simulink model "LKAS_AutoSave_20210315_1628"  (R2018b)
(part 1 of 18)
settings: Solver=FixedStepDiscrete  StartTime=0.0  StopTime=10.0  FixedStep=0.01  RelTol=1e-3
InitFcn:
  | tmpVer = ver('MATLAB');
  | tmpVer = str2num(tmpVer.Version);
  | % -------------------------------------------------------------------
  | %  MATLAB file generated by Simulink.saveVars on 21-Nov-2019 10:06:14
  | %  MATLAB version: 7.13.0.564 (R2011b)
  | % -------------------------------------------------------------------
  | 
  | 
  | SInt16 = Simulink.AliasType;
  | SInt16.Description = 'Num';
  | if (tmpVer > 7.11)
  | 	SInt16.DataScope = 'Auto';
  | end
  | SInt16.HeaderFile = 'Rte_Type.h';
  | SInt16.BaseType = 'int16';
  | 
  | SInt32 = Simulink.AliasType;
  | SInt32.Description = 'Num';
  | if (tmpVer > 7.11)
  | 	SInt32.DataScope = 'Auto';
  | end
  | SInt32.HeaderFile = 'Rte_Type.h';
  | SInt32.BaseType = 'int32';
  | 
  | SInt8 = Simulink.AliasType;
  | SInt8.Description = 'Num';
  | if (tmpVer > 7.11)
  | 	SInt8.DataScope = 'Auto';
  | end
  | SInt8.HeaderFile = 'Rte_Type.h';
  | SInt8.BaseType = 'int8';
  | 
  | T_A_m2_1024_1_u32 = Simulink.NumericType;
  | T_A_m2_1024_1_u32.Description = 'm2 (square meters  (m2))';
  | if (tmpVer > 7.11)
  | 	T_A_m2_1024_1_u32.DataScope = 'Auto';
  | end
  | T_A_m2_1024_1_u32.HeaderFile = 'Rte_Type.h';
  | T_A_m2_1024_1_u32.DataTypeMode = 'Fixed-point: slope and bias scaling';
  | T_A_m2_1024_1_u32.SignednessBool = false;
  | T_A_m2_1024_1_u32.WordLength = 32;
  | T_A_m2_1024_1_u32.FixedExponent = -10;
  | T_A_m2_1024_1_u32.SlopeAdjustmentFactor = 1;
  | T_A_m2_1024_1_u32.Bias = 0;
  | T_A_m2_1024_1_u32.DataTypeOverride = 'Inherit';
  | T_A_m2_1024_1_u32.IsAlias = true;
  | 
  | T_A_m2_65536_1_u16 = Simulink.NumericType;
  | T_A_m2_65536_1_u16.Description = 'm2 (square meters  (m2))';
  | if (tmpVer > 7.11)
  | 	T_A_m2_65536_1_u16.DataScope = 'Auto';
  | end
  | T_A_m2_65536_1_u16.HeaderFile = 'Rte_Type.h';
  | T_A_m2_65536_1_u16.DataTypeMode = 'Fixed-point: slope and bias scaling';
  | T_A_m2_65536_1_u16.SignednessBool = false;
  | T_A_m2_65536_1_u16.WordLength = 16;
  | T_A_m2_65536_1_u16.FixedExponent = -16;
  | T_A_m2_65536_1_u16.SlopeAdjustmentFactor = 1;
  | T_A_m2_65536_1_u16.Bias = 0;
  | T_A_m2_65536_1_u16.DataTypeOverride = 'Inherit';
  | T_A_m2_65536_1_u16.IsAlias = true;
  | 
  | T_A_m2_Float32 = Simulink.NumericType;
  | T_A_m2_Float32.Description = 'm2 (square meters  (m2))';
  | if (tmpVer > 7.11)
  | 	T_A_m2_Float32.DataScope = 'Auto';
  | end
  | T_A_m2_Float32.HeaderFile = 'Rte_Type.h';
  | T_A_m2_Float32.DataTypeMode = 'Single';
  | T_A_m2_Float32.SignednessBool = true;
  | T_A_m2_Float32.WordLength = 32;
  | T_A_m2_Float32.FixedExponent = 0;
  | T_A_m2_Float32.SlopeAdjustmentFactor = 1;
  | T_A_m2_Float32.Bias = 0;
  | T_A_m2_Float32.DataTypeOverride = 'Inherit';
  | T_A_m2_Float32.IsAlias = true;
  | 
  | T_A_mm2_10_1_u16 = Simulink.NumericType;
  | T_A_mm2_10_1_u16.Description = 'mm2 (square millimeters  (mm2))';
  | if (tmpVer > 7.11)
  | 	T_A_mm2_10_1_u16.DataScope = 'Auto';
  | end
  | T_A_mm2_10_1_u16.HeaderFile = 'Rte_Type.h';
  | T_A_mm2_10_1_u16.DataTypeMode = 'Fixed-point: slope and bias scaling';
  | T_A_mm2_10_1_u16.SignednessBool = false;
  | T_A_mm2_10_1_u16.WordLength = 16;
  | T_A_mm2_10_1_u16.FixedExponent = -4;
  | T_A_mm2_10_1_u16.SlopeAdjustmentFactor = 1.6;
  | T_A_mm2_10_1_u16.Bias = 0;
  | T_A_mm2_10_1_u16.DataTypeOverride = 'Inherit';
  | T_A_mm2_10_1_u16.IsAlias = true;
  | 
  | T_A_mm2_4_1_s16 = Simulink.NumericType;
  | T_A_mm2_4_1_s16.Description = 'mm2 (square millimeters  (mm2))';
  | if (tmpVer > 7.11)
  | 	T_A_mm2_4_1_s16.DataScope = 'Auto';
  | end
  | T_A_mm2_4_1_s16.HeaderFile = 'Rte_Type.h';
  | T_A_mm2_4_1_s16.DataTypeMode = 'Fixed-point: slope and bias scaling';
  | T_A_mm2_4_1_s16.SignednessBool = true;
  | T_A_mm2_4_1_s16.WordLength = 16;
  | T_A_mm2_4_1_s16.FixedExponent = -2;
  | T_A_mm2_4_1_s16.SlopeAdjustmentFactor = 1;
  | T_A_mm2_4_1_s16.Bias = 0;
  | T_A_mm2_4_1_s16.DataTypeOverride = 'Inherit';
  | T_A_mm2_4_1_s16.IsAlias = true;
  | 
  | T_A_mm2_Float32 = Simulink.NumericType;
  | T_A_mm2_Float32.Description = 'mm2 (square millimeters  (mm2))';
  | if (tmpVer > 7.11)
  | 	T_A_mm2_Float32.DataScope = 'Auto';
  | end
  | T_A_mm2_Float32.HeaderFile = 'Rte_Type.h';
  | T_A_mm2_Float32.DataTypeMode = 'Single';
  | T_A_mm2_Float32.SignednessBool = true;
  | T_A_mm2_Float32.WordLength = 32;
  | T_A_mm2_Float32.FixedExponent = 0;
  | T_A_mm2_Float32.SlopeAdjustmentFactor = 1;
  | T_A_mm2_Float32.Bias = 0;
  | T_A_mm2_Float32.DataTypeOverride = 'Inherit';
  | T_A_mm2_Float32.IsAlias = true;
  | 
  | T_BOOLEAN = Simulink.AliasType;
  | T_BOOLEAN.Description = 'Bool';
  | if (tmpVer > 7.11)
  | 	T_BOOLEAN.DataScope = 'Auto';
  | end
  | T_BOOLEAN.HeaderFile = 'Rte_Type.h';
  | T_BOOLEAN.BaseType = 'boolean';
  | 
  | T_Cnt_Num_10_1_u32 = Simulink.NumericType;
  | T_Cnt_Num_10_1_u32.Description = 'Num (counts)';
  | if (tmpVer > 7.11)
  | 	T_Cnt_Num_10_1_u32.DataScope = 'Auto';
  | end
  | T_Cnt_Num_10_1_u32.HeaderFile = 'Rte_Type.h';
  | T_Cnt_Num_10_1_u32.DataTypeMode = 'Fixed-point: slope and bias scaling';
  | T_Cnt_Num_10_1_u32.SignednessBool = false;
  | T_Cnt_Num_10_1_u32.WordLength = 32;
  | T_Cnt_Num_10_1_u32.FixedExponent = -4;
  | T_Cnt_Num_10_1_u32.SlopeAdjustmentFactor = 1.6;
  | T_Cnt_Num_10_1_u32.Bias = 0;
  | T_Cnt_Num_10_1_u32.DataTypeOverride = 'Inherit';
  | T_Cnt_Num_10_1_u32.IsAlias = true;
  | 
  | T_Cnt_Num_1_1_s16 = Simulink.NumericType;
  | T_Cnt_Num_1_1_s16.Description = 'Num (counts)';
  | if (tmpVer > 7.11)
  | 	T_Cnt_Num_1_1_s16.DataScope = 'Auto';
  | end
  | T_Cnt_Num_1_1_s16.HeaderFile = 'Rte_Type.h';
  | T_Cnt_Num_1_1_s16.DataTypeMode = 'Fixed-point: slope and bias scaling';
  | T_Cnt_Num_1_1_s16.SignednessBool = true;
  | T_Cnt_Num_1_1_s16.WordLength = 16;
  | T_Cnt_Num_1_1_s16.FixedExponent = 0;
  | T_Cnt_Num_1_1_s16.SlopeAdjustmentFactor = 1;
  | T_Cnt_Num_1_1_s16.Bias = 0;
  | T_Cnt_Num_1_1_s16.DataTypeOverride = 'Inherit';
  | T_Cnt_Num_1_1_s16.IsAlias = true;
  | 
  | T_Cnt_Num_1_1_s32 = Simulink.NumericType;
  | T_Cnt_Num_1_1_s32.Description = 'Num (counts)';
  | if (tmpVer > 7.11)
  | 	T_Cnt_Num_1_1_s32.DataScope = 'Auto';
  | end
  | T_Cnt_Num_1_1_s32.HeaderFile = 'Rte_Type.h';
  | T_Cnt_Num_1_1_s32.DataTypeMode = 'Fixed-point: slope and bias scaling';
  | T_Cnt_Num_1_1_s32.SignednessBool = true;
  | T_Cnt_Num_1_1_s32.WordLength = 32;
  | T_Cnt_Num_1_1_s32.FixedExponent = 0;
  | T_Cnt_Num_1_1_s32.SlopeAdjustmentFactor = 1;
  | T_Cnt_Num_1_1_s32.Bias = 0;
  | T_Cnt_Num_1_1_s32.DataTypeOverride = 'Inherit';
  | T_Cnt_Num_1_1_s32.IsAlias = true;
  | 
  | T_Cnt_Num_1_1_s8 = Simulink.NumericType;
  | T_Cnt_Num_1_1_s8.Description = 'Num (counts)';
  | if (tmpVer > 7.11)
  | 	T_Cnt_Num_1_1_s8.DataScope = 'Auto';
  | end
  | T_Cnt_Num_1_1_s8.HeaderFile = 'Rte_Type.h';
  | T_Cnt_Num_1_1_s8.DataTypeMode = 'Fixed-point: slope and bias scaling';
  | T_Cnt_Num_1_1_s8.SignednessBool = true;
  | T_Cnt_Num_1_1_s8.WordLength = 8;
  | T_Cnt_Num_1_1_s8.FixedExponent = 0;
  | T_Cnt_Num_1_1_s8.SlopeAdjustmentFactor = 1;
  | T_Cnt_Num_1_1_s8.Bias = 0;
  | T_Cnt_Num_1_1_s8.DataTypeOverride = 'Inherit';
  | T_Cnt_Num_1_1_s8.IsAlias = true;
  | 
  | T_Cnt_Num_1_1_u16 = Simulink.NumericType;
  | T_Cnt_Num_1_1_u16.Description = 'Num (counts)';
  | if (tmpVer > 7.11)
  | 	T_Cnt_Num_1_1_u16.DataScope = 'Auto';
  | end
  | T_Cnt_Num_1_1_u16.HeaderFile = 'Rte_Type.h';
  | T_Cnt_Num_1_1_u16.DataTypeMode = 'Fixed-point: slope and bias scaling';
  | T_Cnt_Num_1_1_u16.SignednessBool = false;
  | T_Cnt_Num_1_1_u16.WordLength = 16;
  | T_Cnt_Num_1_1_u16.FixedExponent = 0;
  | T_Cnt_Num_1_1_u16.SlopeAdjustmentFactor = 1;
  | T_Cnt_Num_1_1_u16.Bias = 0;
  | T_Cnt_Num_1_1_u16.DataTypeOverride = 'Inherit';
  | T_Cnt_Num_1_1_u16.IsAlias = true;
  | 
  | T_Cnt_Num_1_1_u32 = Simulink.NumericType;
  | T_Cnt_Num_1_1_u32.Description = 'Num (counts)';
  | if (tmpVer > 7.11)
  | 	T_Cnt_Num_1_1_u32.DataScope = 'Auto';
  | end
  | T_Cnt_Num_1_1_u32.HeaderFile = 'Rte_Type.h';
  | T_Cnt_Num_1_1_u32.DataTypeMode = 'Fixed-point: slope and bias scaling';
  | T_Cnt_Num_1_1_u32.SignednessBool = false;
  | T_Cnt_Num_1_1_u32.WordLength = 32;
  | T_Cnt_Num_1_1_u32.FixedExponent = 0;
  | T_Cnt_Num_1_1_u32.SlopeAdjustmentFactor = 1;
  | T_Cnt_Num_1_1_u32.Bias = 0;
  | T_Cnt_Num_1_1_u32.DataTypeOverride = 'Inherit';
  | T_Cnt_Num_1_1_u32.IsAlias = true;
  | 
  | T_Cnt_Num_1_1_u8 = Simulink.NumericType;
  | T_Cnt_Num_1_1_u8.Description = 'Num (counts)';
  | if (tmpVer > 7.11)
  | 	T_Cnt_Num_1_1_u8.DataScope = 'Auto';
  | end
  | T_Cnt_Num_1_1_u8.HeaderFile = 'Rte_Type.h';
  | T_Cnt_Num_1_1_u8.DataTypeMode = 'Fixed-point: slope and bias scaling';
  | T_Cnt_Num_1_1_u8.SignednessBool = false;
  | T_Cnt_Num_1_1_u8.WordLength = 8;
  | T_Cnt_Num_1_1_u8.FixedExponent = 0;
  | T_Cnt_Num_1_1_u8.SlopeAdjustmentFactor = 1;
  | T_Cnt_Num_1_1_u8.Bias = 0;
  | T_Cnt_Num_1_1_u8.DataTypeOverride = 'Inherit';
  | T_Cnt_Num_1_1_u8.IsAlias = true;
  | 
  | T_E_J_1_1_s32 = Simulink.NumericType;
  | T_E_J_1_1_s32.Description = 'J (joules  (J))';
  | if (tmpVer > 7.11)
  | 	T_E_J_1_1_s32.DataScope = 'Auto';
  | end
  | T_E_J_1_1_s32.HeaderFile = 'Rte_Type.h';
  | T_E_J_1_1_s32.DataTypeMode = 'Fixed-point: slope and bias scaling';
  | T_E_J_1_1_s32.SignednessBool = true;
  | T_E_J_1_1_s32.WordLength = 32;
  | T_E_J_1_1_s32.FixedExponent = 0;
  | T_E_J_1_1_s32.SlopeAdjustmentFactor = 1;
  | T_E_J_1_1_s32.Bias = 0;
  | T_E_J_1_1_s32.DataTypeOverride = 'Inherit';
  | T_E_J_1_1_s32.IsAlias = true;
  | 
  | T_E_J_Float32 = Simulink.NumericType;
  | T_E_J_Float32.Description = 'J (joules  (J))';
  | if (tmpVer > 7.11)
  | 	T_E_J_Float32.DataScope = 'Auto';
  | end
  | T_E_J_Float32.HeaderFile = 'Rte_Type.h';
  | T_E_J_Float32.DataTypeMode = 'Single';
  | T_E_J_Float32.SignednessBool = true;
  | T_E_J_Float32.WordLength = 32;
  | T_E_J_Float32.FixedExponent = 0;
  | T_E_J_Float32.SlopeAdjustmentFactor = 1;
  | T_E_J_Float32.Bias = 0;
  | T_E_J_Float32.DataTypeOverride = 'Inherit';
  | T_E_J_Float32.IsAlias = true;
  | 
  | T_E_kJ_128_1_s32 = Simulink.NumericType;
  | T_E_kJ_128_1_s32.Description = 'kJ (kilojoules  (kJ))';
  | if (tmpVer > 7.11)
  | 	T_E_kJ_128_1_s32.DataScope = 'Auto';
  | end
  | T_E_kJ_128_1_s32.HeaderFile = 'Rte_Type.h';
  | T_E_kJ_128_1_s32.DataTypeMode = 'Fixed-point: slope and bias scaling';
  | T_E_kJ_128_1_s32.SignednessBool = true;
  | T_E_kJ_128_1_s32.WordLength = 32;
  | T_E_kJ_128_1_s32.FixedExponent = -7;
  | T_E_kJ_128_1_s32.SlopeAdjustmentFactor = 1;
  | T_E_kJ_128_1_s32.Bias = 0;
  | T_E_kJ_128_1_s32.DataTypeOverride = 'Inherit';
  | T_E_kJ_128_1_s32.IsAlias = true;
  | 
  | T_E_kJ_Float32 = Simulink.NumericType;
  | T_E_kJ_Float32.Description = 'kJ (kilojoules  (kJ))';
  | if (tmpVer > 7.11)
  | 	T_E_kJ_Float32.DataScope = 'Auto';
  | end
  | T_E_kJ_Float32.HeaderFile = 'Rte_Type.h';
  | T_E_kJ_Float32.DataTypeMode = 'Single';
  | T_E_kJ_Float32.SignednessBool = true;
  | T_E_kJ_Float32.WordLength = 32;
  | T_E_kJ_Float32.FixedExponent = 0;
  | T_E_kJ_Float32.SlopeAdjustmentFactor = 1;
  | T_E_kJ_Float32.Bias = 0;
  | T_E_kJ_Float32.DataTypeOverride = 'Inherit';
  | T_E_kJ_Float32.IsAlias = true;
  | 
  | T_E_kwh_10_1_u16 = Simulink.NumericType;
  | T_E_kwh_10_1_u16.Description = 'kwh (kilowatt-hours (kwh))';
  | if (tmpVer > 7.11)
  | 	T_E_kwh_10_1_u16.DataScope = 'Auto';
  | end
  | T_E_kwh_10_1_u16.HeaderFile = 'Rte_Type.h';
  | T_E_kwh_10_1_u16.DataTypeMode = 'Fixed-point: slope and bias scaling';
  | T_E_kwh_10_1_u16.SignednessBool = false;
  | T_E_kwh_10_1_u16.WordLength = 16;
  | T_E_kwh_10_1_u16.FixedExponent = -4;
  | T_E_kwh_10_1_u16.SlopeAdjustmentFactor = 1.6;
  | T_E_kwh_10_1_u16.Bias = 0;
  | T_E_kwh_10_1_u16.DataTypeOverride = 'Inherit';
  | T_E_kwh_10_1_u16.IsAlias = true;
  | 
  | T_E_kwh_Float32 = Simulink.NumericType;
  | T_E_kwh_Float32.Description = 'kwh (kilowatt-hours (kwh))';
  | if (tmpVer > 7.11)
  | 	T_E_kwh_Float32.DataScope = 'Auto';
  | end
  | T_E_kwh_Float32.HeaderFile = 'Rte_Type.h';
  | T_E_kwh_Float32.DataTypeMode = 'Single';
  | T_E_kwh_Float32.SignednessBool = true;
  | T_E_kwh_Float32.WordLength = 32;
  | T_E_kwh_Float32.FixedExponent = 0;
  | T_E_kwh_Float32.SlopeAdjustmentFactor = 1;
  | T_E_kwh_Float32.Bias = 0;
  | T_E_kwh_Float32.DataTypeOverride = 'Inherit';
  | T_E_kwh_Float32.IsAlias = true;
  | 
  | T_Epl_kwhpkm_100_1_u16 = Simulink.NumericType;
  | T_Epl_kwhpkm_100_1_u16.Description = 'kwhpkm (kwh / 100km  (kwhpkm))';
  | if (tmpVer > 7.11)
  | 	T_Epl_kwhpkm_100_1_u16.DataScope = 'Auto';
  | end
  | T_Epl_kwhpkm_100_1_u16.HeaderFile = 'Rte_Type.h';
  | T_Epl_kwhpkm_100_1_u16.DataTypeMode = ...
  |   'Fixed-point: slope and bias scaling';
  | T_Epl_kwhpkm_100_1_u16.SignednessBool = false;
  | T_Epl_kwhpkm_100_1_u16.WordLength = 16;
  | T_Epl_kwhpkm_100_1_u16.FixedExponent = -7;
  | T_Epl_kwhpkm_100_1_u16.SlopeAdjustmentFactor = 1.28;
  | T_Epl_kwhpkm_100_1_u16.Bias = 0;
  | T_Epl_kwhpkm_100_1_u16.DataTypeOverride = 'Inherit';
  | T_Epl_kwhpkm_100_1_u16.IsAlias = true;
  | 
  | T_Epl_kwhpkm_Float32 = Simulink.NumericType;
  | T_Epl_kwhpkm_Float32.Description = 'kwhpkm (kwh / 100km  (kwhpkm))';
  | if (tmpVer > 7.11)
  | 	T_Epl_kwhpkm_Float32.DataScope = 'Auto';
  | end
  | T_Epl_kwhpkm_Float32.HeaderFile = 'Rte_Type.h';
  | T_Epl_kwhpkm_Float32.DataTypeMode = 'Single';
  | T_Epl_kwhpkm_Float32.SignednessBool = true;
  | T_Epl_kwhpkm_Float32.WordLength = 32;
  | T_Epl_kwhpkm_Float32.FixedExponent = 0;
  | T_Epl_kwhpkm_Float32.SlopeAdjustmentFactor = 1;
  | T_Epl_kwhpkm_Float32.Bias = 0;
  | T_Epl_kwhpkm_Float32.DataTypeOverride = 'Inherit';
  | T_Epl_kwhpkm_Float32.IsAlias = true;
  | 
  | T_F_N_1_1_s16 = Simulink.NumericType;
  | T_F_N_1_1_s16.Description = 'N (newtons  (N))';
  | if (tmpVer > 7.11)
  | 	T_F_N_1_1_s16.DataScope = 'Auto';
  | end
  | T_F_N_1_1_s16.HeaderFile = 'Rte_Type.h';
  | T_F_N_1_1_s16.DataTypeMode = 'Fixed-point: slope and bias scaling';
  | T_F_N_1_1_s16.SignednessBool = true;
  | T_F_N_1_1_s16.WordLength = 16;
  | T_F_N_1_1_s16.FixedExponent = 0;
  | T_F_N_1_1_s16.SlopeAdjustmentFactor = 1;
  | T_F_N_1_1_s16.Bias = 0;
  | T_F_N_1_1_s16.DataTypeOverride = 'Inherit';
  | T_F_N_1_1_s16.IsAlias = true;
  | 
  | T_F_N_Float32 = Simulink.NumericType;
  | T_F_N_Float32.Description = 'N (newtons  (N))';
  | if (tmpVer > 7.11)
  | 	T_F_N_Float32.DataScope = 'Auto';
  | end
  | T_F_N_Float32.HeaderFile = 'Rte_Type.h';
  | T_F_N_Float32.DataTypeMode = 'Single';
  | T_F_N_Float32.SignednessBool = true;
  | T_F_N_Float32.WordLength = 32;
  | T_F_N_Float32.FixedExponent = 0;
  | T_F_N_Float32.SlopeAdjustmentFactor = 1;
  | T_F_N_Float32.Bias = 0;
  | T_F_N_Float32.DataTypeOverride = 'Inherit';
  | T_F_N_Float32.IsAlias = true;
  | 
  | T_I_A_1000_1_u16 = Simulink.NumericType;
  | T_I_A_1000_1_u16.Description = 'A (amperes  (A))';
  | if (tmpVer > 7.11)
  | 	T_I_A_1000_1_u16.DataScope = 'Auto';
  | end
  | T_I_A_1000_1_u16.HeaderFile = 'Rte_Type.h';
  | T_I_A_1000_1_u16.DataTypeMode = 'Fixed-point: slope and bias scaling';
  | T_I_A_1000_1_u16.SignednessBool = false;
  | T_I_A_1000_1_u16.WordLength = 16;
  | T_I_A_1000_1_u16.FixedExponent = -10;
  | T_I_A_1000_1_u16.SlopeAdjustmentFactor = 1.024;
  | T_I_A_1000_1_u16.Bias = 0;
  | T_I_A_1000_1_u16.DataTypeOverride = 'Inherit';
  | T_I_A_1000_1_u16.IsAlias = true;
  | 
  | T_I_A_1048576_1_s32 = Simulink.NumericType;
  | T_I_A_1048576_1_s32.Description = 'A (amperes  (A))';
  | if (tmpVer > 7.11)
  | 	T_I_A_1048576_1_s32.DataScope = 'Auto';
  | end
  | T_I_A_1048576_1_s32.HeaderFile = 'Rte_Type.h';
  | T_I_A_1048576_1_s32.DataTypeMode = ['Fixed-point: slope and bias scalin' ...
  |                                     'g'];
  | T_I_A_1048576_1_s32.SignednessBool = true;
  | T_I_A_1048576_1_s32.WordLength = 32;
  | T_I_A_1048576_1_s32.FixedExponent = -20;
  | T_I_A_1048576_1_s32.SlopeAdjustmentFactor = 1;
  | T_I_A_1048576_1_s32.Bias = 0;
  | T_I_A_1048576_1_s32.DataTypeOverride = 'Inherit';
  | T_I_A_1048576_1_s32.IsAlias = true;
  | 
  | T_I_A_2048_1_s16 = Simulink.NumericType;
  | T_I_A_2048_1_s16.Description = 'A (amperes  (A))';
  | if (tmpVer > 7.11)
  | 	T_I_A_2048_1_s16.DataScope = 'Auto';
  | end
  | T_I_A_2048_1_s16.HeaderFile = 'Rte_Type.h';
  | T_I_A_2048_1_s16.DataTypeMode = 'Fixed-point: slope and bias scaling';
  | T_I_A_2048_1_s16.SignednessBool = true;
  | T_I_A_2048_1_s16.WordLength = 16;
  | T_I_A_2048_1_s16.FixedExponent = -11;
  | T_I_A_2048_1_s16.SlopeAdjustmentFactor = 1;
  | T_I_A_2048_1_s16.Bias = 0;
  | T_I_A_2048_1_s16.DataTypeOverride = 'Inherit';
  | T_I_A_2048_1_s16.IsAlias = true;
  | 
  | T_I_A_32_1_s16 = Simulink.NumericType;
  | T_I_A_32_1_s16.Description = 'A (amperes  (A))';
  | if (tmpVer > 7.11)
  | 	T_I_A_32_1_s16.DataScope = 'Auto';
  | end
  | T_I_A_32_1_s16.HeaderFile = 'Rte_Type.h';
  | T_I_A_32_1_s16.DataTypeMode = 'Fixed-point: slope and bias scaling';
  | T_I_A_32_1_s16.SignednessBool = true;
  | T_I_A_32_1_s16.WordLength = 16;
  | T_I_A_32_1_s16.FixedExponent = -5;
  | T_I_A_32_1_s16.SlopeAdjustmentFactor = 1;
  | T_I_A_32_1_s16.Bias = 0;
  | T_I_A_32_1_s16.DataTypeOverride = 'Inherit';
  | T_I_A_32_1_s16.IsAlias = true;
  | 
  | T_I_A_Float32 = Simulink.NumericType;
  | T_I_A_Float32.Description = 'A (amperes  (A))';
  | if (tmpVer > 7.11)
  | 	T_I_A_Float32.DataScope = 'Auto';
  | end
  | T_I_A_Float32.HeaderFile = 'Rte_Type.h';
  | T_I_A_Float32.DataTypeMode = 'Single';
  | T_I_A_Float32.SignednessBool = true;
  | T_I_A_Float32.WordLength = 32;
  | T_I_A_Float32.FixedExponent = 0;
  | T_I_A_Float32.SlopeAdjustmentFactor = 1;
  | T_I_A_Float32.Bias = 0;
  | T_I_A_Float32.DataTypeOverride = 'Inherit';
  | T_I_A_Float32.IsAlias = true;
  | 
  | T_I_mA_1_1_s16 = Simulink.NumericType;
  | T_I_mA_1_1_s16.Description = 'mA (milliamperes  (mA))';
  | if (tmpVer > 7.11)
  | 	T_I_mA_1_1_s16.DataScope = 'Auto';
  | end
  | T_I_mA_1_1_s16.HeaderFile = 'Rte_Type.h';
  | T_I_mA_1_1_s16.DataTypeMode = 'Fixed-point: slope and bias scaling';
  | T_I_mA_1_1_s16.SignednessBool = true;
  | T_I_mA_1_1_s16.WordLength = 16;
  | T_I_mA_1_1_s16.FixedExponent = 0;
  | T_I_mA_1_1_s16.SlopeAdjustmentFactor = 1;
  | T_I_mA_1_1_s16.Bias = 0;
  | T_I_mA_1_1_s16.DataTypeOverride = 'Inherit';
  | T_I_mA_1_1_s16.IsAlias = true;
  | 
  | T_I_mA_32768_128_s16 = Simulink.NumericType;
  | T_I_mA_32768_128_s16.Description = 'mA (milliamperes  (mA))';
  | if (tmpVer > 7.11)
  | 	T_I_mA_32768_128_s16.DataScope = 'Auto';
  | end
  | T_I_mA_32768_128_s16.HeaderFile = 'Rte_Type.h';
  | T_I_mA_32768_128_s16.DataTypeMode = ...
  |   'Fixed-point: slope and bias scaling';
  | T_I_mA_32768_128_s16.SignednessBool = true;
  | T_I_mA_32768_128_s16.WordLength = 16;
  | T_I_mA_32768_128_s16.FixedExponent = -8;
  | T_I_mA_32768_128_s16.SlopeAdjustmentFactor = 1;
  | T_I_mA_32768_128_s16.Bias = 0;
  | T_I_mA_32768_128_s16.DataTypeOverride = 'Inherit';
  | T_I_mA_32768_128_s16.IsAlias = true;
  | 
  | T_I_mA_Float32 = Simulink.NumericType;
  | T_I_mA_Float32.Description = 'mA (milliamperes  (mA))';
  | if (tmpVer > 7.11)
  | 	T_I_mA_Float32.DataScope = 'Auto';
  | end
  | T_I_mA_Float32.HeaderFile = 'Rte_Type.h';
  | T_I_mA_Float32.DataTypeMode = 'Single';
  | T_I_mA_Float32.SignednessBool = true;
  | T_I_mA_Float32.WordLength = 32;
  | T_I_mA_Float32.FixedExponent = 0;
  | T_I_mA_Float32.SlopeAdjustmentFactor = 1;
  | T_I_mA_Float32.Bias = 0;
  | T_I_mA_Float32.DataTypeOverride = 'Inherit';
  | T_I_mA_Float32.IsAlias = true;
  | 
  | T_J_kgpm2_128_1_u16 = Simulink.NumericType;
  | T_J_kgpm2_128_1_u16.Description = ['kgpm2 (kilograms-square meters  (kg' ...
  |                                    ' m2))'];
  | if (tmpVer > 7.11)
  | 	T_J_kgpm2_128_1_u16.DataScope = 'Auto';
  | end
  | T_J_kgpm2_128_1_u16.HeaderFile = 'Rte_Type.h';
  | T_J_kgpm2_128_1_u16.DataTypeMode = ['Fixed-point: slope and bias scalin' ...
  |                                     'g'];
  | T_J_kgpm2_128_1_u16.SignednessBool = false;
  | T_J_kgpm2_128_1_u16.WordLength = 16;
  | T_J_kgpm2_128_1_u16.FixedExponent = -7;
  | T_J_kgpm2_128_1_u16.SlopeAdjustmentFactor = 1;
  | T_J_kgpm2_128_1_u16.Bias = 0;
  | T_J_kgpm2_128_1_u16.DataTypeOverride = 'Inherit';
  | T_J_kgpm2_128_1_u16.IsAlias = true;
  | 
  | T_J_kgpm2_Float32 = Simulink.NumericType;
  | T_J_kgpm2_Float32.Description = ['kgpm2 (kilograms-square meters  (kg m' ...
  |                                  '2))'];
  | if (tmpVer > 7.11)
  | 	T_J_kgpm2_Float32.DataScope = 'Auto';
  | end
  | T_J_kgpm2_Float32.HeaderFile = 'Rte_Type.h';
  | T_J_kgpm2_Float32.DataTypeMode = 'Single';
  | T_J_kgpm2_Float32.SignednessBool = true;
  | T_J_kgpm2_Float32.WordLength = 32;
  | T_J_kgpm2_Float32.FixedExponent = 0;
  | T_J_kgpm2_Float32.SlopeAdjustmentFactor = 1;
  | T_J_kgpm2_Float32.Bias = 0;
  | T_J_kgpm2_Float32.DataTypeOverride = 'Inherit';
  | T_J_kgpm2_Float32.IsAlias = true;
  | 
  | T_K_NA_1000_1_s16 = Simulink.NumericType;
  | T_K_NA_1000_1_s16.Description = 'NA (dependent upon the gain)';
  | if (tmpVer > 7.11)
  | 	T_K_NA_1000_1_s16.DataScope = 'Auto';
  | end
  | T_K_NA_1000_1_s16.HeaderFile = 'Rte_Type.h';
  | T_K_NA_1000_1_s16.DataTypeMode = 'Fixed-point: slope and bias scaling';
  | T_K_NA_1000_1_s16.SignednessBool = true;
  | T_K_NA_1000_1_s16.WordLength = 16;
  | T_K_NA_1000_1_s16.FixedExponent = -10;
  | T_K_NA_1000_1_s16.SlopeAdjustmentFactor = 1.024;
  | T_K_NA_1000_1_s16.Bias = 0;
  | T_K_NA_1000_1_s16.DataTypeOverride = 'Inherit';
  | T_K_NA_1000_1_s16.IsAlias = true;
  | 
  | T_K_NA_100_1_s16 = Simulink.NumericType;
  | T_K_NA_100_1_s16.Description = 'NA (dependent upon the gain)';
  | if (tmpVer > 7.11)
  | 	T_K_NA_100_1_s16.DataScope = 'Auto';
  | end
  | T_K_NA_100_1_s16.HeaderFile = 'Rte_Type.h';
  | T_K_NA_100_1_s16.DataTypeMode = 'Fixed-point: slope and bias scaling';
  | T_K_NA_100_1_s16.SignednessBool = true;
  | T_K_NA_100_1_s16.WordLength = 16;
  | T_K_NA_100_1_s16.FixedExponent = -7;
  | T_K_NA_100_1_s16.SlopeAdjustmentFactor = 1.28;
  | T_K_NA_100_1_s16.Bias = 0;
  | T_K_NA_100_1_s16.DataTypeOverride = 'Inherit';
  | T_K_NA_100_1_s16.IsAlias = true;
  | 
  | T_K_NA_100_1_u16 = Simulink.NumericType;
  | T_K_NA_100_1_u16.Description = 'NA (dependent upon the gain)';
  | if (tmpVer > 7.11)
  | 	T_K_NA_100_1_u16.DataScope = 'Auto';
  | end
  | T_K_NA_100_1_u16.HeaderFile = 'Rte_Type.h';
  | T_K_NA_100_1_u16.DataTypeMode = 'Fixed-point: slope and bias scaling';
  | T_K_NA_100_1_u16.SignednessBool = false;
  | T_K_NA_100_1_u16.WordLength = 16;
  | T_K_NA_100_1_u16.FixedExponent = -7;
  | T_K_NA_100_1_u16.SlopeAdjustmentFactor = 1.28;
  | T_K_NA_100_1_u16.Bias = 0;
  | T_K_NA_100_1_u16.DataTypeOverride = 'Inherit';
  | T_K_NA_100_1_u16.IsAlias = true;
  | 
  | T_K_NA_1024_1_s16 = Simulink.NumericType;
  | T_K_NA_1024_1_s16.Description = 'NA (dependent upon the gain)';
  | if (tmpVer > 7.11)
  | 	T_K_NA_1024_1_s16.DataScope = 'Auto';
  | end
  | T_K_NA_1024_1_s16.HeaderFile = 'Rte_Type.h';
  | T_K_NA_1024_1_s16.DataTypeMode = 'Fixed-point: slope and bias scaling';
  | T_K_NA_1024_1_s16.SignednessBool = true;
  | T_K_NA_1024_1_s16.WordLength = 16;
  | T_K_NA_1024_1_s16.FixedExponent = -10;
  | T_K_NA_1024_1_s16.SlopeAdjustmentFactor = 1;
  | T_K_NA_1024_1_s16.Bias = 0;
  | T_K_NA_1024_1_s16.DataTypeOverride = 'Inherit';
  | T_K_NA_1024_1_s16.IsAlias = true;
  | 
  | T_K_NA_1024_1_u16 = Simulink.NumericType;
  | T_K_NA_1024_1_u16.Description = 'NA (dependent upon the gain)';
  | if (tmpVer > 7.11)
  | 	T_K_NA_1024_1_u16.DataScope = 'Auto';
  | end
  | T_K_NA_1024_1_u16.HeaderFile = 'Rte_Type.h';
  | T_K_NA_1024_1_u16.DataTypeMode = 'Fixed-point: slope and bias scaling';
  | T_K_NA_1024_1_u16.SignednessBool = false;
  | T_K_NA_1024_1_u16.WordLength = 16;
  | T_K_NA_1024_1_u16.FixedExponent = -10;
  | T_K_NA_1024_1_u16.SlopeAdjustmentFactor = 1;
  | T_K_NA_1024_1_u16.Bias = 0;
  | T_K_NA_1024_1_u16.DataTypeOverride = 'Inherit';
  | T_K_NA_1024_1_u16.IsAlias = true;
  | 
  | T_K_NA_128_1_s16 = Simulink.NumericType;
  | T_K_NA_128_1_s16.Description = 'NA (dependent upon the gain)';
  | if (tmpVer > 7.11)
  | 	T_K_NA_128_1_s16.DataScope = 'Auto';
  | end
  | T_K_NA_128_1_s16.HeaderFile = 'Rte_Type.h';
  | T_K_NA_128_1_s16.DataTypeMode = 'Fixed-point: slope and bias scaling';
  | T_K_NA_128_1_s16.SignednessBool = true;
  | T_K_NA_128_1_s16.WordLength = 16;
  | T_K_NA_128_1_s16.FixedExponent = -7;
  | T_K_NA_128_1_s16.SlopeAdjustmentFactor = 1;
  | T_K_NA_128_1_s16.Bias = 0;
  | T_K_NA_128_1_s16.DataTypeOverride = 'Inherit';
  | T_K_NA_128_1_s16.IsAlias = true;
  | 
  | T_K_NA_128_1_u16 = Simulink.NumericType;
  | T_K_NA_128_1_u16.Description = 'NA (dependent upon the gain)';
  | if (tmpVer > 7.11)
  | 	T_K_NA_128_1_u16.DataScope = 'Auto';
  | end
  | T_K_NA_128_1_u16.HeaderFile = 'Rte_Type.h';
  | T_K_NA_128_1_u16.DataTypeMode = 'Fixed-point: slope and bias scaling';
  | T_K_NA_128_1_u16.SignednessBool = false;
  | T_K_NA_128_1_u16.WordLength = 16;
  | T_K_NA_128_1_u16.FixedExponent = -7;
  | T_K_NA_128_1_u16.SlopeAdjustmentFactor = 1;
  | T_K_NA_128_1_u16.Bias = 0;
  | T_K_NA_128_1_u16.DataTypeOverride = 'Inherit';
  | T_K_NA_128_1_u16.IsAlias = true;
  | 
  | T_K_NA_128_1_u8 = Simulink.NumericType;
  | T_K_NA_128_1_u8.Description = 'NA (dependent upon the gain)';
  | if (tmpVer > 7.11)
  | 	T_K_NA_128_1_u8.DataScope = 'Auto';
  | end
  | T_K_NA_128_1_u8.HeaderFile = 'Rte_Type.h';
  | T_K_NA_128_1_u8.DataTypeMode = 'Fixed-point: slope and bias scaling';
  | T_K_NA_128_1_u8.SignednessBool = false;
  | T_K_NA_128_1_u8.WordLength = 8;
  | T_K_NA_128_1_u8.FixedExponent = -7;
  | T_K_NA_128_1_u8.SlopeAdjustmentFactor = 1;
  | T_K_NA_128_1_u8.Bias = 0;
  | T_K_NA_128_1_u8.DataTypeOverride = 'Inherit';
  | T_K_NA_128_1_u8.IsAlias = true;
  | 
  | T_K_NA_16777216_1_u32 = Simulink.NumericType;
  | T_K_NA_16777216_1_u32.Description = 'NA (dependent upon the gain)';
  | if (tmpVer > 7.11)
  | 	T_K_NA_16777216_1_u32.DataScope = 'Auto';
  | end
  | T_K_NA_16777216_1_u32.HeaderFile = 'Rte_Type.h';
  | T_K_NA_16777216_1_u32.DataTypeMode = ...
  |   'Fixed-point: slope and bias scaling';
  | T_K_NA_16777216_1_u32.SignednessBool = false;
  | T_K_NA_16777216_1_u32.WordLength = 32;
  | T_K_NA_16777216_1_u32.FixedExponent = -24;
  | T_K_NA_16777216_1_u32.SlopeAdjustmentFactor = 1;
  | T_K_NA_16777216_1_u32.Bias = 0;
  | T_K_NA_16777216_1_u32.DataTypeOverride = 'Inherit';
  | T_K_NA_16777216_1_u32.IsAlias = true;
  | 
  | T_K_NA_16_1_s16 = Simulink.NumericType;
  | T_K_NA_16_1_s16.Description = 'NA (dependent upon the gain)';
  | if (tmpVer > 7.11)
  | 	T_K_NA_16_1_s16.DataScope = 'Auto';
  | end
  | T_K_NA_16_1_s16.HeaderFile = 'Rte_Type.h';
  | T_K_NA_16_1_s16.DataTypeMode = 'Fixed-point: slope and bias scaling';
  | T_K_NA_16_1_s16.SignednessBool = true;
  | T_K_NA_16_1_s16.WordLength = 16;
  | T_K_NA_16_1_s16.FixedExponent = -4;
  | T_K_NA_16_1_s16.SlopeAdjustmentFactor = 1;
  | T_K_NA_16_1_s16.Bias = 0;
  | T_K_NA_16_1_s16.DataTypeOverride = 'Inherit';
  | T_K_NA_16_1_s16.IsAlias = true;
  | 
  | T_K_NA_16_1_u16 = Simulink.NumericType;
  | T_K_NA_16_1_u16.Description = 'NA (dependent upon the gain)';
  | if (tmpVer > 7.11)
  | 	T_K_NA_16_1_u16.DataScope = 'Auto';
  | end
  | T_K_NA_16_1_u16.HeaderFile = 'Rte_Type.h';
  | T_K_NA_16_1_u16.DataTypeMode = 'Fixed-point: slope and bias scaling';
  | T_K_NA_16_1_u16.SignednessBool = false;
  | T_K_NA_16_1_u16.WordLength = 16;
  | T_K_NA_16_1_u16.FixedExponent = -4;
  | T_K_NA_16_1_u16.SlopeAdjustmentFactor = 1;
  | T_K_NA_16_1_u16.Bias = 0;
  | T_K_NA_16_1_u16.DataTypeOverride = 'Inherit';
  | T_K_NA_16_1_u16.IsAlias = true;
  | 
  | T_K_NA_16_1_u8 = Simulink.NumericType;
  | T_K_NA_16_1_u8.Description = 'NA (dependent upon the gain)';
  | if (tmpVer > 7.11)
  | 	T_K_NA_16_1_u8.DataScope = 'Auto';
  | end
  | T_K_NA_16_1_u8.HeaderFile = 'Rte_Type.h';
  | T_K_NA_16_1_u8.DataTypeMode = 'Fixed-point: slope and bias scaling';
  | T_K_NA_16_1_u8.SignednessBool = false;
  | T_K_NA_16_1_u8.WordLength = 8;
  | T_K_NA_16_1_u8.FixedExponent = -4;
  | T_K_NA_16_1_u8.SlopeAdjustmentFactor = 1;
  | T_K_NA_16_1_u8.Bias = 0;
  | T_K_NA_16_1_u8.DataTypeOverride = 'Inherit';
  | T_K_NA_16_1_u8.IsAlias = true;
  | 
  | T_K_NA_1_16_u16 = Simulink.NumericType;
  | T_K_NA_1_16_u16.Description = 'NA (dependent upon the gain)';
  | if (tmpVer > 7.11)
  | 	T_K_NA_1_16_u16.DataScope = 'Auto';
  | end
  | T_K_NA_1_16_u16.HeaderFile = 'Rte_Type.h';
  | T_K_NA_1_16_u16.DataTypeMode = 'Fixed-point: slope and bias scaling';
  | T_K_NA_1_16_u16.SignednessBool = false;
  | T_K_NA_1_16_u16.WordLength = 16;
  | T_K_NA_1_16_u16.FixedExponent = 4;
  | T_K_NA_1_16_u16.SlopeAdjustmentFactor = 1;
  | T_K_NA_1_16_u16.Bias = 0;
  | T_K_NA_1_16_u16.DataTypeOverride = 'Inherit';
  | T_K_NA_1_16_u16.IsAlias = true;
  | 
  | T_K_NA_1_1_s16 = Simulink.NumericType;
  | T_K_NA_1_1_s16.Description = 'NA (dependent upon the gain)';
  | if (tmpVer > 7.11)
  | 	T_K_NA_1_1_s16.DataScope = 'Auto';
  | end
  | T_K_NA_1_1_s16.HeaderFile = 'Rte_Type.h';
  | T_K_NA_1_1_s16.DataTypeMode = 'Fixed-point: slope and bias scaling';
  | T_K_NA_1_1_s16.SignednessBool = true;
  | T_K_NA_1_1_s16.WordLength = 16;
  | T_K_NA_1_1_s16.FixedExponent = 0;
  | T_K_NA_1_1_s16.SlopeAdjustmentFactor = 1;
  | T_K_NA_1_1_s16.Bias = 0;
  | T_K_NA_1_1_s16.DataTypeOverride = 'Inherit';
  | T_K_NA_1_1_s16.IsAlias = true;
  | 
  | T_K_NA_1_1_u16 = Simulink.NumericType;
  | T_K_NA_1_1_u16.Description = 'NA (dependent upon the gain)';
  | if (tmpVer > 7.11)
  | 	T_K_NA_1_1_u16.DataScope = 'Auto';
  | end
  | T_K_NA_1_1_u16.HeaderFile = 'Rte_Type.h';
  | T_K_NA_1_1_u16.DataTypeMode = 'Fixed-point: slope and bias scaling';
  | T_K_NA_1_1_u16.SignednessBool = false;
  | T_K_NA_1_1_u16.WordLength = 16;
  | T_K_NA_1_1_u16.FixedExponent = 0;
  | T_K_NA_1_1_u16.SlopeAdjustmentFactor = 1;
  | T_K_NA_1_1_u16.Bias = 0;
  | T_K_NA_1_1_u16.DataTypeOverride = 'Inherit';
  | T_K_NA_1_1_u16.IsAlias = true;
  | 
  | T_K_NA_1_1_u8 = Simulink.NumericType;
  | T_K_NA_1_1_u8.Description = 'NA (dependent upon the gain)';
  | if (tmpVer > 7.11)
  | 	T_K_NA_1_1_u8.DataScope = 'Auto';
  | end
  | T_K_NA_1_1_u8.HeaderFile = 'Rte_Type.h';
  | T_K_NA_1_1_u8.DataTypeMode = 'Fixed-point: slope and bias scaling';
  | T_K_NA_1_1_u8.SignednessBool = false;
  | T_K_NA_1_1_u8.WordLength = 8;
  | T_K_NA_1_1_u8.FixedExponent = 0;
  | T_K_NA_1_1_u8.SlopeAdjustmentFactor = 1;
  | T_K_NA_1_1_u8.Bias = 0;
  | T_K_NA_1_1_u8.DataTypeOverride = 'Inherit';
  | T_K_NA_1_1_u8.IsAlias = true;
  | 
  | T_K_NA_32768_1_s16 = Simulink.NumericType;
  | T_K_NA_32768_1_s16.Description = 'NA (dependent upon the gain)';
  | if (tmpVer > 7.11)
  | 	T_K_NA_32768_1_s16.DataScope = 'Auto';
  | end
  | T_K_NA_32768_1_s16.HeaderFile = 'Rte_Type.h';
  | T_K_NA_32768_1_s16.DataTypeMode = 'Fixed-point: slope and bias scaling';
  | T_K_NA_32768_1_s16.SignednessBool = true;
  | T_K_NA_32768_1_s16.WordLength = 16;
  | T_K_NA_32768_1_s16.FixedExponent = -15;
  | T_K_NA_32768_1_s16.SlopeAdjustmentFactor = 1;
  | T_K_NA_32768_1_s16.Bias = 0;
  | T_K_NA_32768_1_s16.DataTypeOverride = 'Inherit';
  | T_K_NA_32768_1_s16.IsAlias = true;
  | 
  | T_K_NA_32768_1_u16 = Simulink.NumericType;
  | T_K_NA_32768_1_u16.Description = 'NA (dependent upon the gain)';
  | if (tmpVer > 7.11)
  | 	T_K_NA_32768_1_u16.DataScope = 'Auto';
  | end
  | T_K_NA_32768_1_u16.HeaderFile = 'Rte_Type.h';
  | T_K_NA_32768_1_u16.DataTypeMode = 'Fixed-point: slope and bias scaling';
  | T_K_NA_32768_1_u16.SignednessBool = false;
  | T_K_NA_32768_1_u16.WordLength = 16;
  | T_K_NA_32768_1_u16.FixedExponent = -15;
  | T_K_NA_32768_1_u16.SlopeAdjustmentFactor = 1;
  | T_K_NA_32768_1_u16.Bias = 0;
  | T_K_NA_32768_1_u16.DataTypeOverride = 'Inherit';
  | T_K_NA_32768_1_u16.IsAlias = true;
  | 
  | T_K_NA_32_1_s8 = Simulink.NumericType;
  | T_K_NA_32_1_s8.Description = 'NA (dependent upon the gain)';
  | if (tmpVer > 7.11)
  | 	T_K_NA_32_1_s8.DataScope = 'Auto';
  | end
  | T_K_NA_32_1_s8.HeaderFile = 'Rte_Type.h';
  | T_K_NA_32_1_s8.DataTypeMode = 'Fixed-point: slope and bias scaling';
  | T_K_NA_32_1_s8.SignednessBool = true;
  | T_K_NA_32_1_s8.WordLength = 8;
  | T_K_NA_32_1_s8.FixedExponent = -5;
  | T_K_NA_32_1_s8.SlopeAdjustmentFactor = 1;
  | T_K_NA_32_1_s8.Bias = 0;
  | T_K_NA_32_1_s8.DataTypeOverride = 'Inherit';
  | T_K_NA_32_1_s8.IsAlias = true;
  | 
  | T_K_NA_4096_1_u16 = Simulink.NumericType;
  | T_K_NA_4096_1_u16.Description = 'NA (dependent upon the gain)';
  | if (tmpVer > 7.11)
  | 	T_K_NA_4096_1_u16.DataScope = 'Auto';
  | end
  | T_K_NA_4096_1_u16.HeaderFile = 'Rte_Type.h';
  | T_K_NA_4096_1_u16.DataTypeMode = 'Fixed-point: slope and bias scaling';
  | T_K_NA_4096_1_u16.SignednessBool = false;
  | T_K_NA_4096_1_u16.WordLength = 16;
  | T_K_NA_4096_1_u16.FixedExponent = -12;
  | T_K_NA_4096_1_u16.SlopeAdjustmentFactor = 1;
  | T_K_NA_4096_1_u16.Bias = 0;
  | T_K_NA_4096_1_u16.DataTypeOverride = 'Inherit';
  | T_K_NA_4096_1_u16.IsAlias = true;
  | 
  | T_K_NA_4194304_1_s32 = Simulink.NumericType;
  | T_K_NA_4194304_1_s32.Description = 'NA (dependent upon the gain)';
  | if (tmpVer > 7.11)
  | 	T_K_NA_4194304_1_s32.DataScope = 'Auto';
  | end
  | T_K_NA_4194304_1_s32.HeaderFile = 'Rte_Type.h';
  | T_K_NA_4194304_1_s32.DataTypeMode = ...
  |   'Fixed-point: slope and bias scaling';
  | T_K_NA_4194304_1_s32.SignednessBool = true;
  | T_K_NA_4194304_1_s32.WordLength = 32;
  | T_K_NA_4194304_1_s32.FixedExponent = -22;
  | T_K_NA_4194304_1_s32.SlopeAdjustmentFactor = 1;
  | T_K_NA_4194304_1_s32.Bias = 0;
  | T_K_NA_4194304_1_s32.DataTypeOverride = 'Inherit';
  | T_K_NA_4194304_1_s32.IsAlias = true;
  | 
  | T_K_NA_4194304_1_u16 = Simulink.NumericType;
  | T_K_NA_4194304_1_u16.Description = 'NA (dependent upon the gain)';
  | if (tmpVer > 7.11)
  | 	T_K_NA_4194304_1_u16.DataScope = 'Auto';
  | end
  | T_K_NA_4194304_1_u16.HeaderFile = 'Rte_Type.h';
  | T_K_NA_4194304_1_u16.DataTypeMode = ...
  |   'Fixed-point: slope and bias scaling';
  | T_K_NA_4194304_1_u16.SignednessBool = false;
  | T_K_NA_4194304_1_u16.WordLength = 16;
  | T_K_NA_4194304_1_u16.FixedExponent = -22;
  | T_K_NA_4194304_1_u16.SlopeAdjustmentFactor = 1;
  | T_K_NA_4194304_1_u16.Bias = 0;
  | T_K_NA_4194304_1_u16.DataTypeOverride = 'Inherit';
  | T_K_NA_4194304_1_u16.IsAlias = true;
  | 
  | T_K_NA_65536_1_s32 = Simulink.NumericType;
  | T_K_NA_65536_1_s32.Description = 'NA (dependent upon the gain)';
  | if (tmpVer > 7.11)
  | 	T_K_NA_65536_1_s32.DataScope = 'Auto';
  | end
  | T_K_NA_65536_1_s32.HeaderFile = 'Rte_Type.h';
  | T_K_NA_65536_1_s32.DataTypeMode = 'Fixed-point: slope and bias scaling';
  | T_K_NA_65536_1_s32.SignednessBool = true;
  | T_K_NA_65536_1_s32.WordLength = 32;
  | T_K_NA_65536_1_s32.FixedExponent = -16;
  | T_K_NA_65536_1_s32.SlopeAdjustmentFactor = 1;
  | T_K_NA_65536_1_s32.Bias = 0;
  | T_K_NA_65536_1_s32.DataTypeOverride = 'Inherit';
  | T_K_NA_65536_1_s32.IsAlias = true;
  | 
  | T_K_NA_65536_1_u16 = Simulink.NumericType;
  | T_K_NA_65536_1_u16.Description = 'NA (dependent upon the gain)';
  | if (tmpVer > 7.11)
  | 	T_K_NA_65536_1_u16.DataScope = 'Auto';
  | end
  | T_K_NA_65536_1_u16.HeaderFile = 'Rte_Type.h';
  | T_K_NA_65536_1_u16.DataTypeMode = 'Fixed-point: slope and bias scaling';
  | T_K_NA_65536_1_u16.SignednessBool = false;
  | T_K_NA_65536_1_u16.WordLength = 16;
  | T_K_NA_65536_1_u16.FixedExponent = -16;
  | T_K_NA_65536_1_u16.SlopeAdjustmentFactor = 1;
  | T_K_NA_65536_1_u16.Bias = 0;
  | T_K_NA_65536_1_u16.DataTypeOverride = 'Inherit';
  | T_K_NA_65536_1_u16.IsAlias = true;
  | 
  | T_K_NA_8192_1_s16 = Simulink.NumericType;
  | T_K_NA_8192_1_s16.Description = 'NA (dependent upon the gain)';
  | if (tmpVer > 7.11)
  | 	T_K_NA_8192_1_s16.DataScope = 'Auto';
  | end
  | T_K_NA_8192_1_s16.HeaderFile = 'Rte_Type.h';
  | T_K_NA_8192_1_s16.DataTypeMode = 'Fixed-point: slope and bias scaling';
  | T_K_NA_8192_1_s16.SignednessBool = true;
  | T_K_NA_8192_1_s16.WordLength = 16;
  | T_K_NA_8192_1_s16.FixedExponent = -13;
  | T_K_NA_8192_1_s16.SlopeAdjustmentFactor = 1;
  | T_K_NA_8192_1_s16.Bias = 0;
  | T_K_NA_8192_1_s16.DataTypeOverride = 'Inherit';
  | T_K_NA_8192_1_s16.IsAlias = true;
  | 
  | T_K_NA_8_1_s16 = Simulink.NumericType;
  | T_K_NA_8_1_s16.Description = 'NA (dependent upon the gain)';
  | if (tmpVer > 7.11)
  | 	T_K_NA_8_1_s16.DataScope = 'Auto';
  | end
  | T_K_NA_8_1_s16.HeaderFile = 'Rte_Type.h';
  | T_K_NA_8_1_s16.DataTypeMode = 'Fixed-point: slope and bias scaling';
  | T_K_NA_8_1_s16.SignednessBool = true;
  | T_K_NA_8_1_s16.WordLength = 16;
  | T_K_NA_8_1_s16.FixedExponent = -3;
  | T_K_NA_8_1_s16.SlopeAdjustmentFactor = 1;
  | T_K_NA_8_1_s16.Bias = 0;
  | T_K_NA_8_1_s16.DataTypeOverride = 'Inherit';
  | T_K_NA_8_1_s16.IsAlias = true;
  | 
  | T_K_NA_Float32 = Simulink.NumericType;
  | T_K_NA_Float32.Description = 'NA (dependent upon the gain)';
  | if (tmpVer > 7.11)
  | 	T_K_NA_Float32.DataScope = 'Auto';
  | end
  | T_K_NA_Float32.HeaderFile = 'Rte_Type.h';
  | T_K_NA_Float32.DataTypeMode = 'Single';
  | T_K_NA_Float32.SignednessBool = true;
  | T_K_NA_Float32.WordLength = 32;
  | T_K_NA_Float32.FixedExponent = 0;
  | T_K_NA_Float32.SlopeAdjustmentFactor = 1;
  | T_K_NA_Float32.Bias = 0;
  | T_K_NA_Float32.DataTypeOverride = 'Inherit';
  | T_K_NA_Float32.IsAlias = true;
  | 
  | T_M_Nm_16_1_s16 = Simulink.NumericType;
  | T_M_Nm_16_1_s16.Description = 'Nm (newton-meters  (Nm))';
  | if (tmpVer > 7.11)
  | 	T_M_Nm_16_1_s16.DataScope = 'Auto';
  | end
  | T_M_Nm_16_1_s16.HeaderFile = 'Rte_Type.h';
  | T_M_Nm_16_1_s16.DataTypeMode = 'Fixed-point: slope and bias scaling';
  | T_M_Nm_16_1_s16.SignednessBool = true;
  | T_M_Nm_16_1_s16.WordLength = 16;
  | T_M_Nm_16_1_s16.FixedExponent = -4;
  | T_M_Nm_16_1_s16.SlopeAdjustmentFactor = 1;
  | T_M_Nm_16_1_s16.Bias = 0;
  | T_M_Nm_16_1_s16.DataTypeOverride = 'Inherit';
  | T_M_Nm_16_1_s16.IsAlias = true;
  | 
  | T_M_Nm_1_1_s16 = Simulink.NumericType;
  | T_M_Nm_1_1_s16.Description = 'Nm (newton-meters  (Nm))';
  | if (tmpVer > 7.11)
  | 	T_M_Nm_1_1_s16.DataScope = 'Auto';
  | end
  | T_M_Nm_1_1_s16.HeaderFile = 'Rte_Type.h';
  | T_M_Nm_1_1_s16.DataTypeMode = 'Fixed-point: slope and bias scaling';
  | T_M_Nm_1_1_s16.SignednessBool = true;
  | T_M_Nm_1_1_s16.WordLength = 16;
  | T_M_Nm_1_1_s16.FixedExponent = 0;
  | T_M_Nm_1_1_s16.SlopeAdjustmentFactor = 1;
  | T_M_Nm_1_1_s16.Bias = 0;
  | T_M_Nm_1_1_s16.DataTypeOverride = 'Inherit';
  | T_M_Nm_1_1_s16.IsAlias = true;
  | 
  | T_M_Nm_32768_1_s16 = Simulink.NumericType;
  | T_M_Nm_32768_1_s16.Description = 'Nm (newton-meters  (Nm))';
  | if (tmpVer > 7.11)
  | 	T_M_Nm_32768_1_s16.DataScope = 'Auto';
  | end
  | T_M_Nm_32768_1_s16.HeaderFile = 'Rte_Type.h';
  | T_M_Nm_32768_1_s16.DataTypeMode = 'Fixed-point: slope and bias scaling';
  | T_M_Nm_32768_1_s16.SignednessBool = true;
  | T_M_Nm_32768_1_s16.WordLength = 16;
  | T_M_Nm_32768_1_s16.FixedExponent = -15;
  | T_M_Nm_32768_1_s16.SlopeAdjustmentFactor = 1;
  | T_M_Nm_32768_1_s16.Bias = 0;
  | T_M_Nm_32768_1_s16.DataTypeOverride = 'Inherit';
  | T_M_Nm_32768_1_s16.IsAlias = true;
  | 
  | T_M_Nm_32_1_s16 = Simulink.NumericType;
  | T_M_Nm_32_1_s16.Description = 'Nm (newton-meters  (Nm))';
  | if (tmpVer > 7.11)
  | 	T_M_Nm_32_1_s16.DataScope = 'Auto';
  | end
  | T_M_Nm_32_1_s16.HeaderFile = 'Rte_Type.h';
  | T_M_Nm_32_1_s16.DataTypeMode = 'Fixed-point: slope and bias scaling';
  | T_M_Nm_32_1_s16.SignednessBool = true;
  | T_M_Nm_32_1_s16.WordLength = 16;
  | T_M_Nm_32_1_s16.FixedExponent = -5;
  | T_M_Nm_32_1_s16.SlopeAdjustmentFactor = 1;
  | T_M_Nm_32_1_s16.Bias = 0;
  | T_M_Nm_32_1_s16.DataTypeOverride = 'Inherit';
  | T_M_Nm_32_1_s16.IsAlias = true;
  | 
  | T_M_Nm_4_1_s16 = Simulink.NumericType;
  | T_M_Nm_4_1_s16.Description = 'Nm (newton-meters  (Nm))';
  | if (tmpVer > 7.11)
  | 	T_M_Nm_4_1_s16.DataScope = 'Auto';
  | end
  | T_M_Nm_4_1_s16.HeaderFile = 'Rte_Type.h';
  | T_M_Nm_4_1_s16.DataTypeMode = 'Fixed-point: slope and bias scaling';
  | T_M_Nm_4_1_s16.SignednessBool = true;
  | T_M_Nm_4_1_s16.WordLength = 16;
  | T_M_Nm_4_1_s16.FixedExponent = -2;
  | T_M_Nm_4_1_s16.SlopeAdjustmentFactor = 1;
  | T_M_Nm_4_1_s16.Bias = 0;
  | T_M_Nm_4_1_s16.DataTypeOverride = 'Inherit';
  | T_M_Nm_4_1_s16.IsAlias = true;
  | 
  | T_M_Nm_512_1_s16 = Simulink.NumericType;
  | T_M_Nm_512_1_s16.Description = 'Nm (newton-meters  (Nm))';
  | if (tmpVer > 7.11)
  | 	T_M_Nm_512_1_s16.DataScope = 'Auto';
  | end
  | T_M_Nm_512_1_s16.HeaderFile = 'Rte_Type.h';
  | T_M_Nm_512_1_s16.DataTypeMode = 'Fixed-point: slope and bias scaling';
  | T_M_Nm_512_1_s16.SignednessBool = true;
  | T_M_Nm_512_1_s16.WordLength = 16;
  | T_M_Nm_512_1_s16.FixedExponent = -9;
  | T_M_Nm_512_1_s16.SlopeAdjustmentFactor = 1;
  | T_M_Nm_512_1_s16.Bias = 0;
  | T_M_Nm_512_1_s16.DataTypeOverride = 'Inherit';
  | T_M_Nm_512_1_s16.IsAlias = true;
  | 
  | T_M_Nm_Float32 = Simulink.NumericType;
  | T_M_Nm_Float32.Description = 'Nm (newton-meters  (Nm))';
  | if (tmpVer > 7.11)
  | 	T_M_Nm_Float32.DataScope = 'Auto';
  | end
  | T_M_Nm_Float32.HeaderFile = 'Rte_Type.h';
  | T_M_Nm_Float32.DataTypeMode = 'Single';
  | T_M_Nm_Float32.SignednessBool = true;
  | T_M_Nm_Float32.WordLength = 32;
  | T_M_Nm_Float32.FixedExponent = 0;
  | T_M_Nm_Float32.SlopeAdjustmentFactor = 1;
  | T_M_Nm_Float32.Bias = 0;
  | T_M_Nm_Float32.DataTypeOverride = 'Inherit';
  | T_M_Nm_Float32.IsAlias = true;
  | 
  | T_P_W_1_4_s16 = Simulink.NumericType;
  | T_P_W_1_4_s16.Description = 'W (watts  (W))';
  | if (tmpVer > 7.11)
  | 	T_P_W_1_4_s16.DataScope = 'Auto';
  | end
  | T_P_W_1_4_s16.HeaderFile = 'Rte_Type.h';
  | T_P_W_1_4_s16.DataTypeMode = 'Fixed-point: slope and bias scaling';
  | T_P_W_1_4_s16.SignednessBool = true;
  | T_P_W_1_4_s16.WordLength = 16;
  | T_P_W_1_4_s16.FixedExponent = 2;
  | T_P_W_1_4_s16.SlopeAdjustmentFactor = 1;
  | T_P_W_1_4_s16.Bias = 0;
  | T_P_W_1_4_s16.DataTypeOverride = 'Inherit';
  | T_P_W_1_4_s16.IsAlias = true;
  | 
  | T_P_W_1_8_s16 = Simulink.NumericType;
  | T_P_W_1_8_s16.Description = 'W (watts  (W))';
  | if (tmpVer > 7.11)
  | 	T_P_W_1_8_s16.DataScope = 'Auto';
  | end
  | T_P_W_1_8_s16.HeaderFile = 'Rte_Type.h';
  | T_P_W_1_8_s16.DataTypeMode = 'Fixed-point: slope and bias scaling';
  | T_P_W_1_8_s16.SignednessBool = true;
  | T_P_W_1_8_s16.WordLength = 16;
  | T_P_W_1_8_s16.FixedExponent = 3;
  | T_P_W_1_8_s16.SlopeAdjustmentFactor = 1;
  | T_P_W_1_8_s16.Bias = 0;
  | T_P_W_1_8_s16.DataTypeOverride = 'Inherit';
  | T_P_W_1_8_s16.IsAlias = true;
  | 
  | T_P_W_Float32 = Simulink.NumericType;
  | T_P_W_Float32.Description = 'W (watts  (W))';
  | if (tmpVer > 7.11)
  | 	T_P_W_Float32.DataScope = 'Auto';
  | end
  | T_P_W_Float32.HeaderFile = 'Rte_Type.h';
  | T_P_W_Float32.DataTypeMode = 'Single';
  | T_P_W_Float32.SignednessBool = true;
  | T_P_W_Float32.WordLength = 32;
  | T_P_W_Float32.FixedExponent = 0;
  | T_P_W_Float32.SlopeAdjustmentFactor = 1;
  | T_P_W_Float32.Bias = 0;
  | T_P_W_Float32.DataTypeOverride = 'Inherit';
  | T_P_W_Float32.IsAlias = true;
  | 
  | T_P_kW_128_1_s16 = Simulink.NumericType;
  | T_P_kW_128_1_s16.Description = 'kW (kilowatts  (kW))';
  | if (tmpVer > 7.11)
  | 	T_P_kW_128_1_s16.DataScope = 'Auto';
  | end
  | T_P_kW_128_1_s16.HeaderFile = 'Rte_Type.h';
  | T_P_kW_128_1_s16.DataTypeMode = 'Fixed-point: slope and bias scaling';
  | T_P_kW_128_1_s16.SignednessBool = true;
  | T_P_kW_128_1_s16.WordLength = 16;
  | T_P_kW_128_1_s16.FixedExponent = -7;
  | T_P_kW_128_1_s16.SlopeAdjustmentFactor = 1;
  | T_P_kW_128_1_s16.Bias = 0;
  | T_P_kW_128_1_s16.DataTypeOverride = 'Inherit';
  | T_P_kW_128_1_s16.IsAlias = true;
  | 
  | T_P_kW_1_8_s16 = Simulink.NumericType;
  | T_P_kW_1_8_s16.Description = 'kW (kilowatts  (kW))';
  | if (tmpVer > 7.11)
  | 	T_P_kW_1_8_s16.DataScope = 'Auto';
  | end
  | T_P_kW_1_8_s16.HeaderFile = 'Rte_Type.h';
  | T_P_kW_1_8_s16.DataTypeMode = 'Fixed-point: slope and bias scaling';
  | T_P_kW_1_8_s16.SignednessBool = true;
  | T_P_kW_1_8_s16.WordLength = 16;
  | T_P_kW_1_8_s16.FixedExponent = 3;
  | T_P_kW_1_8_s16.SlopeAdjustmentFactor = 1;
  | T_P_kW_1_8_s16.Bias = 0;
  | T_P_kW_1_8_s16.DataTypeOverride = 'Inherit';
  | T_P_kW_1_8_s16.IsAlias = true;
  | 
  | T_P_kW_8_1_s32 = Simulink.NumericType;
  | T_P_kW_8_1_s32.Description = 'kW (kilowatts  (kW))';
  | if (tmpVer > 7.11)
  | 	T_P_kW_8_1_s32.DataScope = 'Auto';
  | end
  | T_P_kW_8_1_s32.HeaderFile = 'Rte_Type.h';
  | T_P_kW_8_1_s32.DataTypeMode = 'Fixed-point: slope and bias scaling';
  | T_P_kW_8_1_s32.SignednessBool = true;
  | T_P_kW_8_1_s32.WordLength = 32;
  | T_P_kW_8_1_s32.FixedExponent = -3;
  | T_P_kW_8_1_s32.SlopeAdjustmentFactor = 1;
  | T_P_kW_8_1_s32.Bias = 0;
  | T_P_kW_8_1_s32.DataTypeOverride = 'Inherit';
  | T_P_kW_8_1_s32.IsAlias = true;
  | 
  | T_P_kW_Float32 = Simulink.NumericType;
  | T_P_kW_Float32.Description = 'kW (kilowatts  (kW))';
  | if (tmpVer > 7.11)
  | 	T_P_kW_Float32.DataScope = 'Auto';
  | end
  | T_P_kW_Float32.HeaderFile = 'Rte_Type.h';
  | T_P_kW_Float32.DataTypeMode = 'Single';
  | T_P_kW_Float32.SignednessBool = true;
  | T_P_kW_Float32.WordLength = 32;
  | T_P_kW_Float32.FixedExponent = 0;
  | T_P_kW_Float32.SlopeAdjustmentFactor = 1;
  | T_P_kW_Float32.Bias = 0;
  | T_P_kW_Float32.DataTypeOverride = 'Inherit';
  | T_P_kW_Float32.IsAlias = true;
  | 
  | T_Pct_pct_1024_1_s32 = Simulink.NumericType;
  | T_Pct_pct_1024_1_s32.Description = 'pct (percent  (%))';
  | if (tmpVer > 7.11)
  | 	T_Pct_pct_1024_1_s32.DataScope = 'Auto';
  | end
  | T_Pct_pct_1024_1_s32.HeaderFile = 'Rte_Type.h';
  | T_Pct_pct_1024_1_s32.DataTypeMode = ...
  |   'Fixed-point: slope and bias scaling';
  | T_Pct_pct_1024_1_s32.SignednessBool = true;
  | T_Pct_pct_1024_1_s32.WordLength = 32;
  | T_Pct_pct_1024_1_s32.FixedExponent = -10;
  | T_Pct_pct_1024_1_s32.SlopeAdjustmentFactor = 1;
  | T_Pct_pct_1024_1_s32.Bias = 0;
  | T_Pct_pct_1024_1_s32.DataTypeOverride = 'Inherit';
  | T_Pct_pct_1024_1_s32.IsAlias = true;
  | 
  | T_Pct_pct_1024_1_u32 = Simulink.NumericType;
  | T_Pct_pct_1024_1_u32.Description = 'pct (percent  (%))';
  | if (tmpVer > 7.11)
  | 	T_Pct_pct_1024_1_u32.DataScope = 'Auto';
  | end
  | T_Pct_pct_1024_1_u32.HeaderFile = 'Rte_Type.h';
  | T_Pct_pct_1024_1_u32.DataTypeMode = ...
  |   'Fixed-point: slope and bias scaling';
  | T_Pct_pct_1024_1_u32.SignednessBool = false;
  | T_Pct_pct_1024_1_u32.WordLength = 32;
  | T_Pct_pct_1024_1_u32.FixedExponent = -10;
  | T_Pct_pct_1024_1_u32.SlopeAdjustmentFactor = 1;
  | T_Pct_pct_1024_1_u32.Bias = 0;
  | T_Pct_pct_1024_1_u32.DataTypeOverride = 'Inherit';
  | T_Pct_pct_1024_1_u32.IsAlias = true;
  | 
  | T_Pct_pct_10_1_s16 = Simulink.NumericType;
  | T_Pct_pct_10_1_s16.Description = 'pct (percent  (%))';
  | if (tmpVer > 7.11)
  | 	T_Pct_pct_10_1_s16.DataScope = 'Auto';
  | end
  | T_Pct_pct_10_1_s16.HeaderFile = 'Rte_Type.h';
  | T_Pct_pct_10_1_s16.DataTypeMode = 'Fixed-point: slope and bias scaling';
  | T_Pct_pct_10_1_s16.SignednessBool = true;
  | T_Pct_pct_10_1_s16.WordLength = 16;
  | T_Pct_pct_10_1_s16.FixedExponent = -4;
  | T_Pct_pct_10_1_s16.SlopeAdjustmentFactor = 1.6;
  | T_Pct_pct_10_1_s16.Bias = 0;
  | T_Pct_pct_10_1_s16.DataTypeOverride = 'Inherit';
  | T_Pct_pct_10_1_s16.IsAlias = true;
  | 
  | T_Pct_pct_10_1_u32 = Simulink.NumericType;
  | T_Pct_pct_10_1_u32.Description = 'pct (percent  (%))';
  | if (tmpVer > 7.11)
  | 	T_Pct_pct_10_1_u32.DataScope = 'Auto';
  | end
  | T_Pct_pct_10_1_u32.HeaderFile = 'Rte_Type.h';
  | T_Pct_pct_10_1_u32.DataTypeMode = 'Fixed-point: slope and bias scaling';
  | T_Pct_pct_10_1_u32.SignednessBool = false;
  | T_Pct_pct_10_1_u32.WordLength = 32;
  | T_Pct_pct_10_1_u32.FixedExponent = -4;
  | T_Pct_pct_10_1_u32.SlopeAdjustmentFactor = 1.6;
  | T_Pct_pct_10_1_u32.Bias = 0;
  | T_Pct_pct_10_1_u32.DataTypeOverride = 'Inherit';
  | T_Pct_pct_10_1_u32.IsAlias = true;
  | 
  | T_Pct_pct_128_100_s8 = Simulink.NumericType;
  | T_Pct_pct_128_100_s8.Description = 'pct (percent  (%))';
  | if (tmpVer > 7.11)
  | 	T_Pct_pct_128_100_s8.DataScope = 'Auto';
  | end
  | T_Pct_pct_128_100_s8.HeaderFile = 'Rte_Type.h';
  | T_Pct_pct_128_100_s8.DataTypeMode = ...
  |   'Fixed-point: slope and bias scaling';
  | T_Pct_pct_128_100_s8.SignednessBool = true;
  | T_Pct_pct_128_100_s8.WordLength = 8;
  | T_Pct_pct_128_100_s8.FixedExponent = -1;
  | T_Pct_pct_128_100_s8.SlopeAdjustmentFactor = 1.5625;
  | T_Pct_pct_128_100_s8.Bias = 0;
  | T_Pct_pct_128_100_s8.DataTypeOverride = 'Inherit';
  | T_Pct_pct_128_100_s8.IsAlias = true;
  | 
  | T_Pct_pct_1_1_s16 = Simulink.NumericType;
  | T_Pct_pct_1_1_s16.Description = 'pct (percent  (%))';
  | if (tmpVer > 7.11)
  | 	T_Pct_pct_1_1_s16.DataScope = 'Auto';
  | end
  | T_Pct_pct_1_1_s16.HeaderFile = 'Rte_Type.h';
  | T_Pct_pct_1_1_s16.DataTypeMode = 'Fixed-point: slope and bias scaling';
  | T_Pct_pct_1_1_s16.SignednessBool = true;
  | T_Pct_pct_1_1_s16.WordLength = 16;
  | T_Pct_pct_1_1_s16.FixedExponent = 0;
  | T_Pct_pct_1_1_s16.SlopeAdjustmentFactor = 1;
  | T_Pct_pct_1_1_s16.Bias = 0;
  | T_Pct_pct_1_1_s16.DataTypeOverride = 'Inherit';
  | T_Pct_pct_1_1_s16.IsAlias = true;
  | 
  | T_Pct_pct_1_4_u8 = Simulink.NumericType;
  | T_Pct_pct_1_4_u8.Description = 'pct (percent  (%))';
  | if (tmpVer > 7.11)
  | 	T_Pct_pct_1_4_u8.DataScope = 'Auto';
  | end
  | T_Pct_pct_1_4_u8.HeaderFile = 'Rte_Type.h';
  | T_Pct_pct_1_4_u8.DataTypeMode = 'Fixed-point: slope and bias scaling';
  | T_Pct_pct_1_4_u8.SignednessBool = false;
  | T_Pct_pct_1_4_u8.WordLength = 8;
  | T_Pct_pct_1_4_u8.FixedExponent = 2;
  | T_Pct_pct_1_4_u8.SlopeAdjustmentFactor = 1;
  | T_Pct_pct_1_4_u8.Bias = 0;
  | T_Pct_pct_1_4_u8.DataTypeOverride = 'Inherit';
  | T_Pct_pct_1_4_u8.IsAlias = true;
  | 
  | T_Pct_pct_255_100_u16 = Simulink.NumericType;
  | T_Pct_pct_255_100_u16.Description = 'pct (percent  (%))';
  | if (tmpVer > 7.11)
  | 	T_Pct_pct_255_100_u16.DataScope = 'Auto';
  | end
  | T_Pct_pct_255_100_u16.HeaderFile = 'Rte_Type.h';
  | T_Pct_pct_255_100_u16.DataTypeMode = ...
  |   'Fixed-point: slope and bias scaling';
  | T_Pct_pct_255_100_u16.SignednessBool = false;
  | T_Pct_pct_255_100_u16.WordLength = 16;
  | T_Pct_pct_255_100_u16.FixedExponent = -2;
  | T_Pct_pct_255_100_u16.SlopeAdjustmentFactor = 1.5686274509803921;
  | T_Pct_pct_255_100_u16.Bias = 0;
  | T_Pct_pct_255_100_u16.DataTypeOverride = 'Inherit';
  | T_Pct_pct_255_100_u16.IsAlias = true;
  | 
  | T_Pct_pct_255_100_u8 = Simulink.NumericType;
  | T_Pct_pct_255_100_u8.Description = 'pct (percent  (%))';
  | if (tmpVer > 7.11)
  | 	T_Pct_pct_255_100_u8.DataScope = 'Auto';
  | end
  | T_Pct_pct_255_100_u8.HeaderFile = 'Rte_Type.h';
  | T_Pct_pct_255_100_u8.DataTypeMode = ...
  |   'Fixed-point: slope and bias scaling';
  | T_Pct_pct_255_100_u8.SignednessBool = false;
  | T_Pct_pct_255_100_u8.WordLength = 8;
  | T_Pct_pct_255_100_u8.FixedExponent = -2;
  | T_Pct_pct_255_100_u8.SlopeAdjustmentFactor = 1.5686274509803921;
  | T_Pct_pct_255_100_u8.Bias = 0;
  | T_Pct_pct_255_100_u8.DataTypeOverride = 'Inherit';
  | T_Pct_pct_255_100_u8.IsAlias = true;
  | 
  | T_Pct_pct_256_1_s16 = Simulink.NumericType;
  | T_Pct_pct_256_1_s16.Description = 'pct (percent  (%))';
  | if (tmpVer > 7.11)
  | 	T_Pct_pct_256_1_s16.DataScope = 'Auto';
  | end
  | T_Pct_pct_256_1_s16.HeaderFile = 'Rte_Type.h';
  | T_Pct_pct_256_1_s16.DataTypeMode = ['Fixed-point: slope and bias scalin' ...
  |                                     'g'];
  | T_Pct_pct_256_1_s16.SignednessBool = true;
  | T_Pct_pct_256_1_s16.WordLength = 16;
  | T_Pct_pct_256_1_s16.FixedExponent = -8;
  | T_Pct_pct_256_1_s16.SlopeAdjustmentFactor = 1;
  | T_Pct_pct_256_1_s16.Bias = 0;
  | T_Pct_pct_256_1_s16.DataTypeOverride = 'Inherit';
  | T_Pct_pct_256_1_s16.IsAlias = true;
  | 
  | T_Pct_pct_256_1_u16 = Simulink.NumericType;
  | T_Pct_pct_256_1_u16.Description = 'pct (percent  (%))';
  | if (tmpVer > 7.11)
  | 	T_Pct_pct_256_1_u16.DataScope = 'Auto';
  | end
  | T_Pct_pct_256_1_u16.HeaderFile = 'Rte_Type.h';
  | T_Pct_pct_256_1_u16.DataTypeMode = ['Fixed-point: slope and bias scalin' ...
  |                                     'g'];
  | T_Pct_pct_256_1_u16.SignednessBool = false;
  | T_Pct_pct_256_1_u16.WordLength = 16;
  | T_Pct_pct_256_1_u16.FixedExponent = -8;
  | T_Pct_pct_256_1_u16.SlopeAdjustmentFactor = 1;
  | T_Pct_pct_256_1_u16.Bias = 0;
  | T_Pct_pct_256_1_u16.DataTypeOverride = 'Inherit';
  | T_Pct_pct_256_1_u16.IsAlias = true;
  | 
  | T_Pct_pct_65535_100_u16 = Simulink.NumericType;
  | T_Pct_pct_65535_100_u16.Description = 'pct (percent  (%))';
  | if (tmpVer > 7.11)
  | 	T_Pct_pct_65535_100_u16.DataScope = 'Auto';
  | end
  | T_Pct_pct_65535_100_u16.HeaderFile = 'Rte_Type.h';
  | T_Pct_pct_65535_100_u16.DataTypeMode = ...
  |   'Fixed-point: slope and bias scaling';
  | T_Pct_pct_65535_100_u16.SignednessBool = false;
  | T_Pct_pct_65535_100_u16.WordLength = 16;
  | T_Pct_pct_65535_100_u16.FixedExponent = -10;
  | T_Pct_pct_65535_100_u16.SlopeAdjustmentFactor = 1.5625238422217136;
  | T_Pct_pct_65535_100_u16.Bias = 0;
  | T_Pct_pct_65535_100_u16.DataTypeOverride = 'Inherit';
  | T_Pct_pct_65535_100_u16.IsAlias = true;
  | 
  | T_Pct_pct_Float32 = Simulink.NumericType;
  | T_Pct_pct_Float32.Description = 'pct (percent  (%))';
  | if (tmpVer > 7.11)
  | 	T_Pct_pct_Float32.DataScope = 'Auto';
  | end
  | T_Pct_pct_Float32.HeaderFile = 'Rte_Type.h';
  | T_Pct_pct_Float32.DataTypeMode = 'Single';
  | T_Pct_pct_Float32.SignednessBool = true;
  | T_Pct_pct_Float32.WordLength = 32;
  | T_Pct_pct_Float32.FixedExponent = 0;
  | T_Pct_pct_Float32.SlopeAdjustmentFactor = 1;
  | T_Pct_pct_Float32.Bias = 0;
  | T_Pct_pct_Float32.DataTypeOverride = 'Inherit';
  | T_Pct_pct_Float32.IsAlias = true;
  | 
  | T_R_ohm_1024_1_s16 = Simulink.NumericType;
  | T_R_ohm_1024_1_s16.Description = 'ohm (ohms  (ohm))';
  | if (tmpVer > 7.11)
  | 	T_R_ohm_1024_1_s16.DataScope = 'Auto';
  | end
  | T_R_ohm_1024_1_s16.HeaderFile = 'Rte_Type.h';
  | T_R_ohm_1024_1_s16.DataTypeMode = 'Fixed-point: slope and bias scaling';
  | T_R_ohm_1024_1_s16.SignednessBool = true;
  | T_R_ohm_1024_1_s16.WordLength = 16;
  | T_R_ohm_1024_1_s16.FixedExponent = -10;
  | T_R_ohm_1024_1_s16.SlopeAdjustmentFactor = 1;
  | T_R_ohm_1024_1_s16.Bias = 0;
  | T_R_ohm_1024_1_s16.DataTypeOverride = 'Inherit';
  | T_R_ohm_1024_1_s16.IsAlias = true;
  | 
  | T_R_ohm_32_1_s16 = Simulink.NumericType;
  | T_R_ohm_32_1_s16.Description = 'ohm (ohms  (ohm))';
  | if (tmpVer > 7.11)
  | 	T_R_ohm_32_1_s16.DataScope = 'Auto';
  | end
  | T_R_ohm_32_1_s16.HeaderFile = 'Rte_Type.h';
  | T_R_ohm_32_1_s16.DataTypeMode = 'Fixed-point: slope and bias scaling';
  | T_R_ohm_32_1_s16.SignednessBool = true;
  | T_R_ohm_32_1_s16.WordLength = 16;
  | T_R_ohm_32_1_s16.FixedExponent = -5;
  | T_R_ohm_32_1_s16.SlopeAdjustmentFactor = 1;
  | T_R_ohm_32_1_s16.Bias = 0;
  | T_R_ohm_32_1_s16.DataTypeOverride = 'Inherit';
  | T_R_ohm_32_1_s16.IsAlias = true;
  | 
  | T_R_ohm_Float32 = Simulink.NumericType;
  | T_R_ohm_Float32.Description = 'ohm (ohms  (ohm))';
  | if (tmpVer > 7.11)
  | 	T_R_ohm_Float32.DataScope = 'Auto';
  | end
  | T_R_ohm_Float32.HeaderFile = 'Rte_Type.h';
  | T_R_ohm_Float32.DataTypeMode = 'Single';
  | T_R_ohm_Float32.SignednessBool = true;
  | T_R_ohm_Float32.WordLength = 32;
  | T_R_ohm_Float32.FixedExponent = 0;
  | T_R_ohm_Float32.SlopeAdjustmentFactor = 1;
  | T_R_ohm_Float32.Bias = 0;
  | T_R_ohm_Float32.DataTypeOverride = 'Inherit';
  | T_R_ohm_Float32.IsAlias = true;
  | 
  | T_TK_K_16_1_s16 = Simulink.NumericType;
  | T_TK_K_16_1_s16.Description = 'K (Kelvin  (K))';
  | if (tmpVer > 7.11)
  | 	T_TK_K_16_1_s16.DataScope = 'Auto';
  | end
  | T_TK_K_16_1_s16.HeaderFile = 'Rte_Type.h';
  | T_TK_K_16_1_s16.DataTypeMode = 'Fixed-point: slope and bias scaling';
  | T_TK_K_16_1_s16.SignednessBool = true;
  | T_TK_K_16_1_s16.WordLength = 16;
  | T_TK_K_16_1_s16.FixedExponent = -4;
  | T_TK_K_16_1_s16.SlopeAdjustmentFactor = 1;
  | T_TK_K_16_1_s16.Bias = 0;
  | T_TK_K_16_1_s16.DataTypeOverride = 'Inherit';
  | T_TK_K_16_1_s16.IsAlias = true;
  | 
  | T_TK_K_Float32 = Simulink.NumericType;
  | T_TK_K_Float32.Description = 'K (Kelvin  (K))';
  | if (tmpVer > 7.11)
  | 	T_TK_K_Float32.DataScope = 'Auto';
  | end
  | T_TK_K_Float32.HeaderFile = 'Rte_Type.h';
  | T_TK_K_Float32.DataTypeMode = 'Single';
  | T_TK_K_Float32.SignednessBool = true;
  | T_TK_K_Float32.WordLength = 32;
  | T_TK_K_Float32.FixedExponent = 0;
  | T_TK_K_Float32.SlopeAdjustmentFactor = 1;
  | T_TK_K_Float32.Bias = 0;
  | T_TK_K_Float32.DataTypeOverride = 'Inherit';
  | T_TK_K_Float32.IsAlias = true;
  | 
  | T_T_degC_10_400_1_u16 = Simulink.NumericType;
  | T_T_degC_10_400_1_u16.Description = 'degC (degrees Celsius  (deg C))';
  | if (tmpVer > 7.11)
  | 	T_T_degC_10_400_1_u16.DataScope = 'Auto';
  | end
  | T_T_degC_10_400_1_u16.HeaderFile = 'Rte_Type.h';
  | T_T_degC_10_400_1_u16.DataTypeMode = ...
  |   'Fixed-point: slope and bias scaling';
  | T_T_degC_10_400_1_u16.SignednessBool = false;
  | T_T_degC_10_400_1_u16.WordLength = 16;
  | T_T_degC_10_400_1_u16.FixedExponent = -4;
  | T_T_degC_10_400_1_u16.SlopeAdjustmentFactor = 1.6;
  | T_T_degC_10_400_1_u16.Bias = -40;
  | T_T_degC_10_400_1_u16.DataTypeOverride = 'Inherit';
  | T_T_degC_10_400_1_u16.IsAlias = true;
  | 
  | T_T_degC_16_1_s16 = Simulink.NumericType;
  | T_T_degC_16_1_s16.Description = 'degC (degrees Celsius  (deg C))';
  | if (tmpVer > 7.11)
  | 	T_T_degC_16_1_s16.DataScope = 'Auto';
  | end
  | T_T_degC_16_1_s16.HeaderFile = 'Rte_Type.h';
  | T_T_degC_16_1_s16.DataTypeMode = 'Fixed-point: slope and bias scaling';
  | T_T_degC_16_1_s16.SignednessBool = true;
  | T_T_degC_16_1_s16.WordLength = 16;
  | T_T_degC_16_1_s16.FixedExponent = -4;
  | T_T_degC_16_1_s16.SlopeAdjustmentFactor = 1;
  | T_T_degC_16_1_s16.Bias = 0;
  | T_T_degC_16_1_s16.DataTypeOverride = 'Inherit';
  | T_T_degC_16_1_s16.IsAlias = true;
  | 
  | T_T_degC_1_40_1_u8 = Simulink.NumericType;
  | T_T_degC_1_40_1_u8.Description = 'degC (degrees Celsius  (deg C))';
  | if (tmpVer > 7.11)
  | 	T_T_degC_1_40_1_u8.DataScope = 'Auto';
  | end
  | T_T_degC_1_40_1_u8.HeaderFile = 'Rte_Type.h';
  | T_T_degC_1_40_1_u8.DataTypeMode = 'Fixed-point: slope and bias scaling';
  | T_T_degC_1_40_1_u8.SignednessBool = false;
  | T_T_degC_1_40_1_u8.WordLength = 8;
  | T_T_degC_1_40_1_u8.FixedExponent = 0;
  | T_T_degC_1_40_1_u8.SlopeAdjustmentFactor = 1;
  | T_T_degC_1_40_1_u8.Bias = -40;
  | T_T_degC_1_40_1_u8.DataTypeOverride = 'Inherit';
  | T_T_degC_1_40_1_u8.IsAlias = true;
  | 
  | T_T_degC_2_80_1_u8 = Simulink.NumericType;
  | T_T_degC_2_80_1_u8.Description = 'degC (degrees Celsius  (deg C))';
  | if (tmpVer > 7.11)
  | 	T_T_degC_2_80_1_u8.DataScope = 'Auto';
  | end
  | T_T_degC_2_80_1_u8.HeaderFile = 'Rte_Type.h';
  | T_T_degC_2_80_1_u8.DataTypeMode = 'Fixed-point: slope and bias scaling';
  | T_T_degC_2_80_1_u8.SignednessBool = false;
  | T_T_degC_2_80_1_u8.WordLength = 8;
  | T_T_degC_2_80_1_u8.FixedExponent = -1;
  | T_T_degC_2_80_1_u8.SlopeAdjustmentFactor = 1;
  | T_T_degC_2_80_1_u8.Bias = -40;
  | T_T_degC_2_80_1_u8.DataTypeOverride = 'Inherit';
  | T_T_degC_2_80_1_u8.IsAlias = true;
  | 
  | T_T_degC_Float32 = Simulink.NumericType;
  | T_T_degC_Float32.Description = 'degC (degrees Celsius  (deg C))';
  | if (tmpVer > 7.11)
  | 	T_T_degC_Float32.DataScope = 'Auto';
  | end
  | T_T_degC_Float32.HeaderFile = 'Rte_Type.h';
  | T_T_degC_Float32.DataTypeMode = 'Single';
  | T_T_degC_Float32.SignednessBool = true;
  | T_T_degC_Float32.WordLength = 32;
  | T_T_degC_Float32.FixedExponent = 0;
  | T_T_degC_Float32.SlopeAdjustmentFactor = 1;
  | T_T_degC_Float32.Bias = 0;
  | T_T_degC_Float32.DataTypeOverride = 'Inherit';
  | T_T_degC_Float32.IsAlias = true;
  | 
  | T_U_V_1000_1_u16 = Simulink.NumericType;
  | T_U_V_1000_1_u16.Description = 'V (volts  (V))';
  | if (tmpVer > 7.11)
  | 	T_U_V_1000_1_u16.DataScope = 'Auto';
  | end
  | T_U_V_1000_1_u16.HeaderFile = 'Rte_Type.h';
  | T_U_V_1000_1_u16.DataTypeMode = 'Fixed-point: slope and bias scaling';
  | T_U_V_1000_1_u16.SignednessBool = false;
  | T_U_V_1000_1_u16.WordLength = 16;
  | T_U_V_1000_1_u16.FixedExponent = -10;
  | T_U_V_1000_1_u16.SlopeAdjustmentFactor = 1.024;
  | T_U_V_1000_1_u16.Bias = 0;
  | T_U_V_1000_1_u16.DataTypeOverride = 'Inherit';
  | T_U_V_1000_1_u16.IsAlias = true;
  | 
  | T_U_V_10_1_u8 = Simulink.NumericType;
  | T_U_V_10_1_u8.Description = 'V (volts  (V))';
  | if (tmpVer > 7.11)
  | 	T_U_V_10_1_u8.DataScope = 'Auto';
  | end
  | T_U_V_10_1_u8.HeaderFile = 'Rte_Type.h';
  | T_U_V_10_1_u8.DataTypeMode = 'Fixed-point: slope and bias scaling';
  | T_U_V_10_1_u8.SignednessBool = false;
  | T_U_V_10_1_u8.WordLength = 8;
  | T_U_V_10_1_u8.FixedExponent = -4;
  | T_U_V_10_1_u8.SlopeAdjustmentFactor = 1.6;
  | T_U_V_10_1_u8.Bias = 0;
  | T_U_V_10_1_u8.DataTypeOverride = 'Inherit';
  | T_U_V_10_1_u8.IsAlias = true;
  | 
  | T_U_V_200_1_u8 = Simulink.NumericType;
  | T_U_V_200_1_u8.Description = 'V (volts  (V))';
  | if (tmpVer > 7.11)
  | 	T_U_V_200_1_u8.DataScope = 'Auto';
  | end
  | T_U_V_200_1_u8.HeaderFile = 'Rte_Type.h';
  | T_U_V_200_1_u8.DataTypeMode = 'Fixed-point: slope and bias scaling';
  | T_U_V_200_1_u8.SignednessBool = false;
  | T_U_V_200_1_u8.WordLength = 8;
  | T_U_V_200_1_u8.FixedExponent = -8;
  | T_U_V_200_1_u8.SlopeAdjustmentFactor = 1.28;
  | T_U_V_200_1_u8.Bias = 0;
  | T_U_V_200_1_u8.DataTypeOverride = 'Inherit';
  | T_U_V_200_1_u8.IsAlias = true;
  | 
  | T_U_V_32_1_s16 = Simulink.NumericType;
  | T_U_V_32_1_s16.Description = 'V (volts  (V))';
  | if (tmpVer > 7.11)
  | 	T_U_V_32_1_s16.DataScope = 'Auto';
  | end
  | T_U_V_32_1_s16.HeaderFile = 'Rte_Type.h';
  | T_U_V_32_1_s16.DataTypeMode = 'Fixed-point: slope and bias scaling';
  | T_U_V_32_1_s16.SignednessBool = true;
  | T_U_V_32_1_s16.WordLength = 16;
  | T_U_V_32_1_s16.FixedExponent = -5;
  | T_U_V_32_1_s16.SlopeAdjustmentFactor = 1;
  | T_U_V_32_1_s16.Bias = 0;
  | T_U_V_32_1_s16.DataTypeOverride = 'Inherit';
  | T_U_V_32_1_s16.IsAlias = true;
  | 
  | T_U_V_4096_1_s16 = Simulink.NumericType;
  | T_U_V_4096_1_s16.Description = 'V (volts  (V))';
  | if (tmpVer > 7.11)
  | 	T_U_V_4096_1_s16.DataScope = 'Auto';
  | end
  | T_U_V_4096_1_s16.HeaderFile = 'Rte_Type.h';
  | T_U_V_4096_1_s16.DataTypeMode = 'Fixed-point: slope and bias scaling';
  | T_U_V_4096_1_s16.SignednessBool = true;
  | T_U_V_4096_1_s16.WordLength = 16;
  | T_U_V_4096_1_s16.FixedExponent = -12;
  | T_U_V_4096_1_s16.SlopeAdjustmentFactor = 1;
  | T_U_V_4096_1_s16.Bias = 0;
  | T_U_V_4096_1_s16.DataTypeOverride = 'Inherit';
  | T_U_V_4096_1_s16.IsAlias = true;
  | 
  | T_U_V_512_1_s16 = Simulink.NumericType;
  | T_U_V_512_1_s16.Description = 'V (volts  (V))';
  | if (tmpVer > 7.11)
  | 	T_U_V_512_1_s16.DataScope = 'Auto';
  | end
  | T_U_V_512_1_s16.HeaderFile = 'Rte_Type.h';
  | T_U_V_512_1_s16.DataTypeMode = 'Fixed-point: slope and bias scaling';
  | T_U_V_512_1_s16.SignednessBool = true;
  | T_U_V_512_1_s16.WordLength = 16;
  | T_U_V_512_1_s16.FixedExponent = -9;
  | T_U_V_512_1_s16.SlopeAdjustmentFactor = 1;
  | T_U_V_512_1_s16.Bias = 0;
  | T_U_V_512_1_s16.DataTypeOverride = 'Inherit';
  | T_U_V_512_1_s16.IsAlias = true;
  | 
  | T_U_V_65535_8_u16 = Simulink.NumericType;
  | T_U_V_65535_8_u16.Description = 'V (volts  (V))';
  | if (tmpVer > 7.11)
  | 	T_U_V_65535_8_u16.DataScope = 'Auto';
  | end
  | T_U_V_65535_8_u16.HeaderFile = 'Rte_Type.h';
  | T_U_V_65535_8_u16.DataTypeMode = 'Fixed-point: slope and bias scaling';
  | T_U_V_65535_8_u16.SignednessBool = false;
  | T_U_V_65535_8_u16.WordLength = 16;
  | T_U_V_65535_8_u16.FixedExponent = -13;
  | T_U_V_65535_8_u16.SlopeAdjustmentFactor = 1.0000152590218967;
  | T_U_V_65535_8_u16.Bias = 0;
  | T_U_V_65535_8_u16.DataTypeOverride = 'Inherit';
  | T_U_V_65535_8_u16.IsAlias = true;
  | 
  | T_U_V_8192_1_u16 = Simulink.NumericType;
  | T_U_V_8192_1_u16.Description = 'V (volts  (V))';
  | if (tmpVer > 7.11)
  | 	T_U_V_8192_1_u16.DataScope = 'Auto';
  | end
  | T_U_V_8192_1_u16.HeaderFile = 'Rte_Type.h';
  | T_U_V_8192_1_u16.DataTypeMode = 'Fixed-point: slope and bias scaling';
  | T_U_V_8192_1_u16.SignednessBool = false;
  | T_U_V_8192_1_u16.WordLength = 16;
  | T_U_V_8192_1_u16.FixedExponent = -13;
  | T_U_V_8192_1_u16.SlopeAdjustmentFactor = 1;
  | T_U_V_8192_1_u16.Bias = 0;
  | T_U_V_8192_1_u16.DataTypeOverride = 'Inherit';
  | T_U_V_8192_1_u16.IsAlias = true;
  | 
  | T_U_V_Float32 = Simulink.NumericType;
  | T_U_V_Float32.Description = 'V (volts  (V))';
  | if (tmpVer > 7.11)
  | 	T_U_V_Float32.DataScope = 'Auto';
  | end
  | T_U_V_Float32.HeaderFile = 'Rte_Type.h';
  | T_U_V_Float32.DataTypeMode = 'Single';
  | T_U_V_Float32.SignednessBool = true;
  | T_U_V_Float32.WordLength = 32;
  | T_U_V_Float32.FixedExponent = 0;
  | T_U_V_Float32.SlopeAdjustmentFactor = 1;
  | T_U_V_Float32.Bias = 0;
  | T_U_V_Float32.DataTypeOverride = 'Inherit';
  | T_U_V_Float32.IsAlias = true;
  | 
  | T_U_mV_1_1_s16 = Simulink.NumericType;
  | T_U_mV_1_1_s16.Description = 'mV (millivolts  (mV))';
  | if (tmpVer > 7.11)
  | 	T_U_mV_1_1_s16.DataScope = 'Auto';
  | end
  | T_U_mV_1_1_s16.HeaderFile = 'Rte_Type.h';
  | T_U_mV_1_1_s16.DataTypeMode = 'Fixed-point: slope and bias scaling';
  | T_U_mV_1_1_s16.SignednessBool = true;
  | T_U_mV_1_1_s16.WordLength = 16;
  | T_U_mV_1_1_s16.FixedExponent = 0;
  | T_U_mV_1_1_s16.SlopeAdjustmentFactor = 1;
  | T_U_mV_1_1_s16.Bias = 0;
  | T_U_mV_1_1_s16.DataTypeOverride = 'Inherit';
  | T_U_mV_1_1_s16.IsAlias = true;
  | 
  | T_U_mV_256_20_u16 = Simulink.NumericType;
  | T_U_mV_256_20_u16.Description = 'mV (millivolts  (mV))';
  | if (tmpVer > 7.11)
  | 	T_U_mV_256_20_u16.DataScope = 'Auto';
  | end
  | T_U_mV_256_20_u16.HeaderFile = 'Rte_Type.h';
  | T_U_mV_256_20_u16.DataTypeMode = 'Fixed-point: slope and bias scaling';
  | T_U_mV_256_20_u16.SignednessBool = false;
  | T_U_mV_256_20_u16.WordLength = 16;
  | T_U_mV_256_20_u16.FixedExponent = -4;
  | T_U_mV_256_20_u16.SlopeAdjustmentFactor = 1.25;
  | T_U_mV_256_20_u16.Bias = 0;
  | T_U_mV_256_20_u16.DataTypeOverride = 'Inherit';
  | T_U_mV_256_20_u16.IsAlias = true;
  | 
  | T_U_mV_Float32 = Simulink.NumericType;
  | T_U_mV_Float32.Description = 'mV (millivolts  (mV))';
  | if (tmpVer > 7.11)
  | 	T_U_mV_Float32.DataScope = 'Auto';
  | end
  | T_U_mV_Float32.HeaderFile = 'Rte_Type.h';
  | T_U_mV_Float32.DataTypeMode = 'Single';
  | T_U_mV_Float32.SignednessBool = true;
  | T_U_mV_Float32.WordLength = 32;
  | T_U_mV_Float32.FixedExponent = 0;
  | T_U_mV_Float32.SlopeAdjustmentFactor = 1;
  | T_U_mV_Float32.Bias = 0;
  | T_U_mV_Float32.DataTypeOverride = 'Inherit';
  | T_U_mV_Float32.IsAlias = true;
  | 
  | T_V_l_256_1_s16 = Simulink.NumericType;
  | T_V_l_256_1_s16.Description = 'l (liters  (l))';
  | if (tmpVer > 7.11)
  | 	T_V_l_256_1_s16.DataScope = 'Auto';
  | end
  | T_V_l_256_1_s16.HeaderFile = 'Rte_Type.h';
  | T_V_l_256_1_s16.DataTypeMode = 'Fixed-point: slope and bias scaling';
  | T_V_l_256_1_s16.SignednessBool = true;
  | T_V_l_256_1_s16.WordLength = 16;
  | T_V_l_256_1_s16.FixedExponent = -8;
  | T_V_l_256_1_s16.SlopeAdjustmentFactor = 1;
  | T_V_l_256_1_s16.Bias = 0;
  | T_V_l_256_1_s16.DataTypeOverride = 'Inherit';
  | T_V_l_256_1_s16.IsAlias = true;
  | 
  | T_V_l_4096_1_s16 = Simulink.NumericType;
  | T_V_l_4096_1_s16.Description = 'l (liters  (l))';
  | if (tmpVer > 7.11)
  | 	T_V_l_4096_1_s16.DataScope = 'Auto';
  | end
  | T_V_l_4096_1_s16.HeaderFile = 'Rte_Type.h';
  | T_V_l_4096_1_s16.DataTypeMode = 'Fixed-point: slope and bias scaling';
  | T_V_l_4096_1_s16.SignednessBool = true;
  | T_V_l_4096_1_s16.WordLength = 16;
  | T_V_l_4096_1_s16.FixedExponent = -12;
  | T_V_l_4096_1_s16.SlopeAdjustmentFactor = 1;
  | T_V_l_4096_1_s16.Bias = 0;
  | T_V_l_4096_1_s16.DataTypeOverride = 'Inherit';
  | T_V_l_4096_1_s16.IsAlias = true;
  | 
  | T_V_l_64_1_s16 = Simulink.NumericType;
  | T_V_l_64_1_s16.Description = 'l (liters  (l))';
  | if (tmpVer > 7.11)
  | 	T_V_l_64_1_s16.DataScope = 'Auto';
  | end
  | T_V_l_64_1_s16.HeaderFile = 'Rte_Type.h';
  | T_V_l_64_1_s16.DataTypeMode = 'Fixed-point: slope and bias scaling';
  | T_V_l_64_1_s16.SignednessBool = true;
  | T_V_l_64_1_s16.WordLength = 16;
  | T_V_l_64_1_s16.FixedExponent = -6;
  | T_V_l_64_1_s16.SlopeAdjustmentFactor = 1;
  | T_V_l_64_1_s16.Bias = 0;
  | T_V_l_64_1_s16.DataTypeOverride = 'Inherit';
  | T_V_l_64_1_s16.IsAlias = true;
  | 
  | T_V_l_65535_100_u16 = Simulink.NumericType;
  | T_V_l_65535_100_u16.Description = 'l (liters  (l))';
  | if (tmpVer > 7.11)
  | 	T_V_l_65535_100_u16.DataScope = 'Auto';
  | end
  | T_V_l_65535_100_u16.HeaderFile = 'Rte_Type.h';
  | T_V_l_65535_100_u16.DataTypeMode = ['Fixed-point: slope and bias scalin' ...
  |                                     'g'];
  | T_V_l_65535_100_u16.SignednessBool = false;
  | T_V_l_65535_100_u16.WordLength = 16;
  | T_V_l_65535_100_u16.FixedExponent = -10;
  | T_V_l_65535_100_u16.SlopeAdjustmentFactor = 1.5625238422217136;
  | T_V_l_65535_100_u16.Bias = 0;
  | T_V_l_65535_100_u16.DataTypeOverride = 'Inherit';
  | T_V_l_65535_100_u16.IsAlias = true;
  | 
  | T_V_l_Float32 = Simulink.NumericType;
  | T_V_l_Float32.Description = 'l (liters  (l))';
  | if (tmpVer > 7.11)
  | 	T_V_l_Float32.DataScope = 'Auto';
  | end
  | T_V_l_Float32.HeaderFile = 'Rte_Type.h';
  | T_V_l_Float32.DataTypeMode = 'Single';
  | T_V_l_Float32.SignednessBool = true;
  | T_V_l_Float32.WordLength = 32;
  | T_V_l_Float32.FixedExponent = 0;
  | T_V_l_Float32.SlopeAdjustmentFactor = 1;
  | T_V_l_Float32.Bias = 0;
  | T_V_l_Float32.DataTypeOverride = 'Inherit';
  | T_V_l_Float32.IsAlias = true;
  | 
  | T_V_ml_128_1_s16 = Simulink.NumericType;
  | T_V_ml_128_1_s16.Description = 'ml (milliliters  (ml))';
  | if (tmpVer > 7.11)
  | 	T_V_ml_128_1_s16.DataScope = 'Auto';
  | end
  | T_V_ml_128_1_s16.HeaderFile = 'Rte_Type.h';
  | T_V_ml_128_1_s16.DataTypeMode = 'Fixed-point: slope and bias scaling';
  | T_V_ml_128_1_s16.SignednessBool = true;
  | T_V_ml_128_1_s16.WordLength = 16;
  | T_V_ml_128_1_s16.FixedExponent = -7;
  | T_V_ml_128_1_s16.SlopeAdjustmentFactor = 1;
  | T_V_ml_128_1_s16.Bias = 0;
  | T_V_ml_128_1_s16.DataTypeOverride = 'Inherit';
  | T_V_ml_128_1_s16.IsAlias = true;
  | 
  | T_V_ml_1_1_s16 = Simulink.NumericType;
  | T_V_ml_1_1_s16.Description = 'ml (milliliters  (ml))';
  | if (tmpVer > 7.11)
  | 	T_V_ml_1_1_s16.DataScope = 'Auto';
  | end
  | T_V_ml_1_1_s16.HeaderFile = 'Rte_Type.h';
  | T_V_ml_1_1_s16.DataTypeMode = 'Fixed-point: slope and bias scaling';
  | T_V_ml_1_1_s16.SignednessBool = true;
  | T_V_ml_1_1_s16.WordLength = 16;
  | T_V_ml_1_1_s16.FixedExponent = 0;
  | T_V_ml_1_1_s16.SlopeAdjustmentFactor = 1;
  | T_V_ml_1_1_s16.Bias = 0;
  | T_V_ml_1_1_s16.DataTypeOverride = 'Inherit';
  | T_V_ml_1_1_s16.IsAlias = true;
  | 
  | T_V_ml_32768_1_s16 = Simulink.NumericType;
  | T_V_ml_32768_1_s16.Description = 'ml (milliliters  (ml))';
  | if (tmpVer > 7.11)
  | 	T_V_ml_32768_1_s16.DataScope = 'Auto';
  | end
  | T_V_ml_32768_1_s16.HeaderFile = 'Rte_Type.h';
  | T_V_ml_32768_1_s16.DataTypeMode = 'Fixed-point: slope and bias scaling';
  | T_V_ml_32768_1_s16.SignednessBool = true;
  | T_V_ml_32768_1_s16.WordLength = 16;
  | T_V_ml_32768_1_s16.FixedExponent = -15;
  | T_V_ml_32768_1_s16.SlopeAdjustmentFactor = 1;
  | T_V_ml_32768_1_s16.Bias = 0;
  | T_V_ml_32768_1_s16.DataTypeOverride = 'Inherit';
  | T_V_ml_32768_1_s16.IsAlias = true;
  | 
  | T_V_ml_Float32 = Simulink.NumericType;
  | T_V_ml_Float32.Description = 'ml (milliliters  (ml))';
  | if (tmpVer > 7.11)
  | 	T_V_ml_Float32.DataScope = 'Auto';
  | end
  | T_V_ml_Float32.HeaderFile = 'Rte_Type.h';
  | T_V_ml_Float32.DataTypeMode = 'Single';
  | T_V_ml_Float32.SignednessBool = true;
  | T_V_ml_Float32.WordLength = 32;
  | T_V_ml_Float32.FixedExponent = 0;
  | T_V_ml_Float32.SlopeAdjustmentFactor = 1;
  | T_V_ml_Float32.Bias = 0;
  | T_V_ml_Float32.DataTypeOverride = 'Inherit';
  | T_V_ml_Float32.IsAlias = true;
  | 
  | T_V_ul_32_1_u16 = Simulink.NumericType;
  | T_V_ul_32_1_u16.Description = 'ul (microliters  (ul))';
  | if (tmpVer > 7.11)
  | 	T_V_ul_32_1_u16.DataScope = 'Auto';
  | end
  | T_V_ul_32_1_u16.HeaderFile = 'Rte_Type.h';
  | T_V_ul_32_1_u16.DataTypeMode = 'Fixed-point: slope and bias scaling';
  | T_V_ul_32_1_u16.SignednessBool = false;
  | T_V_ul_32_1_u16.WordLength = 16;
  | T_V_ul_32_1_u16.FixedExponent = -5;
  | T_V_ul_32_1_u16.SlopeAdjustmentFactor = 1;
  | T_V_ul_32_1_u16.Bias = 0;
  | T_V_ul_32_1_u16.DataTypeOverride = 'Inherit';
  | T_V_ul_32_1_u16.IsAlias = true;
  | 
  | T_V_ul_Float32 = Simulink.NumericType;
  | T_V_ul_Float32.Description = 'ul (microliters  (ul))';
  | if (tmpVer > 7.11)
  | 	T_V_ul_Float32.DataScope = 'Auto';
  | end
  | T_V_ul_Float32.HeaderFile = 'Rte_Type.h';
  | T_V_ul_Float32.DataTypeMode = 'Single';
  | T_V_ul_Float32.SignednessBool = true;
  | T_V_ul_Float32.WordLength = 32;
  | T_V_ul_Float32.FixedExponent = 0;
  | T_V_ul_Float32.SlopeAdjustmentFactor = 1;
  | T_V_ul_Float32.Bias = 0;
  | T_V_ul_Float32.DataTypeOverride = 'Inherit';
  | T_V_ul_Float32.IsAlias = true;
  | 
  | T_Vpl_clpkm_512_1_u16 = Simulink.NumericType;
  | T_Vpl_clpkm_512_1_u16.Description = 'clpkm (liters / 100km  (clpkm))';
  | if (tmpVer > 7.11)
  | 	T_Vpl_clpkm_512_1_u16.DataScope = 'Auto';
  | end
  | T_Vpl_clpkm_512_1_u16.HeaderFile = 'Rte_Type.h';
  | T_Vpl_clpkm_512_1_u16.DataTypeMode = ...
  |   'Fixed-point: slope and bias scaling';
  | T_Vpl_clpkm_512_1_u16.SignednessBool = false;
  | T_Vpl_clpkm_512_1_u16.WordLength = 16;
  | T_Vpl_clpkm_512_1_u16.FixedExponent = -9;
  | T_Vpl_clpkm_512_1_u16.SlopeAdjustmentFactor = 1;
  | T_Vpl_clpkm_512_1_u16.Bias = 0;
  | T_Vpl_clpkm_512_1_u16.DataTypeOverride = 'Inherit';
  | T_Vpl_clpkm_512_1_u16.IsAlias = true;
  | 
  | T_Vpl_clpkm_Float32 = Simulink.NumericType;
  | T_Vpl_clpkm_Float32.Description = 'clpkm (liters / 100km  (clpkm))';
  | if (tmpVer > 7.11)
  | 	T_Vpl_clpkm_Float32.DataScope = 'Auto';
  | end
  | T_Vpl_clpkm_Float32.HeaderFile = 'Rte_Type.h';
  | T_Vpl_clpkm_Float32.DataTypeMode = 'Single';
  | T_Vpl_clpkm_Float32.SignednessBool = true;
  | T_Vpl_clpkm_Float32.WordLength = 32;
  | T_Vpl_clpkm_Float32.FixedExponent = 0;
  | T_Vpl_clpkm_Float32.SlopeAdjustmentFactor = 1;
  | T_Vpl_clpkm_Float32.Bias = 0;
  | T_Vpl_clpkm_Float32.DataTypeOverride = 'Inherit';
  | T_Vpl_clpkm_Float32.IsAlias = true;
  | 
  | T_a_kphps_16_1_s16 = Simulink.NumericType;
  | T_a_kphps_16_1_s16.Description = ['kphps (kilometers / hour / second  (' ...
  |                                   'kph/s))'];
  | if (tmpVer > 7.11)
  | 	T_a_kphps_16_1_s16.DataScope = 'Auto';
  | end
  | T_a_kphps_16_1_s16.HeaderFile = 'Rte_Type.h';
  | T_a_kphps_16_1_s16.DataTypeMode = 'Fixed-point: slope and bias scaling';
  | T_a_kphps_16_1_s16.SignednessBool = true;
  | T_a_kphps_16_1_s16.WordLength = 16;
  | T_a_kphps_16_1_s16.FixedExponent = -4;
  | T_a_kphps_16_1_s16.SlopeAdjustmentFactor = 1;
  | T_a_kphps_16_1_s16.Bias = 0;
  | T_a_kphps_16_1_s16.DataTypeOverride = 'Inherit';
  | T_a_kphps_16_1_s16.IsAlias = true;
  | 
  | T_a_kphps_Float32 = Simulink.NumericType;
  | T_a_kphps_Float32.Description = ['kphps (kilometers / hour / second  (k' ...
  |                                  'ph/s))'];
  | if (tmpVer > 7.11)
  | 	T_a_kphps_Float32.DataScope = 'Auto';
  | end
  | T_a_kphps_Float32.HeaderFile = 'Rte_Type.h';
  | T_a_kphps_Float32.DataTypeMode = 'Single';
  | T_a_kphps_Float32.SignednessBool = true;
  | T_a_kphps_Float32.WordLength = 32;
  | T_a_kphps_Float32.FixedExponent = 0;
  | T_a_kphps_Float32.SlopeAdjustmentFactor = 1;
  | T_a_kphps_Float32.Bias = 0;
  | T_a_kphps_Float32.DataTypeOverride = 'Inherit';
  | T_a_kphps_Float32.IsAlias = true;
  | 
  | T_a_mps2_128_1_s16 = Simulink.NumericType;
  | T_a_mps2_128_1_s16.Description = 'mps2 (meters / second2  (m/s2))';
  | if (tmpVer > 7.11)
  | 	T_a_mps2_128_1_s16.DataScope = 'Auto';
  | end
  | T_a_mps2_128_1_s16.HeaderFile = 'Rte_Type.h';
  | T_a_mps2_128_1_s16.DataTypeMode = 'Fixed-point: slope and bias scaling';
  | T_a_mps2_128_1_s16.SignednessBool = true;
  | T_a_mps2_128_1_s16.WordLength = 16;
  | T_a_mps2_128_1_s16.FixedExponent = -7;
  | T_a_mps2_128_1_s16.SlopeAdjustmentFactor = 1;
  | T_a_mps2_128_1_s16.Bias = 0;
  | T_a_mps2_128_1_s16.DataTypeOverride = 'Inherit';
  | T_a_mps2_128_1_s16.IsAlias = true;
  | 
  | T_a_mps2_Float32 = Simulink.NumericType;
  | T_a_mps2_Float32.Description = 'mps2 (meters / second2  (m/s2))';
  | if (tmpVer > 7.11)
  | 	T_a_mps2_Float32.DataScope = 'Auto';
  | end
  | T_a_mps2_Float32.HeaderFile = 'Rte_Type.h';
  | T_a_mps2_Float32.DataTypeMode = 'Single';
  | T_a_mps2_Float32.SignednessBool = true;
  | T_a_mps2_Float32.WordLength = 32;
  | T_a_mps2_Float32.FixedExponent = 0;
  | T_a_mps2_Float32.SlopeAdjustmentFactor = 1;
  | T_a_mps2_Float32.Bias = 0;
  | T_a_mps2_Float32.DataTypeOverride = 'Inherit';
  | T_a_mps2_Float32.IsAlias = true;
  | 
  | T_c_MJpkg_256_1_s16 = Simulink.NumericType;
  | T_c_MJpkg_256_1_s16.Description = ['MJpkg (megajoules / kilogram  (MJ/(' ...
  |                                    'kg*K)))'];
  | if (tmpVer > 7.11)
  | 	T_c_MJpkg_256_1_s16.DataScope = 'Auto';
  | end
  | T_c_MJpkg_256_1_s16.HeaderFile = 'Rte_Type.h';
  | T_c_MJpkg_256_1_s16.DataTypeMode = ['Fixed-point: slope and bias scalin' ...
  |                                     'g'];
  | T_c_MJpkg_256_1_s16.SignednessBool = true;
  | T_c_MJpkg_256_1_s16.WordLength = 16;
  | T_c_MJpkg_256_1_s16.FixedExponent = -8;
  | T_c_MJpkg_256_1_s16.SlopeAdjustmentFactor = 1;
  | T_c_MJpkg_256_1_s16.Bias = 0;
  | T_c_MJpkg_256_1_s16.DataTypeOverride = 'Inherit';
  | T_c_MJpkg_256_1_s16.IsAlias = true;
  | 
  | T_c_MJpkg_Float32 = Simulink.NumericType;
  | T_c_MJpkg_Float32.Description = ['MJpkg (megajoules / kilogram  (MJ/(kg' ...
  |                                  '*K)))'];
  | if (tmpVer > 7.11)
  | 	T_c_MJpkg_Float32.DataScope = 'Auto';
  | end
  | T_c_MJpkg_Float32.HeaderFile = 'Rte_Type.h';
  | T_c_MJpkg_Float32.DataTypeMode = 'Single';
  | T_c_MJpkg_Float32.SignednessBool = true;
  | T_c_MJpkg_Float32.WordLength = 32;
  | T_c_MJpkg_Float32.FixedExponent = 0;
  | T_c_MJpkg_Float32.SlopeAdjustmentFactor = 1;
  | T_c_MJpkg_Float32.Bias = 0;
  | T_c_MJpkg_Float32.DataTypeOverride = 'Inherit';
  | T_c_MJpkg_Float32.IsAlias = true;
  | 
  | T_c_kJpgpK_1024_1_s16 = Simulink.NumericType;
  | T_c_kJpgpK_1024_1_s16.Description = ...
  |   'kJpgpK (kjoules / gram  (kJ/(g*K)))';
  | if (tmpVer > 7.11)
  | 	T_c_kJpgpK_1024_1_s16.DataScope = 'Auto';
  | end
  | T_c_kJpgpK_1024_1_s16.HeaderFile = 'Rte_Type.h';
  | T_c_kJpgpK_1024_1_s16.DataTypeMode = ...
  |   'Fixed-point: slope and bias scaling';
  | T_c_kJpgpK_1024_1_s16.SignednessBool = true;
  | T_c_kJpgpK_1024_1_s16.WordLength = 16;
  | T_c_kJpgpK_1024_1_s16.FixedExponent = -10;
  | T_c_kJpgpK_1024_1_s16.SlopeAdjustmentFactor = 1;
  | T_c_kJpgpK_1024_1_s16.Bias = 0;
  | T_c_kJpgpK_1024_1_s16.DataTypeOverride = 'Inherit';
  | T_c_kJpgpK_1024_1_s16.IsAlias = true;
  | 
  | T_c_kJpgpK_Float32 = Simulink.NumericType;
  | T_c_kJpgpK_Float32.Description = 'kJpgpK (kjoules / gram  (kJ/(g*K)))';
  | if (tmpVer > 7.11)
  | 	T_c_kJpgpK_Float32.DataScope = 'Auto';
  | end
  | T_c_kJpgpK_Float32.HeaderFile = 'Rte_Type.h';
  | T_c_kJpgpK_Float32.DataTypeMode = 'Single';
  | T_c_kJpgpK_Float32.SignednessBool = true;
  | T_c_kJpgpK_Float32.WordLength = 32;
  | T_c_kJpgpK_Float32.FixedExponent = 0;
  | T_c_kJpgpK_Float32.SlopeAdjustmentFactor = 1;
  | T_c_kJpgpK_Float32.Bias = 0;
  | T_c_kJpgpK_Float32.DataTypeOverride = 'Inherit';
  | T_c_kJpgpK_Float32.IsAlias = true;
  | 
  | T_c_kJpkgpK_128_1_u16 = Simulink.NumericType;
  | T_c_kJpkgpK_128_1_u16.Description = ...
  |   'kJpkgpK (kilojoules / kilogram Kelvin  (kJ/(kg*K)))';
  | if (tmpVer > 7.11)
  | 	T_c_kJpkgpK_128_1_u16.DataScope = 'Auto';
  | end
  | T_c_kJpkgpK_128_1_u16.HeaderFile = 'Rte_Type.h';
  | T_c_kJpkgpK_128_1_u16.DataTypeMode = ...
  |   'Fixed-point: slope and bias scaling';
  | T_c_kJpkgpK_128_1_u16.SignednessBool = false;
  | T_c_kJpkgpK_128_1_u16.WordLength = 16;
  | T_c_kJpkgpK_128_1_u16.FixedExponent = -7;
  | T_c_kJpkgpK_128_1_u16.SlopeAdjustmentFactor = 1;
  | T_c_kJpkgpK_128_1_u16.Bias = 0;
  | T_c_kJpkgpK_128_1_u16.DataTypeOverride = 'Inherit';
  | T_c_kJpkgpK_128_1_u16.IsAlias = true;
  | 
  | T_c_kJpkgpK_Float32 = Simulink.NumericType;
  | T_c_kJpkgpK_Float32.Description = ['kJpkgpK (kilojoules / kilogram Kelv' ...
  |                                    'in  (kJ/(kg*K)))'];
  | if (tmpVer > 7.11)
  | 	T_c_kJpkgpK_Float32.DataScope = 'Auto';
  | end
  | T_c_kJpkgpK_Float32.HeaderFile = 'Rte_Type.h';
  | T_c_kJpkgpK_Float32.DataTypeMode = 'Single';
  | T_c_kJpkgpK_Float32.SignednessBool = true;
  | T_c_kJpkgpK_Float32.WordLength = 32;
  | T_c_kJpkgpK_Float32.FixedExponent = 0;
  | T_c_kJpkgpK_Float32.SlopeAdjustmentFactor = 1;
  | T_c_kJpkgpK_Float32.Bias = 0;
  | T_c_kJpkgpK_Float32.DataTypeOverride = 'Inherit';
  | T_c_kJpkgpK_Float32.IsAlias = true;
  | 
  | T_chrg_Ah_1_1_s16 = Simulink.NumericType;
  | T_chrg_Ah_1_1_s16.Description = 'Ah (ampere-hours  (Ah))';
  | if (tmpVer > 7.11)
  | 	T_chrg_Ah_1_1_s16.DataScope = 'Auto';
  | end
  | T_chrg_Ah_1_1_s16.HeaderFile = 'Rte_Type.h';
  | T_chrg_Ah_1_1_s16.DataTypeMode = 'Fixed-point: slope and bias scaling';
  | T_chrg_Ah_1_1_s16.SignednessBool = true;
  | T_chrg_Ah_1_1_s16.WordLength = 16;
  | T_chrg_Ah_1_1_s16.FixedExponent = 0;
  | T_chrg_Ah_1_1_s16.SlopeAdjustmentFactor = 1;
  | T_chrg_Ah_1_1_s16.Bias = 0;
  | T_chrg_Ah_1_1_s16.DataTypeOverride = 'Inherit';
  | T_chrg_Ah_1_1_s16.IsAlias = true;
  | 
  | T_chrg_Ah_1_1_u16 = Simulink.NumericType;
  | T_chrg_Ah_1_1_u16.Description = 'Ah (ampere-hours  (Ah))';
  | if (tmpVer > 7.11)
  | 	T_chrg_Ah_1_1_u16.DataScope = 'Auto';
  | end
  | T_chrg_Ah_1_1_u16.HeaderFile = 'Rte_Type.h';
  | T_chrg_Ah_1_1_u16.DataTypeMode = 'Fixed-point: slope and bias scaling';
  | T_chrg_Ah_1_1_u16.SignednessBool = false;
  | T_chrg_Ah_1_1_u16.WordLength = 16;
  | T_chrg_Ah_1_1_u16.FixedExponent = 0;
  | T_chrg_Ah_1_1_u16.SlopeAdjustmentFactor = 1;
  | T_chrg_Ah_1_1_u16.Bias = 0;
  | T_chrg_Ah_1_1_u16.DataTypeOverride = 'Inherit';
  | T_chrg_Ah_1_1_u16.IsAlias = true;
  | 
  | T_chrg_Ah_1_1_u8 = Simulink.NumericType;
  | T_chrg_Ah_1_1_u8.Description = 'Ah (ampere-hours  (Ah))';
  | if (tmpVer > 7.11)
  | 	T_chrg_Ah_1_1_u8.DataScope = 'Auto';
  | end
  | T_chrg_Ah_1_1_u8.HeaderFile = 'Rte_Type.h';
  | T_chrg_Ah_1_1_u8.DataTypeMode = 'Fixed-point: slope and bias scaling';
  | T_chrg_Ah_1_1_u8.SignednessBool = false;
  | T_chrg_Ah_1_1_u8.WordLength = 8;
  | T_chrg_Ah_1_1_u8.FixedExponent = 0;
  | T_chrg_Ah_1_1_u8.SlopeAdjustmentFactor = 1;
  | T_chrg_Ah_1_1_u8.Bias = 0;
  | T_chrg_Ah_1_1_u8.DataTypeOverride = 'Inherit';
  | T_chrg_Ah_1_1_u8.IsAlias = true;
  | 
  | T_chrg_Ah_256_1_u16 = Simulink.NumericType;
  | T_chrg_Ah_256_1_u16.Description = 'Ah (ampere-hours  (Ah))';
  | if (tmpVer > 7.11)
  | 	T_chrg_Ah_256_1_u16.DataScope = 'Auto';
  | end
  | T_chrg_Ah_256_1_u16.HeaderFile = 'Rte_Type.h';
  | T_chrg_Ah_256_1_u16.DataTypeMode = ['Fixed-point: slope and bias scalin' ...
  |                                     'g'];
  | T_chrg_Ah_256_1_u16.SignednessBool = false;
  | T_chrg_Ah_256_1_u16.WordLength = 16;
  | T_chrg_Ah_256_1_u16.FixedExponent = -8;
  | T_chrg_Ah_256_1_u16.SlopeAdjustmentFactor = 1;
  | T_chrg_Ah_256_1_u16.Bias = 0;
  | T_chrg_Ah_256_1_u16.DataTypeOverride = 'Inherit';
  | T_chrg_Ah_256_1_u16.IsAlias = true;
  | 
  | T_chrg_Ah_4194304_1_s32 = Simulink.NumericType;
  | T_chrg_Ah_4194304_1_s32.Description = 'Ah (ampere-hours  (Ah))';
  | if (tmpVer > 7.11)
  | 	T_chrg_Ah_4194304_1_s32.DataScope = 'Auto';
  | end
  | T_chrg_Ah_4194304_1_s32.HeaderFile = 'Rte_Type.h';
  | T_chrg_Ah_4194304_1_s32.DataTypeMode = ...
  |   'Fixed-point: slope and bias scaling';
  | T_chrg_Ah_4194304_1_s32.SignednessBool = true;
  | T_chrg_Ah_4194304_1_s32.WordLength = 32;
  | T_chrg_Ah_4194304_1_s32.FixedExponent = -22;
  | T_chrg_Ah_4194304_1_s32.SlopeAdjustmentFactor = 1;
  | T_chrg_Ah_4194304_1_s32.Bias = 0;
  | T_chrg_Ah_4194304_1_s32.DataTypeOverride = 'Inherit';
  | T_chrg_Ah_4194304_1_s32.IsAlias = true;
  | 
  | T_chrg_Ah_512_1_u16 = Simulink.NumericType;
  | T_chrg_Ah_512_1_u16.Description = 'Ah (ampere-hours  (Ah))';
  | if (tmpVer > 7.11)
  | 	T_chrg_Ah_512_1_u16.DataScope = 'Auto';
  | end
  | T_chrg_Ah_512_1_u16.HeaderFile = 'Rte_Type.h';
  | T_chrg_Ah_512_1_u16.DataTypeMode = ['Fixed-point: slope and bias scalin' ...
  |                                     'g'];
  | T_chrg_Ah_512_1_u16.SignednessBool = false;
  | T_chrg_Ah_512_1_u16.WordLength = 16;
  | T_chrg_Ah_512_1_u16.FixedExponent = -9;
  | T_chrg_Ah_512_1_u16.SlopeAdjustmentFactor = 1;
  | T_chrg_Ah_512_1_u16.Bias = 0;
  | T_chrg_Ah_512_1_u16.DataTypeOverride = 'Inherit';
  | T_chrg_Ah_512_1_u16.IsAlias = true;
  | 
  | T_chrg_Ah_8_1_u16 = Simulink.NumericType;
  | T_chrg_Ah_8_1_u16.Description = 'Ah (ampere-hours  (Ah))';
  | if (tmpVer > 7.11)
  | 	T_chrg_Ah_8_1_u16.DataScope = 'Auto';
  | end
  | T_chrg_Ah_8_1_u16.HeaderFile = 'Rte_Type.h';
  | T_chrg_Ah_8_1_u16.DataTypeMode = 'Fixed-point: slope and bias scaling';
  | T_chrg_Ah_8_1_u16.SignednessBool = false;
  | T_chrg_Ah_8_1_u16.WordLength = 16;
  | T_chrg_Ah_8_1_u16.FixedExponent = -3;
  | T_chrg_Ah_8_1_u16.SlopeAdjustmentFactor = 1;
  | T_chrg_Ah_8_1_u16.Bias = 0;
  | T_chrg_Ah_8_1_u16.DataTypeOverride = 'Inherit';
  | T_chrg_Ah_8_1_u16.IsAlias = true;
  | 
  | T_chrg_Ah_Float32 = Simulink.NumericType;
  | T_chrg_Ah_Float32.Description = 'Ah (ampere-hours  (Ah))';
  | if (tmpVer > 7.11)
  | 	T_chrg_Ah_Float32.DataScope = 'Auto';
  | end
  | T_chrg_Ah_Float32.HeaderFile = 'Rte_Type.h';
  | T_chrg_Ah_Float32.DataTypeMode = 'Single';
  | T_chrg_Ah_Float32.SignednessBool = true;
  | T_chrg_Ah_Float32.WordLength = 32;
  | T_chrg_Ah_Float32.FixedExponent = 0;
  | T_chrg_Ah_Float32.SlopeAdjustmentFactor = 1;
  | T_chrg_Ah_Float32.Bias = 0;
  | T_chrg_Ah_Float32.DataTypeOverride = 'Inherit';
  | T_chrg_Ah_Float32.IsAlias = true;
  | 
  | T_cmp_NA_100_1_s16 = Simulink.NumericType;
  | T_cmp_NA_100_1_s16.Description = ['NA (dependent upon the composition o' ...
  |                                   'f units)'];
  | if (tmpVer > 7.11)
  | 	T_cmp_NA_100_1_s16.DataScope = 'Auto';
  | end
  | T_cmp_NA_100_1_s16.HeaderFile = 'Rte_Type.h';
  | T_cmp_NA_100_1_s16.DataTypeMode = 'Fixed-point: slope and bias scaling';
  | T_cmp_NA_100_1_s16.SignednessBool = true;
  | T_cmp_NA_100_1_s16.WordLength = 16;
  | T_cmp_NA_100_1_s16.FixedExponent = -7;
  | T_cmp_NA_100_1_s16.SlopeAdjustmentFactor = 1.28;
  | T_cmp_NA_100_1_s16.Bias = 0;
  | T_cmp_NA_100_1_s16.DataTypeOverride = 'Inherit';
  | T_cmp_NA_100_1_s16.IsAlias = true;
  | 
  | T_cmp_NA_128_1_s16 = Simulink.NumericType;
  | T_cmp_NA_128_1_s16.Description = ['NA (dependent upon the composition o' ...
  |                                   'f units)'];
  | if (tmpVer > 7.11)
  | 	T_cmp_NA_128_1_s16.DataScope = 'Auto';
  | end
  | T_cmp_NA_128_1_s16.HeaderFile = 'Rte_Type.h';
  | T_cmp_NA_128_1_s16.DataTypeMode = 'Fixed-point: slope and bias scaling';
  | T_cmp_NA_128_1_s16.SignednessBool = true;
  | T_cmp_NA_128_1_s16.WordLength = 16;
  | T_cmp_NA_128_1_s16.FixedExponent = -7;
  | T_cmp_NA_128_1_s16.SlopeAdjustmentFactor = 1;
  | T_cmp_NA_128_1_s16.Bias = 0;
  | T_cmp_NA_128_1_s16.DataTypeOverride = 'Inherit';
  | T_cmp_NA_128_1_s16.IsAlias = true;
  | 
  | T_cmp_NA_16_1_s16 = Simulink.NumericType;
  | T_cmp_NA_16_1_s16.Description = ['NA (dependent upon the composition of' ...
  |                                  ' units)'];
  | if (tmpVer > 7.11)
  | 	T_cmp_NA_16_1_s16.DataScope = 'Auto';
  | end
  | T_cmp_NA_16_1_s16.HeaderFile = 'Rte_Type.h';
  | T_cmp_NA_16_1_s16.DataTypeMode = 'Fixed-point: slope and bias scaling';
  | T_cmp_NA_16_1_s16.SignednessBool = true;
  | T_cmp_NA_16_1_s16.WordLength = 16;
  | T_cmp_NA_16_1_s16.FixedExponent = -4;
  | T_cmp_NA_16_1_s16.SlopeAdjustmentFactor = 1;
  | T_cmp_NA_16_1_s16.Bias = 0;
  | T_cmp_NA_16_1_s16.DataTypeOverride = 'Inherit';
  | T_cmp_NA_16_1_s16.IsAlias = true;
  | 
  | T_cmp_NA_32768_1_u16 = Simulink.NumericType;
  | T_cmp_NA_32768_1_u16.Description = ['NA (dependent upon the composition' ...
  |                                     ' of units)'];
  | if (tmpVer > 7.11)
  | 	T_cmp_NA_32768_1_u16.DataScope = 'Auto';
  | end
  | T_cmp_NA_32768_1_u16.HeaderFile = 'Rte_Type.h';
  | T_cmp_NA_32768_1_u16.DataTypeMode = ...
  |   'Fixed-point: slope and bias scaling';
  | T_cmp_NA_32768_1_u16.SignednessBool = false;
  | T_cmp_NA_32768_1_u16.WordLength = 16;
  | T_cmp_NA_32768_1_u16.FixedExponent = -15;
  | T_cmp_NA_32768_1_u16.SlopeAdjustmentFactor = 1;
  | T_cmp_NA_32768_1_u16.Bias = 0;
  | T_cmp_NA_32768_1_u16.DataTypeOverride = 'Inherit';
  | T_cmp_NA_32768_1_u16.IsAlias = true;
  | 
  | T_cmp_NA_Float32 = Simulink.NumericType;
  | T_cmp_NA_Float32.Description = ['NA (dependent upon the composition of ' ...
  |                                 'units)'];
  | if (tmpVer > 7.11)
  | 	T_cmp_NA_Float32.DataScope = 'Auto';
  | end
  | T_cmp_NA_Float32.HeaderFile = 'Rte_Type.h';
  | T_cmp_NA_Float32.DataTypeMode = 'Single';
  | T_cmp_NA_Float32.SignednessBool = true;
  | T_cmp_NA_Float32.WordLength = 32;
  | T_cmp_NA_Float32.FixedExponent = 0;
  | T_cmp_NA_Float32.SlopeAdjustmentFactor = 1;
  | T_cmp_NA_Float32.Bias = 0;
  | T_cmp_NA_Float32.DataTypeOverride = 'Inherit';
  | T_cmp_NA_Float32.IsAlias = true;
  | 
  | T_d2n_rpmps2_4_1_s16 = Simulink.NumericType;
  | T_d2n_rpmps2_4_1_s16.Description = ['rpmps2 (revolutions / minute / sec' ...
  |                                     'ond2  (rpm/s2))'];
  | if (tmpVer > 7.11)
  | 	T_d2n_rpmps2_4_1_s16.DataScope = 'Auto';
  | end
  | T_d2n_rpmps2_4_1_s16.HeaderFile = 'Rte_Type.h';
  | T_d2n_rpmps2_4_1_s16.DataTypeMode = ...
  |   'Fixed-point: slope and bias scaling';
  | T_d2n_rpmps2_4_1_s16.SignednessBool = true;
  | T_d2n_rpmps2_4_1_s16.WordLength = 16;
  | T_d2n_rpmps2_4_1_s16.FixedExponent = -2;
  | T_d2n_rpmps2_4_1_s16.SlopeAdjustmentFactor = 1;
  | T_d2n_rpmps2_4_1_s16.Bias = 0;
  | T_d2n_rpmps2_4_1_s16.DataTypeOverride = 'Inherit';
  | T_d2n_rpmps2_4_1_s16.IsAlias = true;
  | 
  | T_d2n_rpmps2_Float32 = Simulink.NumericType;
  | T_d2n_rpmps2_Float32.Description = ['rpmps2 (revolutions / minute / sec' ...
  |                                     'ond2  (rpm/s2))'];
  | if (tmpVer > 7.11)
  | 	T_d2n_rpmps2_Float32.DataScope = 'Auto';
  | end
  | T_d2n_rpmps2_Float32.HeaderFile = 'Rte_Type.h';
  | T_d2n_rpmps2_Float32.DataTypeMode = 'Single';
  | T_d2n_rpmps2_Float32.SignednessBool = true;
  | T_d2n_rpmps2_Float32.WordLength = 32;
  | T_d2n_rpmps2_Float32.FixedExponent = 0;
  | T_d2n_rpmps2_Float32.SlopeAdjustmentFactor = 1;
  | T_d2n_rpmps2_Float32.Bias = 0;
  | T_d2n_rpmps2_Float32.DataTypeOverride = 'Inherit';
  | T_d2n_rpmps2_Float32.IsAlias = true;
  | 
  | T_dPct_pctps_16_1_s16 = Simulink.NumericType;
  | T_dPct_pctps_16_1_s16.Description = 'pctps (percent / second  (%/s))';
  | if (tmpVer > 7.11)
  | 	T_dPct_pctps_16_1_s16.DataScope = 'Auto';
  | end
  | T_dPct_pctps_16_1_s16.HeaderFile = 'Rte_Type.h';
  | T_dPct_pctps_16_1_s16.DataTypeMode = ...
  |   'Fixed-point: slope and bias scaling';
  | T_dPct_pctps_16_1_s16.SignednessBool = true;
  | T_dPct_pctps_16_1_s16.WordLength = 16;
  | T_dPct_pctps_16_1_s16.FixedExponent = -4;
  | T_dPct_pctps_16_1_s16.SlopeAdjustmentFactor = 1;
  | T_dPct_pctps_16_1_s16.Bias = 0;
  | T_dPct_pctps_16_1_s16.DataTypeOverride = 'Inherit';
  | T_dPct_pctps_16_1_s16.IsAlias = true;
  | 
  | T_dPct_pctps_256_1_s16 = Simulink.NumericType;
  | T_dPct_pctps_256_1_s16.Description = 'pctps (percent / second  (%/s))';
  | if (tmpVer > 7.11)
  | 	T_dPct_pctps_256_1_s16.DataScope = 'Auto';
  | end
  | T_dPct_pctps_256_1_s16.HeaderFile = 'Rte_Type.h';
  | T_dPct_pctps_256_1_s16.DataTypeMode = ...
  |   'Fixed-point: slope and bias scaling';
  | T_dPct_pctps_256_1_s16.SignednessBool = true;
  | T_dPct_pctps_256_1_s16.WordLength = 16;
  | T_dPct_pctps_256_1_s16.FixedExponent = -8;
  | T_dPct_pctps_256_1_s16.SlopeAdjustmentFactor = 1;
  | T_dPct_pctps_256_1_s16.Bias = 0;
  | T_dPct_pctps_256_1_s16.DataTypeOverride = 'Inherit';
  | T_dPct_pctps_256_1_s16.IsAlias = true;
  | 
  | T_dPct_pctps_Float32 = Simulink.NumericType;
  | T_dPct_pctps_Float32.Description = 'pctps (percent / second  (%/s))';
  | if (tmpVer > 7.11)
  | 	T_dPct_pctps_Float32.DataScope = 'Auto';
  | end
  | T_dPct_pctps_Float32.HeaderFile = 'Rte_Type.h';
  | T_dPct_pctps_Float32.DataTypeMode = 'Single';
  | T_dPct_pctps_Float32.SignednessBool = true;
  | T_dPct_pctps_Float32.WordLength = 32;
  | T_dPct_pctps_Float32.FixedExponent = 0;
  | T_dPct_pctps_Float32.SlopeAdjustmentFactor = 1;
  | T_dPct_pctps_Float32.Bias = 0;
  | T_dPct_pctps_Float32.DataTypeOverride = 'Inherit';
  | T_dPct_pctps_Float32.IsAlias = true;
  | 
  | T_dT_degCps_128_1_s16 = Simulink.NumericType;
  | T_dT_degCps_128_1_s16.Description = ...
  |   'degCps (degrees Celsius / second  (deg C/s))';
  | if (tmpVer > 7.11)
  | 	T_dT_degCps_128_1_s16.DataScope = 'Auto';
  | end
  | T_dT_degCps_128_1_s16.HeaderFile = 'Rte_Type.h';
  | T_dT_degCps_128_1_s16.DataTypeMode = ...
  |   'Fixed-point: slope and bias scaling';
  | T_dT_degCps_128_1_s16.SignednessBool = true;
  | T_dT_degCps_128_1_s16.WordLength = 16;
  | T_dT_degCps_128_1_s16.FixedExponent = -7;
  | T_dT_degCps_128_1_s16.SlopeAdjustmentFactor = 1;
  | T_dT_degCps_128_1_s16.Bias = 0;
  | T_dT_degCps_128_1_s16.DataTypeOverride = 'Inherit';
  | T_dT_degCps_128_1_s16.IsAlias = true;
  | 
  | T_dT_degCps_Float32 = Simulink.NumericType;
  | T_dT_degCps_Float32.Description = ['degCps (degrees Celsius / second  (' ...
  |                                    'deg C/s))'];
  | if (tmpVer > 7.11)
  | 	T_dT_degCps_Float32.DataScope = 'Auto';
  | end
  | T_dT_degCps_Float32.HeaderFile = 'Rte_Type.h';
  | T_dT_degCps_Float32.DataTypeMode = 'Single';
  | T_dT_degCps_Float32.SignednessBool = true;
  | T_dT_degCps_Float32.WordLength = 32;
  | T_dT_degCps_Float32.FixedExponent = 0;
  | T_dT_degCps_Float32.SlopeAdjustmentFactor = 1;
  | T_dT_degCps_Float32.Bias = 0;
  | T_dT_degCps_Float32.DataTypeOverride = 'Inherit';
  | T_dT_degCps_Float32.IsAlias = true;
  | 
  | T_dV_lph_1_1_s16 = Simulink.NumericType;
  | T_dV_lph_1_1_s16.Description = 'lph (liters / hour (l/h))';
  | if (tmpVer > 7.11)
  | 	T_dV_lph_1_1_s16.DataScope = 'Auto';
  | end
  | T_dV_lph_1_1_s16.HeaderFile = 'Rte_Type.h';
  | T_dV_lph_1_1_s16.DataTypeMode = 'Fixed-point: slope and bias scaling';
  | T_dV_lph_1_1_s16.SignednessBool = true;
  | T_dV_lph_1_1_s16.WordLength = 16;
  | T_dV_lph_1_1_s16.FixedExponent = 0;
  | T_dV_lph_1_1_s16.SlopeAdjustmentFactor = 1;
  | T_dV_lph_1_1_s16.Bias = 0;
  | T_dV_lph_1_1_s16.DataTypeOverride = 'Inherit';
  | T_dV_lph_1_1_s16.IsAlias = true;
  | 
  | T_dV_lph_Float32 = Simulink.NumericType;
  | T_dV_lph_Float32.Description = 'lph (liters / hour (l/h))';
  | if (tmpVer > 7.11)
  | 	T_dV_lph_Float32.DataScope = 'Auto';
  | end
  | T_dV_lph_Float32.HeaderFile = 'Rte_Type.h';
  | T_dV_lph_Float32.DataTypeMode = 'Single';
  | T_dV_lph_Float32.SignednessBool = true;
  | T_dV_lph_Float32.WordLength = 32;
  | T_dV_lph_Float32.FixedExponent = 0;
  | T_dV_lph_Float32.SlopeAdjustmentFactor = 1;
  | T_dV_lph_Float32.Bias = 0;
  | T_dV_lph_Float32.DataTypeOverride = 'Inherit';
  | T_dV_lph_Float32.IsAlias = true;
  | 
  | T_dV_lpm_128_1_s16 = Simulink.NumericType;
  | T_dV_lpm_128_1_s16.Description = 'lpm (liters / minute  (l/m))';
  | if (tmpVer > 7.11)
  | 	T_dV_lpm_128_1_s16.DataScope = 'Auto';
  | end
  | T_dV_lpm_128_1_s16.HeaderFile = 'Rte_Type.h';
  | T_dV_lpm_128_1_s16.DataTypeMode = 'Fixed-point: slope and bias scaling';
  | T_dV_lpm_128_1_s16.SignednessBool = true;
  | T_dV_lpm_128_1_s16.WordLength = 16;
  | T_dV_lpm_128_1_s16.FixedExponent = -7;
  | T_dV_lpm_128_1_s16.SlopeAdjustmentFactor = 1;
  | T_dV_lpm_128_1_s16.Bias = 0;
  | T_dV_lpm_128_1_s16.DataTypeOverride = 'Inherit';
  | T_dV_lpm_128_1_s16.IsAlias = true;
  | 
  | T_dV_lpm_32_1_s16 = Simulink.NumericType;
  | T_dV_lpm_32_1_s16.Description = 'lpm (liters / minute  (l/m))';
  | if (tmpVer > 7.11)
  | 	T_dV_lpm_32_1_s16.DataScope = 'Auto';
  | end
  | T_dV_lpm_32_1_s16.HeaderFile = 'Rte_Type.h';
  | T_dV_lpm_32_1_s16.DataTypeMode = 'Fixed-point: slope and bias scaling';
  | T_dV_lpm_32_1_s16.SignednessBool = true;
  | T_dV_lpm_32_1_s16.WordLength = 16;
  | T_dV_lpm_32_1_s16.FixedExponent = -5;
  | T_dV_lpm_32_1_s16.SlopeAdjustmentFactor = 1;
  | T_dV_lpm_32_1_s16.Bias = 0;
  | T_dV_lpm_32_1_s16.DataTypeOverride = 'Inherit';
  | T_dV_lpm_32_1_s16.IsAlias = true;
  | 
  | T_dV_lpm_Float32 = Simulink.NumericType;
  | T_dV_lpm_Float32.Description = 'lpm (liters / minute  (l/m))';
  | if (tmpVer > 7.11)
  | 	T_dV_lpm_Float32.DataScope = 'Auto';
  | end
  | T_dV_lpm_Float32.HeaderFile = 'Rte_Type.h';
  | T_dV_lpm_Float32.DataTypeMode = 'Single';
  | T_dV_lpm_Float32.SignednessBool = true;
  | T_dV_lpm_Float32.WordLength = 32;
  | T_dV_lpm_Float32.FixedExponent = 0;
  | T_dV_lpm_Float32.SlopeAdjustmentFactor = 1;
  | T_dV_lpm_Float32.Bias = 0;
  | T_dV_lpm_Float32.DataTypeOverride = 'Inherit';
  | T_dV_lpm_Float32.IsAlias = true;
  | 
  | T_dV_lps_1024_1_u16 = Simulink.NumericType;
  | T_dV_lps_1024_1_u16.Description = 'lps (liters / second  (l/s))';
  | if (tmpVer > 7.11)
  | 	T_dV_lps_1024_1_u16.DataScope = 'Auto';
  | end
  | T_dV_lps_1024_1_u16.HeaderFile = 'Rte_Type.h';
  | T_dV_lps_1024_1_u16.DataTypeMode = ['Fixed-point: slope and bias scalin' ...
  |                                     'g'];
  | T_dV_lps_1024_1_u16.SignednessBool = false;
  | T_dV_lps_1024_1_u16.WordLength = 16;
  | T_dV_lps_1024_1_u16.FixedExponent = -10;
  | T_dV_lps_1024_1_u16.SlopeAdjustmentFactor = 1;
  | T_dV_lps_1024_1_u16.Bias = 0;
  | T_dV_lps_1024_1_u16.DataTypeOverride = 'Inherit';
  | T_dV_lps_1024_1_u16.IsAlias = true;
  | 
  | T_dV_lps_4_1_u16 = Simulink.NumericType;
  | T_dV_lps_4_1_u16.Description = 'lps (liters / second  (l/s))';
  | if (tmpVer > 7.11)
  | 	T_dV_lps_4_1_u16.DataScope = 'Auto';
  | end
  | T_dV_lps_4_1_u16.HeaderFile = 'Rte_Type.h';
  | T_dV_lps_4_1_u16.DataTypeMode = 'Fixed-point: slope and bias scaling';
  | T_dV_lps_4_1_u16.SignednessBool = false;
  | T_dV_lps_4_1_u16.WordLength = 16;
  | T_dV_lps_4_1_u16.FixedExponent = -2;
  | T_dV_lps_4_1_u16.SlopeAdjustmentFactor = 1;
  | T_dV_lps_4_1_u16.Bias = 0;
  | T_dV_lps_4_1_u16.DataTypeOverride = 'Inherit';
  | T_dV_lps_4_1_u16.IsAlias = true;
  | 
  | T_dV_lps_Float32 = Simulink.NumericType;
  | T_dV_lps_Float32.Description = 'lps (liters / second  (l/s))';
  | if (tmpVer > 7.11)
  | 	T_dV_lps_Float32.DataScope = 'Auto';
  | end
  | T_dV_lps_Float32.HeaderFile = 'Rte_Type.h';
  | T_dV_lps_Float32.DataTypeMode = 'Single';
  | T_dV_lps_Float32.SignednessBool = true;
  | T_dV_lps_Float32.WordLength = 32;
  | T_dV_lps_Float32.FixedExponent = 0;
  | T_dV_lps_Float32.SlopeAdjustmentFactor = 1;
  | T_dV_lps_Float32.Bias = 0;
  | T_dV_lps_Float32.DataTypeOverride = 'Inherit';
  | T_dV_lps_Float32.IsAlias = true;
  | 
  | T_dV_mlps_1024_1_s16 = Simulink.NumericType;
  | T_dV_mlps_1024_1_s16.Description = ['mlps (milliliters / second  (ml/s)' ...
  |                                     ')'];
  | if (tmpVer > 7.11)
  | 	T_dV_mlps_1024_1_s16.DataScope = 'Auto';
  | end
  | T_dV_mlps_1024_1_s16.HeaderFile = 'Rte_Type.h';
  | T_dV_mlps_1024_1_s16.DataTypeMode = ...
  |   'Fixed-point: slope and bias scaling';
  | T_dV_mlps_1024_1_s16.SignednessBool = true;
  | T_dV_mlps_1024_1_s16.WordLength = 16;
  | T_dV_mlps_1024_1_s16.FixedExponent = -10;
  | T_dV_mlps_1024_1_s16.SlopeAdjustmentFactor = 1;
  | T_dV_mlps_1024_1_s16.Bias = 0;
  | T_dV_mlps_1024_1_s16.DataTypeOverride = 'Inherit';
  | T_dV_mlps_1024_1_s16.IsAlias = true;
  | 
  | T_dV_mlps_Float32 = Simulink.NumericType;
  | T_dV_mlps_Float32.Description = 'mlps (milliliters / second  (ml/s))';
  | if (tmpVer > 7.11)
  | 	T_dV_mlps_Float32.DataScope = 'Auto';
  | end
  | T_dV_mlps_Float32.HeaderFile = 'Rte_Type.h';
  | T_dV_mlps_Float32.DataTypeMode = 'Single';
  | T_dV_mlps_Float32.SignednessBool = true;
  | T_dV_mlps_Float32.WordLength = 32;
  | T_dV_mlps_Float32.FixedExponent = 0;
  | T_dV_mlps_Float32.SlopeAdjustmentFactor = 1;
  | T_dV_mlps_Float32.Bias = 0;
  | T_dV_mlps_Float32.DataTypeOverride = 'Inherit';
  | T_dV_mlps_Float32.IsAlias = true;
  | 
  | T_d_BitField16 = Simulink.NumericType;
  | T_d_BitField16.Description = 'BitField';
  | if (tmpVer > 7.11)
  | 	T_d_BitField16.DataScope = 'Auto';
  | end
  | T_d_BitField16.HeaderFile = 'Rte_Type.h';
  | T_d_BitField16.DataTypeMode = 'Fixed-point: slope and bias scaling';
  | T_d_BitField16.SignednessBool = false;
  | T_d_BitField16.WordLength = 16;
  | T_d_BitField16.FixedExponent = 0;
  | T_d_BitField16.SlopeAdjustmentFactor = 1;
  | T_d_BitField16.Bias = 0;
  | T_d_BitField16.DataTypeOverride = 'Inherit';
  | T_d_BitField16.IsAlias = true;
  | 
  | T_dm_gps_128_1_s16 = Simulink.NumericType;
  | T_dm_gps_128_1_s16.Description = 'gps (grams / second  (g/s))';
  | if (tmpVer > 7.11)
  | 	T_dm_gps_128_1_s16.DataScope = 'Auto';
  | end
  | T_dm_gps_128_1_s16.HeaderFile = 'Rte_Type.h';
  | T_dm_gps_128_1_s16.DataTypeMode = 'Fixed-point: slope and bias scaling';
  | T_dm_gps_128_1_s16.SignednessBool = true;
  | T_dm_gps_128_1_s16.WordLength = 16;
  | T_dm_gps_128_1_s16.FixedExponent = -7;
  | T_dm_gps_128_1_s16.SlopeAdjustmentFactor = 1;
  | T_dm_gps_128_1_s16.Bias = 0;
  | T_dm_gps_128_1_s16.DataTypeOverride = 'Inherit';
  | T_dm_gps_128_1_s16.IsAlias = true;
  | 
  | T_dm_gps_128_1_u16 = Simulink.NumericType;
  | T_dm_gps_128_1_u16.Description = 'gps (grams / second  (g/s))';
  | if (tmpVer > 7.11)
  | 	T_dm_gps_128_1_u16.DataScope = 'Auto';
  | end
  | T_dm_gps_128_1_u16.HeaderFile = 'Rte_Type.h';
  | T_dm_gps_128_1_u16.DataTypeMode = 'Fixed-point: slope and bias scaling';
  | T_dm_gps_128_1_u16.SignednessBool = false;
  | T_dm_gps_128_1_u16.WordLength = 16;
  | T_dm_gps_128_1_u16.FixedExponent = -7;
  | T_dm_gps_128_1_u16.SlopeAdjustmentFactor = 1;
  | T_dm_gps_128_1_u16.Bias = 0;
  | T_dm_gps_128_1_u16.DataTypeOverride = 'Inherit';
  | T_dm_gps_128_1_u16.IsAlias = true;
  | 
  | T_dm_gps_256_1_u16 = Simulink.NumericType;
  | T_dm_gps_256_1_u16.Description = 'gps (grams / second  (g/s))';
  | if (tmpVer > 7.11)
  | 	T_dm_gps_256_1_u16.DataScope = 'Auto';
  | end
  | T_dm_gps_256_1_u16.HeaderFile = 'Rte_Type.h';
  | T_dm_gps_256_1_u16.DataTypeMode = 'Fixed-point: slope and bias scaling';
  | T_dm_gps_256_1_u16.SignednessBool = false;
  | T_dm_gps_256_1_u16.WordLength = 16;
  | T_dm_gps_256_1_u16.FixedExponent = -8;
  | T_dm_gps_256_1_u16.SlopeAdjustmentFactor = 1;
  | T_dm_gps_256_1_u16.Bias = 0;
  | T_dm_gps_256_1_u16.DataTypeOverride = 'Inherit';
  | T_dm_gps_256_1_u16.IsAlias = true;
  | 
  | T_dm_gps_Float32 = Simulink.NumericType;
  | T_dm_gps_Float32.Description = 'gps (grams / second  (g/s))';
  | if (tmpVer > 7.11)
  | 	T_dm_gps_Float32.DataScope = 'Auto';
  | end
  | T_dm_gps_Float32.HeaderFile = 'Rte_Type.h';
  | T_dm_gps_Float32.DataTypeMode = 'Single';
  | T_dm_gps_Float32.SignednessBool = true;
  | T_dm_gps_Float32.WordLength = 32;
  | T_dm_gps_Float32.FixedExponent = 0;
  | T_dm_gps_Float32.SlopeAdjustmentFactor = 1;
  | T_dm_gps_Float32.Bias = 0;
  | T_dm_gps_Float32.DataTypeOverride = 'Inherit';
  | T_dm_gps_Float32.IsAlias = true;
  | 
  | T_dm_mgps_1_1_s16 = Simulink.NumericType;
  | T_dm_mgps_1_1_s16.Description = 'mgps (milligrams / second  (mg/s))';
  | if (tmpVer > 7.11)
  | 	T_dm_mgps_1_1_s16.DataScope = 'Auto';
  | end
  | T_dm_mgps_1_1_s16.HeaderFile = 'Rte_Type.h';
  | T_dm_mgps_1_1_s16.DataTypeMode = 'Fixed-point: slope and bias scaling';
  | T_dm_mgps_1_1_s16.SignednessBool = true;
  | T_dm_mgps_1_1_s16.WordLength = 16;
  | T_dm_mgps_1_1_s16.FixedExponent = 0;
  | T_dm_mgps_1_1_s16.SlopeAdjustmentFactor = 1;
  | T_dm_mgps_1_1_s16.Bias = 0;
  | T_dm_mgps_1_1_s16.DataTypeOverride = 'Inherit';
  | T_dm_mgps_1_1_s16.IsAlias = true;
  | 
  | T_dm_mgps_Float32 = Simulink.NumericType;
  | T_dm_mgps_Float32.Description = 'mgps (milligrams / second  (mg/s))';
  | if (tmpVer > 7.11)
  | 	T_dm_mgps_Float32.DataScope = 'Auto';
  | end
  | T_dm_mgps_Float32.HeaderFile = 'Rte_Type.h';
  | T_dm_mgps_Float32.DataTypeMode = 'Single';
  | T_dm_mgps_Float32.SignednessBool = true;
  | T_dm_mgps_Float32.WordLength = 32;
  | T_dm_mgps_Float32.FixedExponent = 0;
  | T_dm_mgps_Float32.SlopeAdjustmentFactor = 1;
  | T_dm_mgps_Float32.Bias = 0;
  | T_dm_mgps_Float32.DataTypeOverride = 'Inherit';
  | T_dm_mgps_Float32.IsAlias = true;
  | 
  | T_dn_rpmps_1_1_s16 = Simulink.NumericType;
  | T_dn_rpmps_1_1_s16.Description = ['rpmps (revolutions / minute / second' ...
  |                                   '  (rpm/s))'];
  | if (tmpVer > 7.11)
  | 	T_dn_rpmps_1_1_s16.DataScope = 'Auto';
  | end
  | T_dn_rpmps_1_1_s16.HeaderFile = 'Rte_Type.h';
  | T_dn_rpmps_1_1_s16.DataTypeMode = 'Fixed-point: slope and bias scaling';
  | T_dn_rpmps_1_1_s16.SignednessBool = true;
  | T_dn_rpmps_1_1_s16.WordLength = 16;
  | T_dn_rpmps_1_1_s16.FixedExponent = 0;
  | T_dn_rpmps_1_1_s16.SlopeAdjustmentFactor = 1;
  | T_dn_rpmps_1_1_s16.Bias = 0;
  | T_dn_rpmps_1_1_s16.DataTypeOverride = 'Inherit';
  | T_dn_rpmps_1_1_s16.IsAlias = true;
  | 
  | T_dn_rpmps_2_1_s16 = Simulink.NumericType;
  | T_dn_rpmps_2_1_s16.Description = ['rpmps (revolutions / minute / second' ...
  |                                   '  (rpm/s))'];
  | if (tmpVer > 7.11)
  | 	T_dn_rpmps_2_1_s16.DataScope = 'Auto';
  | end
  | T_dn_rpmps_2_1_s16.HeaderFile = 'Rte_Type.h';
  | T_dn_rpmps_2_1_s16.DataTypeMode = 'Fixed-point: slope and bias scaling';
  | T_dn_rpmps_2_1_s16.SignednessBool = true;
  | T_dn_rpmps_2_1_s16.WordLength = 16;
  | T_dn_rpmps_2_1_s16.FixedExponent = -1;
  | T_dn_rpmps_2_1_s16.SlopeAdjustmentFactor = 1;
  | T_dn_rpmps_2_1_s16.Bias = 0;
  | T_dn_rpmps_2_1_s16.DataTypeOverride = 'Inherit';
  | T_dn_rpmps_2_1_s16.IsAlias = true;
  | 
  | T_dn_rpmps_Float32 = Simulink.NumericType;
  | T_dn_rpmps_Float32.Description = ['rpmps (revolutions / minute / second' ...
  |                                   '  (rpm/s))'];
  | if (tmpVer > 7.11)
  | 	T_dn_rpmps_Float32.DataScope = 'Auto';
  | end
  | T_dn_rpmps_Float32.HeaderFile = 'Rte_Type.h';
  | T_dn_rpmps_Float32.DataTypeMode = 'Single';
  | T_dn_rpmps_Float32.SignednessBool = true;
  | T_dn_rpmps_Float32.WordLength = 32;
  | T_dn_rpmps_Float32.FixedExponent = 0;
  | T_dn_rpmps_Float32.SlopeAdjustmentFactor = 1;
  | T_dn_rpmps_Float32.Bias = 0;
  | T_dn_rpmps_Float32.DataTypeOverride = 'Inherit';
  | T_dn_rpmps_Float32.IsAlias = true;
  | 
  | T_dp_Paps_1_1_s16 = Simulink.NumericType;
  | T_dp_Paps_1_1_s16.Description = 'Paps (Pascals / second  (Pa/s))';
  | if (tmpVer > 7.11)
  | 	T_dp_Paps_1_1_s16.DataScope = 'Auto';
  | end
  | T_dp_Paps_1_1_s16.HeaderFile = 'Rte_Type.h';
  | T_dp_Paps_1_1_s16.DataTypeMode = 'Fixed-point: slope and bias scaling';
  | T_dp_Paps_1_1_s16.SignednessBool = true;
  | T_dp_Paps_1_1_s16.WordLength = 16;
  | T_dp_Paps_1_1_s16.FixedExponent = 0;
  | T_dp_Paps_1_1_s16.SlopeAdjustmentFactor = 1;
  | T_dp_Paps_1_1_s16.Bias = 0;
  | T_dp_Paps_1_1_s16.DataTypeOverride = 'Inherit';
  | T_dp_Paps_1_1_s16.IsAlias = true;
  | 
  | T_dp_Paps_Float32 = Simulink.NumericType;
  | T_dp_Paps_Float32.Description = 'Paps (Pascals / second  (Pa/s))';
  | if (tmpVer > 7.11)
  | 	T_dp_Paps_Float32.DataScope = 'Auto';
  | end
  | T_dp_Paps_Float32.HeaderFile = 'Rte_Type.h';
  | T_dp_Paps_Float32.DataTypeMode = 'Single';
  | T_dp_Paps_Float32.SignednessBool = true;
  | T_dp_Paps_Float32.WordLength = 32;
  | T_dp_Paps_Float32.FixedExponent = 0;
  | T_dp_Paps_Float32.SlopeAdjustmentFactor = 1;
  | T_dp_Paps_Float32.Bias = 0;
  | T_dp_Paps_Float32.DataTypeOverride = 'Inherit';
  | T_dp_Paps_Float32.IsAlias = true;
  | 
  | T_dp_kPaps_1_1_s16 = Simulink.NumericType;
  | T_dp_kPaps_1_1_s16.Description = ['kPaps (kiloPascals / second  (kPa/s)' ...
  |                                   ')'];
  | if (tmpVer > 7.11)
  | 	T_dp_kPaps_1_1_s16.DataScope = 'Auto';
  | end
  | T_dp_kPaps_1_1_s16.HeaderFile = 'Rte_Type.h';
  | T_dp_kPaps_1_1_s16.DataTypeMode = 'Fixed-point: slope and bias scaling';
  | T_dp_kPaps_1_1_s16.SignednessBool = true;
  | T_dp_kPaps_1_1_s16.WordLength = 16;
  | T_dp_kPaps_1_1_s16.FixedExponent = 0;
  | T_dp_kPaps_1_1_s16.SlopeAdjustmentFactor = 1;
  | T_dp_kPaps_1_1_s16.Bias = 0;
  | T_dp_kPaps_1_1_s16.DataTypeOverride = 'Inherit';
  | T_dp_kPaps_1_1_s16.IsAlias = true;
  | 
  | T_dp_kPaps_8_1_s16 = Simulink.NumericType;
  | T_dp_kPaps_8_1_s16.Description = ['kPaps (kiloPascals / second  (kPa/s)' ...
  |                                   ')'];
  | if (tmpVer > 7.11)
  | 	T_dp_kPaps_8_1_s16.DataScope = 'Auto';
  | end
  | T_dp_kPaps_8_1_s16.HeaderFile = 'Rte_Type.h';
  | T_dp_kPaps_8_1_s16.DataTypeMode = 'Fixed-point: slope and bias scaling';
  | T_dp_kPaps_8_1_s16.SignednessBool = true;
  | T_dp_kPaps_8_1_s16.WordLength = 16;
  | T_dp_kPaps_8_1_s16.FixedExponent = -3;
  | T_dp_kPaps_8_1_s16.SlopeAdjustmentFactor = 1;
  | T_dp_kPaps_8_1_s16.Bias = 0;
  | T_dp_kPaps_8_1_s16.DataTypeOverride = 'Inherit';
  | T_dp_kPaps_8_1_s16.IsAlias = true;
  | 
  | T_dp_kPaps_Float32 = Simulink.NumericType;
  | T_dp_kPaps_Float32.Description = ['kPaps (kiloPascals / second  (kPa/s)' ...
  |                                   ')'];
  | if (tmpVer > 7.11)
  | 	T_dp_kPaps_Float32.DataScope = 'Auto';
  | end
  | T_dp_kPaps_Float32.HeaderFile = 'Rte_Type.h';
  | T_dp_kPaps_Float32.DataTypeMode = 'Single';
  | T_dp_kPaps_Float32.SignednessBool = true;
  | T_dp_kPaps_Float32.WordLength = 32;
  | T_dp_kPaps_Float32.FixedExponent = 0;
  | T_dp_kPaps_Float32.SlopeAdjustmentFactor = 1;
  | T_dp_kPaps_Float32.Bias = 0;
  | T_dp_kPaps_Float32.DataTypeOverride = 'Inherit';
  | T_dp_kPaps_Float32.IsAlias = true;
  | 
  | T_dphi_degps_128_1_s16 = Simulink.NumericType;
  | T_dphi_degps_128_1_s16.Description = ...
  |   'degps (degrees / second  (deg/s))';
  | if (tmpVer > 7.11)
  | 	T_dphi_degps_128_1_s16.DataScope = 'Auto';
  | end
  | T_dphi_degps_128_1_s16.HeaderFile = 'Rte_Type.h';
  | T_dphi_degps_128_1_s16.DataTypeMode = ...
  |   'Fixed-point: slope and bias scaling';
  | T_dphi_degps_128_1_s16.SignednessBool = true;
  | T_dphi_degps_128_1_s16.WordLength = 16;
  | T_dphi_degps_128_1_s16.FixedExponent = -7;
  | T_dphi_degps_128_1_s16.SlopeAdjustmentFactor = 1;
  | T_dphi_degps_128_1_s16.Bias = 0;
  | T_dphi_degps_128_1_s16.DataTypeOverride = 'Inherit';
  | T_dphi_degps_128_1_s16.IsAlias = true;
  | 
  | T_dphi_degps_8_1_s16 = Simulink.NumericType;
  | T_dphi_degps_8_1_s16.Description = 'degps (degrees / second  (deg/s))';
  | if (tmpVer > 7.11)
  | 	T_dphi_degps_8_1_s16.DataScope = 'Auto';
  | end
  | T_dphi_degps_8_1_s16.HeaderFile = 'Rte_Type.h';
  | T_dphi_degps_8_1_s16.DataTypeMode = ...
  |   'Fixed-point: slope and bias scaling';
  | T_dphi_degps_8_1_s16.SignednessBool = true;
  | T_dphi_degps_8_1_s16.WordLength = 16;
  | T_dphi_degps_8_1_s16.FixedExponent = -3;
  | T_dphi_degps_8_1_s16.SlopeAdjustmentFactor = 1;
  | T_dphi_degps_8_1_s16.Bias = 0;
  | T_dphi_degps_8_1_s16.DataTypeOverride = 'Inherit';
  | T_dphi_degps_8_1_s16.IsAlias = true;
  | 
  | T_dphi_degps_Float32 = Simulink.NumericType;
  | T_dphi_degps_Float32.Description = 'degps (degrees / second  (deg/s))';
  | if (tmpVer > 7.11)
  | 	T_dphi_degps_Float32.DataScope = 'Auto';
  | end
  | T_dphi_degps_Float32.HeaderFile = 'Rte_Type.h';
  | T_dphi_degps_Float32.DataTypeMode = 'Single';
  | T_dphi_degps_Float32.SignednessBool = true;
  | T_dphi_degps_Float32.WordLength = 32;
  | T_dphi_degps_Float32.FixedExponent = 0;
  | T_dphi_degps_Float32.SlopeAdjustmentFactor = 1;
  | T_dphi_degps_Float32.Bias = 0;
  | T_dphi_degps_Float32.DataTypeOverride = 'Inherit';
  | T_dphi_degps_Float32.IsAlias = true;
  | 
  | T_dr_ps_256_1_s16 = Simulink.NumericType;
  | T_dr_ps_256_1_s16.Description = 'ps (none)';
  | if (tmpVer > 7.11)
  | 	T_dr_ps_256_1_s16.DataScope = 'Auto';
  | end
  | T_dr_ps_256_1_s16.HeaderFile = 'Rte_Type.h';
  | T_dr_ps_256_1_s16.DataTypeMode = 'Fixed-point: slope and bias scaling';
  | T_dr_ps_256_1_s16.SignednessBool = true;
  | T_dr_ps_256_1_s16.WordLength = 16;
  | T_dr_ps_256_1_s16.FixedExponent = -8;
  | T_dr_ps_256_1_s16.SlopeAdjustmentFactor = 1;
  | T_dr_ps_256_1_s16.Bias = 0;
  | T_dr_ps_256_1_s16.DataTypeOverride = 'Inherit';
  | T_dr_ps_256_1_s16.IsAlias = true;
  | 
  | T_dr_ps_Float32 = Simulink.NumericType;
  | T_dr_ps_Float32.Description = 'ps (none)';
  | if (tmpVer > 7.11)
  | 	T_dr_ps_Float32.DataScope = 'Auto';
  | end
  | T_dr_ps_Float32.HeaderFile = 'Rte_Type.h';
  | T_dr_ps_Float32.DataTypeMode = 'Single';
  | T_dr_ps_Float32.SignednessBool = true;
  | T_dr_ps_Float32.WordLength = 32;
  | T_dr_ps_Float32.FixedExponent = 0;
  | T_dr_ps_Float32.SlopeAdjustmentFactor = 1;
  | T_dr_ps_Float32.Bias = 0;
  | T_dr_ps_Float32.DataTypeOverride = 'Inherit';
  | T_dr_ps_Float32.IsAlias = true;
  | 
  | T_drho_mgplps_1_2_s16 = Simulink.NumericType;
  | T_drho_mgplps_1_2_s16.Description = ...
  |   'mgplps (milligrams / liter / s (mg/l/s))';
  | if (tmpVer > 7.11)
  | 	T_drho_mgplps_1_2_s16.DataScope = 'Auto';
  | end
  | T_drho_mgplps_1_2_s16.HeaderFile = 'Rte_Type.h';
  | T_drho_mgplps_1_2_s16.DataTypeMode = ...
  |   'Fixed-point: slope and bias scaling';
  | T_drho_mgplps_1_2_s16.SignednessBool = true;
  | T_drho_mgplps_1_2_s16.WordLength = 16;
  | T_drho_mgplps_1_2_s16.FixedExponent = 1;
  | T_drho_mgplps_1_2_s16.SlopeAdjustmentFactor = 1;
  | T_drho_mgplps_1_2_s16.Bias = 0;
  | T_drho_mgplps_1_2_s16.DataTypeOverride = 'Inherit';
  | T_drho_mgplps_1_2_s16.IsAlias = true;
  | 
  | T_drho_mgplps_Float32 = Simulink.NumericType;
  | T_drho_mgplps_Float32.Description = ...
  |   'mgplps (milligrams / liter / s (mg/l/s))';
  | if (tmpVer > 7.11)
  | 	T_drho_mgplps_Float32.DataScope = 'Auto';
  | end
  | T_drho_mgplps_Float32.HeaderFile = 'Rte_Type.h';
  | T_drho_mgplps_Float32.DataTypeMode = 'Single';
  | T_drho_mgplps_Float32.SignednessBool = true;
  | T_drho_mgplps_Float32.WordLength = 32;
  | T_drho_mgplps_Float32.FixedExponent = 0;
  | T_drho_mgplps_Float32.SlopeAdjustmentFactor = 1;
  | T_drho_mgplps_Float32.Bias = 0;
  | T_drho_mgplps_Float32.DataTypeOverride = 'Inherit';
  | T_drho_mgplps_Float32.IsAlias = true;
  | 
  | T_e_NA_1_1_u8 = Simulink.NumericType;
  | T_e_NA_1_1_u8.Description = 'TYPE TO BE REMOVED';
  | if (tmpVer > 7.11)
  | 	T_e_NA_1_1_u8.DataScope = 'Auto';
  | end
  | T_e_NA_1_1_u8.HeaderFile = 'Rte_Type.h';
  | T_e_NA_1_1_u8.DataTypeMode = 'Fixed-point: slope and bias scaling';
  | T_e_NA_1_1_u8.SignednessBool = false;
  | T_e_NA_1_1_u8.WordLength = 8;
  | T_e_NA_1_1_u8.FixedExponent = 0;
  | T_e_NA_1_1_u8.SlopeAdjustmentFactor = 1;
  | T_e_NA_1_1_u8.Bias = 0;
  | T_e_NA_1_1_u8.DataTypeOverride = 'Inherit';
  | T_e_NA_1_1_u8.IsAlias = true;
  | 
  | T_f_Hz_1_1_u16 = Simulink.NumericType;
  | T_f_Hz_1_1_u16.Description = 'Hz (hertz  (Hz))';
  | if (tmpVer > 7.11)
  | 	T_f_Hz_1_1_u16.DataScope = 'Auto';
  | end
  | T_f_Hz_1_1_u16.HeaderFile = 'Rte_Type.h';
  | T_f_Hz_1_1_u16.DataTypeMode = 'Fixed-point: slope and bias scaling';
  | T_f_Hz_1_1_u16.SignednessBool = false;
  | T_f_Hz_1_1_u16.WordLength = 16;
  | T_f_Hz_1_1_u16.FixedExponent = 0;
  | T_f_Hz_1_1_u16.SlopeAdjustmentFactor = 1;
  | T_f_Hz_1_1_u16.Bias = 0;
  | T_f_Hz_1_1_u16.DataTypeOverride = 'Inherit';
  | T_f_Hz_1_1_u16.IsAlias = true;
  | 
  | T_f_Hz_1_1_u32 = Simulink.NumericType;
  | T_f_Hz_1_1_u32.Description = 'Hz (hertz  (Hz))';
  | if (tmpVer > 7.11)
  | 	T_f_Hz_1_1_u32.DataScope = 'Auto';
  | end
  | T_f_Hz_1_1_u32.HeaderFile = 'Rte_Type.h';
  | T_f_Hz_1_1_u32.DataTypeMode = 'Fixed-point: slope and bias scaling';
  | T_f_Hz_1_1_u32.SignednessBool = false;
  | T_f_Hz_1_1_u32.WordLength = 32;
  | T_f_Hz_1_1_u32.FixedExponent = 0;
  | T_f_Hz_1_1_u32.SlopeAdjustmentFactor = 1;
  | T_f_Hz_1_1_u32.Bias = 0;
  | T_f_Hz_1_1_u32.DataTypeOverride = 'Inherit';
  | T_f_Hz_1_1_u32.IsAlias = true;
  | 
  | T_f_Hz_64_1_u16 = Simulink.NumericType;
  | T_f_Hz_64_1_u16.Description = 'Hz (hertz  (Hz))';
  | if (tmpVer > 7.11)
  | 	T_f_Hz_64_1_u16.DataScope = 'Auto';
  | end
  | T_f_Hz_64_1_u16.HeaderFile = 'Rte_Type.h';
  | T_f_Hz_64_1_u16.DataTypeMode = 'Fixed-point: slope and bias scaling';
  | T_f_Hz_64_1_u16.SignednessBool = false;
  | T_f_Hz_64_1_u16.WordLength = 16;
  | T_f_Hz_64_1_u16.FixedExponent = -6;
  | T_f_Hz_64_1_u16.SlopeAdjustmentFactor = 1;
  | T_f_Hz_64_1_u16.Bias = 0;
  | T_f_Hz_64_1_u16.DataTypeOverride = 'Inherit';
  | T_f_Hz_64_1_u16.IsAlias = true;
  | 
  | T_f_Hz_8_1_s16 = Simulink.NumericType;
  | T_f_Hz_8_1_s16.Description = 'Hz (hertz  (Hz))';
  | if (tmpVer > 7.11)
  | 	T_f_Hz_8_1_s16.DataScope = 'Auto';
  | end
  | T_f_Hz_8_1_s16.HeaderFile = 'Rte_Type.h';
  | T_f_Hz_8_1_s16.DataTypeMode = 'Fixed-point: slope and bias scaling';
  | T_f_Hz_8_1_s16.SignednessBool = true;
  | T_f_Hz_8_1_s16.WordLength = 16;
  | T_f_Hz_8_1_s16.FixedExponent = -3;
  | T_f_Hz_8_1_s16.SlopeAdjustmentFactor = 1;
  | T_f_Hz_8_1_s16.Bias = 0;
  | T_f_Hz_8_1_s16.DataTypeOverride = 'Inherit';
  | T_f_Hz_8_1_s16.IsAlias = true;
  | 
  | T_f_Hz_Float32 = Simulink.NumericType;
  | T_f_Hz_Float32.Description = 'Hz (hertz  (Hz))';
  | if (tmpVer > 7.11)
  | 	T_f_Hz_Float32.DataScope = 'Auto';
  | end
  | T_f_Hz_Float32.HeaderFile = 'Rte_Type.h';
  | T_f_Hz_Float32.DataTypeMode = 'Single';
  | T_f_Hz_Float32.SignednessBool = true;
  | T_f_Hz_Float32.WordLength = 32;
  | T_f_Hz_Float32.FixedExponent = 0;
  | T_f_Hz_Float32.SlopeAdjustmentFactor = 1;
  | T_f_Hz_Float32.Bias = 0;
  | T_f_Hz_Float32.DataTypeOverride = 'Inherit';
  | T_f_Hz_Float32.IsAlias = true;
  | 
  | T_g_BitField32 = Simulink.NumericType;
  | T_g_BitField32.Description = 'BitField';
  | if (tmpVer > 7.11)
  | 	T_g_BitField32.DataScope = 'Auto';
  | end
  | T_g_BitField32.HeaderFile = 'Rte_Type.h';
  | T_g_BitField32.DataTypeMode = 'Fixed-point: slope and bias scaling';
  | T_g_BitField32.SignednessBool = false;
  | T_g_BitField32.WordLength = 32;
  | T_g_BitField32.FixedExponent = 0;
  | T_g_BitField32.SlopeAdjustmentFactor = 1;
  | T_g_BitField32.Bias = 0;
  | T_g_BitField32.DataTypeOverride = 'Inherit';
  | T_g_BitField32.IsAlias = true;
  | 
  | T_l_km_16_1_s16 = Simulink.NumericType;
  | T_l_km_16_1_s16.Description = 'km (kilometers  (km))';
  | if (tmpVer > 7.11)
  | 	T_l_km_16_1_s16.DataScope = 'Auto';
  | end
  | T_l_km_16_1_s16.HeaderFile = 'Rte_Type.h';
  | T_l_km_16_1_s16.DataTypeMode = 'Fixed-point: slope and bias scaling';
  | T_l_km_16_1_s16.SignednessBool = true;
  | T_l_km_16_1_s16.WordLength = 16;
  | T_l_km_16_1_s16.FixedExponent = -4;
  | T_l_km_16_1_s16.SlopeAdjustmentFactor = 1;
  | T_l_km_16_1_s16.Bias = 0;
  | T_l_km_16_1_s16.DataTypeOverride = 'Inherit';
  | T_l_km_16_1_s16.IsAlias = true;
  | 
  | T_l_km_1_1_u16 = Simulink.NumericType;
  | T_l_km_1_1_u16.Description = 'km (kilometers  (km))';
  | if (tmpVer > 7.11)
  | 	T_l_km_1_1_u16.DataScope = 'Auto';
  | end
  | T_l_km_1_1_u16.HeaderFile = 'Rte_Type.h';
  | T_l_km_1_1_u16.DataTypeMode = 'Fixed-point: slope and bias scaling';
  | T_l_km_1_1_u16.SignednessBool = false;
  | T_l_km_1_1_u16.WordLength = 16;
  | T_l_km_1_1_u16.FixedExponent = 0;
  | T_l_km_1_1_u16.SlopeAdjustmentFactor = 1;
  | T_l_km_1_1_u16.Bias = 0;
  | T_l_km_1_1_u16.DataTypeOverride = 'Inherit';
  | T_l_km_1_1_u16.IsAlias = true;
  | 
  | T_l_km_1_1_u32 = Simulink.NumericType;
  | T_l_km_1_1_u32.Description = 'km (kilometers  (km))';
  | if (tmpVer > 7.11)
  | 	T_l_km_1_1_u32.DataScope = 'Auto';
  | end
  | T_l_km_1_1_u32.HeaderFile = 'Rte_Type.h';
  | T_l_km_1_1_u32.DataTypeMode = 'Fixed-point: slope and bias scaling';
  | T_l_km_1_1_u32.SignednessBool = false;
  | T_l_km_1_1_u32.WordLength = 32;
  | T_l_km_1_1_u32.FixedExponent = 0;
  | T_l_km_1_1_u32.SlopeAdjustmentFactor = 1;
  | T_l_km_1_1_u32.Bias = 0;
  | T_l_km_1_1_u32.DataTypeOverride = 'Inherit';
  | T_l_km_1_1_u32.IsAlias = true;
  | 
  | T_l_km_Float32 = Simulink.NumericType;
  | T_l_km_Float32.Description = 'km (kilometers  (km))';
  | if (tmpVer > 7.11)
  | 	T_l_km_Float32.DataScope = 'Auto';
  | end
  | T_l_km_Float32.HeaderFile = 'Rte_Type.h';
  | T_l_km_Float32.DataTypeMode = 'Single';
  | T_l_km_Float32.SignednessBool = true;
  | T_l_km_Float32.WordLength = 32;
  | T_l_km_Float32.FixedExponent = 0;
  | T_l_km_Float32.SlopeAdjustmentFactor = 1;
  | T_l_km_Float32.Bias = 0;
  | T_l_km_Float32.DataTypeOverride = 'Inherit';
  | T_l_km_Float32.IsAlias = true;
  | 
  | T_l_m_1024_1_s16 = Simulink.NumericType;
  | T_l_m_1024_1_s16.Description = 'm (meters  (m))';
  | if (tmpVer > 7.11)
  | 	T_l_m_1024_1_s16.DataScope = 'Auto';
  | end
  | T_l_m_1024_1_s16.HeaderFile = 'Rte_Type.h';
  | T_l_m_1024_1_s16.DataTypeMode = 'Fixed-point: slope and bias scaling';
  | T_l_m_1024_1_s16.SignednessBool = true;
  | T_l_m_1024_1_s16.WordLength = 16;
  | T_l_m_1024_1_s16.FixedExponent = -10;
  | T_l_m_1024_1_s16.SlopeAdjustmentFactor = 1;
  | T_l_m_1024_1_s16.Bias = 0;
  | T_l_m_1024_1_s16.DataTypeOverride = 'Inherit';
  | T_l_m_1024_1_s16.IsAlias = true;
  | 
  | T_l_m_16_1_s16 = Simulink.NumericType;
  | T_l_m_16_1_s16.Description = 'm (meters  (m))';
  | if (tmpVer > 7.11)
  | 	T_l_m_16_1_s16.DataScope = 'Auto';
  | end
  | T_l_m_16_1_s16.HeaderFile = 'Rte_Type.h';
  | T_l_m_16_1_s16.DataTypeMode = 'Fixed-point: slope and bias scaling';
  | T_l_m_16_1_s16.SignednessBool = true;
  | T_l_m_16_1_s16.WordLength = 16;
  | T_l_m_16_1_s16.FixedExponent = -4;
  | T_l_m_16_1_s16.SlopeAdjustmentFactor = 1;
  | T_l_m_16_1_s16.Bias = 0;
  | T_l_m_16_1_s16.DataTypeOverride = 'Inherit';
  | T_l_m_16_1_s16.IsAlias = true;
  | 
  | T_l_m_1_1_u32 = Simulink.NumericType;
  | T_l_m_1_1_u32.Description = 'm (meters  (m))';
  | if (tmpVer > 7.11)
  | 	T_l_m_1_1_u32.DataScope = 'Auto';
  | end
  | T_l_m_1_1_u32.HeaderFile = 'Rte_Type.h';
  | T_l_m_1_1_u32.DataTypeMode = 'Fixed-point: slope and bias scaling';
  | T_l_m_1_1_u32.SignednessBool = false;
  | T_l_m_1_1_u32.WordLength = 32;
  | T_l_m_1_1_u32.FixedExponent = 0;
  | T_l_m_1_1_u32.SlopeAdjustmentFactor = 1;
  | T_l_m_1_1_u32.Bias = 0;
  | T_l_m_1_1_u32.DataTypeOverride = 'Inherit';
  | T_l_m_1_1_u32.IsAlias = true;
  | 
  | T_l_m_Float32 = Simulink.NumericType;
  | T_l_m_Float32.Description = 'm (meters  (m))';
  | if (tmpVer > 7.11)
  | 	T_l_m_Float32.DataScope = 'Auto';
  | end
  | T_l_m_Float32.HeaderFile = 'Rte_Type.h';
  | T_l_m_Float32.DataTypeMode = 'Single';
  | T_l_m_Float32.SignednessBool = true;
  | T_l_m_Float32.WordLength = 32;
  | T_l_m_Float32.FixedExponent = 0;
  | T_l_m_Float32.SlopeAdjustmentFactor = 1;
  | T_l_m_Float32.Bias = 0;
  | T_l_m_Float32.DataTypeOverride = 'Inherit';
  | T_l_m_Float32.IsAlias = true;
  | 
  | T_l_mm_16_1_s16 = Simulink.NumericType;
  | T_l_mm_16_1_s16.Description = 'mm (millimeters  (mm))';
  | if (tmpVer > 7.11)
  | 	T_l_mm_16_1_s16.DataScope = 'Auto';
  | end
  | T_l_mm_16_1_s16.HeaderFile = 'Rte_Type.h';
  | T_l_mm_16_1_s16.DataTypeMode = 'Fixed-point: slope and bias scaling';
  | T_l_mm_16_1_s16.SignednessBool = true;
  | T_l_mm_16_1_s16.WordLength = 16;
  | T_l_mm_16_1_s16.FixedExponent = -4;
  | T_l_mm_16_1_s16.SlopeAdjustmentFactor = 1;
  | T_l_mm_16_1_s16.Bias = 0;
  | T_l_mm_16_1_s16.DataTypeOverride = 'Inherit';
  | T_l_mm_16_1_s16.IsAlias = true;
  | 
  | T_l_mm_1_1_u16 = Simulink.NumericType;
  | T_l_mm_1_1_u16.Description = 'mm (millimeters  (mm))';
  | if (tmpVer > 7.11)
  | 	T_l_mm_1_1_u16.DataScope = 'Auto';
  | end
  | T_l_mm_1_1_u16.HeaderFile = 'Rte_Type.h';
  | T_l_mm_1_1_u16.DataTypeMode = 'Fixed-point: slope and bias scaling';
  | T_l_mm_1_1_u16.SignednessBool = false;
  | T_l_mm_1_1_u16.WordLength = 16;
  | T_l_mm_1_1_u16.FixedExponent = 0;
  | T_l_mm_1_1_u16.SlopeAdjustmentFactor = 1;
  | T_l_mm_1_1_u16.Bias = 0;
  | T_l_mm_1_1_u16.DataTypeOverride = 'Inherit';
  | T_l_mm_1_1_u16.IsAlias = true;
  | 
  | T_l_mm_4096_1_s16 = Simulink.NumericType;
  | T_l_mm_4096_1_s16.Description = 'mm (millimeters  (mm))';
  | if (tmpVer > 7.11)
  | 	T_l_mm_4096_1_s16.DataScope = 'Auto';
  | end
  | T_l_mm_4096_1_s16.HeaderFile = 'Rte_Type.h';
  | T_l_mm_4096_1_s16.DataTypeMode = 'Fixed-point: slope and bias scaling';
  | T_l_mm_4096_1_s16.SignednessBool = true;
  | T_l_mm_4096_1_s16.WordLength = 16;
  | T_l_mm_4096_1_s16.FixedExponent = -12;
  | T_l_mm_4096_1_s16.SlopeAdjustmentFactor = 1;
  | T_l_mm_4096_1_s16.Bias = 0;
  | T_l_mm_4096_1_s16.DataTypeOverride = 'Inherit';
  | T_l_mm_4096_1_s16.IsAlias = true;
  | 
  | T_l_mm_4_1_u8 = Simulink.NumericType;
  | T_l_mm_4_1_u8.Description = 'mm (millimeters  (mm))';
  | if (tmpVer > 7.11)
  | 	T_l_mm_4_1_u8.DataScope = 'Auto';
  | end
  | T_l_mm_4_1_u8.HeaderFile = 'Rte_Type.h';
  | T_l_mm_4_1_u8.DataTypeMode = 'Fixed-point: slope and bias scaling';
  | T_l_mm_4_1_u8.SignednessBool = false;
  | T_l_mm_4_1_u8.WordLength = 8;
  | T_l_mm_4_1_u8.FixedExponent = -2;
  | T_l_mm_4_1_u8.SlopeAdjustmentFactor = 1;
  | T_l_mm_4_1_u8.Bias = 0;
  | T_l_mm_4_1_u8.DataTypeOverride = 'Inherit';
  | T_l_mm_4_1_u8.IsAlias = true;
  | 
  | T_l_mm_64_1_s16 = Simulink.NumericType;
  | T_l_mm_64_1_s16.Description = 'mm (millimeters  (mm))';
  | if (tmpVer > 7.11)
  | 	T_l_mm_64_1_s16.DataScope = 'Auto';
  | end
  | T_l_mm_64_1_s16.HeaderFile = 'Rte_Type.h';
  | T_l_mm_64_1_s16.DataTypeMode = 'Fixed-point: slope and bias scaling';
  | T_l_mm_64_1_s16.SignednessBool = true;
  | T_l_mm_64_1_s16.WordLength = 16;
  | T_l_mm_64_1_s16.FixedExponent = -6;
  | T_l_mm_64_1_s16.SlopeAdjustmentFactor = 1;
  | T_l_mm_64_1_s16.Bias = 0;
  | T_l_mm_64_1_s16.DataTypeOverride = 'Inherit';
  | T_l_mm_64_1_s16.IsAlias = true;
  | 
  | T_l_mm_Float32 = Simulink.NumericType;
  | T_l_mm_Float32.Description = 'mm (millimeters  (mm))';
  | if (tmpVer > 7.11)
  | 	T_l_mm_Float32.DataScope = 'Auto';
  | end
  | T_l_mm_Float32.HeaderFile = 'Rte_Type.h';
  | T_l_mm_Float32.DataTypeMode = 'Single';
  | T_l_mm_Float32.SignednessBool = true;
  | T_l_mm_Float32.WordLength = 32;
  | T_l_mm_Float32.FixedExponent = 0;
  | T_l_mm_Float32.SlopeAdjustmentFactor = 1;
  | T_l_mm_Float32.Bias = 0;
  | T_l_mm_Float32.DataTypeOverride = 'Inherit';
  | T_l_mm_Float32.IsAlias = true;
  | 
  | T_m_g_1_1_s16 = Simulink.NumericType;
  | T_m_g_1_1_s16.Description = 'g (grams  (g))';
  | if (tmpVer > 7.11)
  | 	T_m_g_1_1_s16.DataScope = 'Auto';
  | end
  | T_m_g_1_1_s16.HeaderFile = 'Rte_Type.h';
  | T_m_g_1_1_s16.DataTypeMode = 'Fixed-point: slope and bias scaling';
  | T_m_g_1_1_s16.SignednessBool = true;
  | T_m_g_1_1_s16.WordLength = 16;
  | T_m_g_1_1_s16.FixedExponent = 0;
  | T_m_g_1_1_s16.SlopeAdjustmentFactor = 1;
  | T_m_g_1_1_s16.Bias = 0;
  | T_m_g_1_1_s16.DataTypeOverride = 'Inherit';
  | T_m_g_1_1_s16.IsAlias = true;
  | 
  | T_m_g_2048_1_s16 = Simulink.NumericType;
  | T_m_g_2048_1_s16.Description = 'g (grams  (g))';
  | if (tmpVer > 7.11)
  | 	T_m_g_2048_1_s16.DataScope = 'Auto';
  | end
  | T_m_g_2048_1_s16.HeaderFile = 'Rte_Type.h';
  | T_m_g_2048_1_s16.DataTypeMode = 'Fixed-point: slope and bias scaling';
  | T_m_g_2048_1_s16.SignednessBool = true;
  | T_m_g_2048_1_s16.WordLength = 16;
  | T_m_g_2048_1_s16.FixedExponent = -11;
  | T_m_g_2048_1_s16.SlopeAdjustmentFactor = 1;
  | T_m_g_2048_1_s16.Bias = 0;
  | T_m_g_2048_1_s16.DataTypeOverride = 'Inherit';
  | T_m_g_2048_1_s16.IsAlias = true;
  | 
  | T_m_g_32_1_u16 = Simulink.NumericType;
  | T_m_g_32_1_u16.Description = 'g (grams  (g))';
  | if (tmpVer > 7.11)
  | 	T_m_g_32_1_u16.DataScope = 'Auto';
  | end
  | T_m_g_32_1_u16.HeaderFile = 'Rte_Type.h';
  | T_m_g_32_1_u16.DataTypeMode = 'Fixed-point: slope and bias scaling';
  | T_m_g_32_1_u16.SignednessBool = false;
  | T_m_g_32_1_u16.WordLength = 16;
  | T_m_g_32_1_u16.FixedExponent = -5;
  | T_m_g_32_1_u16.SlopeAdjustmentFactor = 1;
  | T_m_g_32_1_u16.Bias = 0;
  | T_m_g_32_1_u16.DataTypeOverride = 'Inherit';
  | T_m_g_32_1_u16.IsAlias = true;
  | 
  | T_m_g_Float32 = Simulink.NumericType;
  | T_m_g_Float32.Description = 'g (grams  (g))';
  | if (tmpVer > 7.11)
  | 	T_m_g_Float32.DataScope = 'Auto';
  | end
  | T_m_g_Float32.HeaderFile = 'Rte_Type.h';
  | T_m_g_Float32.DataTypeMode = 'Single';
  | T_m_g_Float32.SignednessBool = true;
  | T_m_g_Float32.WordLength = 32;
  | T_m_g_Float32.FixedExponent = 0;
  | T_m_g_Float32.SlopeAdjustmentFactor = 1;
  | T_m_g_Float32.Bias = 0;
  | T_m_g_Float32.DataTypeOverride = 'Inherit';
  | T_m_g_Float32.IsAlias = true;
  | 
  | T_m_kg_1024_1_s16 = Simulink.NumericType;
  | T_m_kg_1024_1_s16.Description = 'kg (kilograms  (kg))';
  | if (tmpVer > 7.11)
  | 	T_m_kg_1024_1_s16.DataScope = 'Auto';
  | end
  | T_m_kg_1024_1_s16.HeaderFile = 'Rte_Type.h';
  | T_m_kg_1024_1_s16.DataTypeMode = 'Fixed-point: slope and bias scaling';
  | T_m_kg_1024_1_s16.SignednessBool = true;
  | T_m_kg_1024_1_s16.WordLength = 16;
  | T_m_kg_1024_1_s16.FixedExponent = -10;
  | T_m_kg_1024_1_s16.SlopeAdjustmentFactor = 1;
  | T_m_kg_1024_1_s16.Bias = 0;
  | T_m_kg_1024_1_s16.DataTypeOverride = 'Inherit';
  | T_m_kg_1024_1_s16.IsAlias = true;
  | 
  | T_m_kg_1_1_s16 = Simulink.NumericType;
  | T_m_kg_1_1_s16.Description = 'kg (kilograms  (kg))';
  | if (tmpVer > 7.11)
  | 	T_m_kg_1_1_s16.DataScope = 'Auto';
  | end
  | T_m_kg_1_1_s16.HeaderFile = 'Rte_Type.h';
  | T_m_kg_1_1_s16.DataTypeMode = 'Fixed-point: slope and bias scaling';
  | T_m_kg_1_1_s16.SignednessBool = true;
  | T_m_kg_1_1_s16.WordLength = 16;
  | T_m_kg_1_1_s16.FixedExponent = 0;
  | T_m_kg_1_1_s16.SlopeAdjustmentFactor = 1;
  | T_m_kg_1_1_s16.Bias = 0;
  | T_m_kg_1_1_s16.DataTypeOverride = 'Inherit';
  | T_m_kg_1_1_s16.IsAlias = true;
  | 
  | T_m_kg_1_1_u32 = Simulink.NumericType;
  | T_m_kg_1_1_u32.Description = 'kg (kilograms  (kg))';
  | if (tmpVer > 7.11)
  | 	T_m_kg_1_1_u32.DataScope = 'Auto';
  | end
  | T_m_kg_1_1_u32.HeaderFile = 'Rte_Type.h';
  | T_m_kg_1_1_u32.DataTypeMode = 'Fixed-point: slope and bias scaling';
  | T_m_kg_1_1_u32.SignednessBool = false;
  | T_m_kg_1_1_u32.WordLength = 32;
  | T_m_kg_1_1_u32.FixedExponent = 0;
  | T_m_kg_1_1_u32.SlopeAdjustmentFactor = 1;
  | T_m_kg_1_1_u32.Bias = 0;
  | T_m_kg_1_1_u32.DataTypeOverride = 'Inherit';
  | T_m_kg_1_1_u32.IsAlias = true;
  | 
  | T_m_kg_Float32 = Simulink.NumericType;
  | T_m_kg_Float32.Description = 'kg (kilograms  (kg))';
  | if (tmpVer > 7.11)
  | 	T_m_kg_Float32.DataScope = 'Auto';
  | end
  | T_m_kg_Float32.HeaderFile = 'Rte_Type.h';
  | T_m_kg_Float32.DataTypeMode = 'Single';
  | T_m_kg_Float32.SignednessBool = true;
  | T_m_kg_Float32.WordLength = 32;
  | T_m_kg_Float32.FixedExponent = 0;
  | T_m_kg_Float32.SlopeAdjustmentFactor = 1;
  | T_m_kg_Float32.Bias = 0;
  | T_m_kg_Float32.DataTypeOverride = 'Inherit';
  | T_m_kg_Float32.IsAlias = true;
  | 
  | T_m_mg_128_1_s16 = Simulink.NumericType;
  | T_m_mg_128_1_s16.Description = 'mg (milligrams  (mg))';
  | if (tmpVer > 7.11)
  | 	T_m_mg_128_1_s16.DataScope = 'Auto';
  | end
  | T_m_mg_128_1_s16.HeaderFile = 'Rte_Type.h';
  | T_m_mg_128_1_s16.DataTypeMode = 'Fixed-point: slope and bias scaling';
  | T_m_mg_128_1_s16.SignednessBool = true;
  | T_m_mg_128_1_s16.WordLength = 16;
  | T_m_mg_128_1_s16.FixedExponent = -7;
  | T_m_mg_128_1_s16.SlopeAdjustmentFactor = 1;
  | T_m_mg_128_1_s16.Bias = 0;
  | T_m_mg_128_1_s16.DataTypeOverride = 'Inherit';
  | T_m_mg_128_1_s16.IsAlias = true;
  | 
  | T_m_mg_32_1_s16 = Simulink.NumericType;
  | T_m_mg_32_1_s16.Description = 'mg (milligrams  (mg))';
  | if (tmpVer > 7.11)
  | 	T_m_mg_32_1_s16.DataScope = 'Auto';
  | end
  | T_m_mg_32_1_s16.HeaderFile = 'Rte_Type.h';
  | T_m_mg_32_1_s16.DataTypeMode = 'Fixed-point: slope and bias scaling';
  | T_m_mg_32_1_s16.SignednessBool = true;
  | T_m_mg_32_1_s16.WordLength = 16;
  | T_m_mg_32_1_s16.FixedExponent = -5;
  | T_m_mg_32_1_s16.SlopeAdjustmentFactor = 1;
  | T_m_mg_32_1_s16.Bias = 0;
  | T_m_mg_32_1_s16.DataTypeOverride = 'Inherit';
  | T_m_mg_32_1_s16.IsAlias = true;
  | 
  | T_m_mg_Float32 = Simulink.NumericType;
  | T_m_mg_Float32.Description = 'mg (milligrams  (mg))';
  | if (tmpVer > 7.11)
  | 	T_m_mg_Float32.DataScope = 'Auto';
  | end
  | T_m_mg_Float32.HeaderFile = 'Rte_Type.h';
  | T_m_mg_Float32.DataTypeMode = 'Single';
  | T_m_mg_Float32.SignednessBool = true;
  | T_m_mg_Float32.WordLength = 32;
  | T_m_mg_Float32.FixedExponent = 0;
  | T_m_mg_Float32.SlopeAdjustmentFactor = 1;
  | T_m_mg_Float32.Bias = 0;
  | T_m_mg_Float32.DataTypeOverride = 'Inherit';
  | T_m_mg_Float32.IsAlias = true;
  | 
  | T_n_rpm_1_1_s16 = Simulink.NumericType;
  | T_n_rpm_1_1_s16.Description = 'rpm (revolutions / minute  (rpm))';
  | if (tmpVer > 7.11)
  | 	T_n_rpm_1_1_s16.DataScope = 'Auto';
  | end
  | T_n_rpm_1_1_s16.HeaderFile = 'Rte_Type.h';
  | T_n_rpm_1_1_s16.DataTypeMode = 'Fixed-point: slope and bias scaling';
  | T_n_rpm_1_1_s16.SignednessBool = true;
  | T_n_rpm_1_1_s16.WordLength = 16;
  | T_n_rpm_1_1_s16.FixedExponent = 0;
  | T_n_rpm_1_1_s16.SlopeAdjustmentFactor = 1;
  | T_n_rpm_1_1_s16.Bias = 0;
  | T_n_rpm_1_1_s16.DataTypeOverride = 'Inherit';
  | T_n_rpm_1_1_s16.IsAlias = true;
  | 
  | T_n_rpm_1_25_u8 = Simulink.NumericType;
  | T_n_rpm_1_25_u8.Description = 'rpm (revolutions / minute  (rpm))';
  | if (tmpVer > 7.11)
  | 	T_n_rpm_1_25_u8.DataScope = 'Auto';
  | end
  | T_n_rpm_1_25_u8.HeaderFile = 'Rte_Type.h';
  | T_n_rpm_1_25_u8.DataTypeMode = 'Fixed-point: slope and bias scaling';
  | T_n_rpm_1_25_u8.SignednessBool = false;
  | T_n_rpm_1_25_u8.WordLength = 8;
  | T_n_rpm_1_25_u8.FixedExponent = 4;
  | T_n_rpm_1_25_u8.SlopeAdjustmentFactor = 1.5625;
  | T_n_rpm_1_25_u8.Bias = 0;
  | T_n_rpm_1_25_u8.DataTypeOverride = 'Inherit';
  | T_n_rpm_1_25_u8.IsAlias = true;
  | 
  | T_n_rpm_256_50_u16 = Simulink.NumericType;
  | T_n_rpm_256_50_u16.Description = 'rpm (revolutions / minute  (rpm))';
  | if (tmpVer > 7.11)
  | 	T_n_rpm_256_50_u16.DataScope = 'Auto';
  | end
  | T_n_rpm_256_50_u16.HeaderFile = 'Rte_Type.h';
  | T_n_rpm_256_50_u16.DataTypeMode = 'Fixed-point: slope and bias scaling';
  | T_n_rpm_256_50_u16.SignednessBool = false;
  | T_n_rpm_256_50_u16.WordLength = 16;
  | T_n_rpm_256_50_u16.FixedExponent = -3;
  | T_n_rpm_256_50_u16.SlopeAdjustmentFactor = 1.5625;
  | T_n_rpm_256_50_u16.Bias = 0;
  | T_n_rpm_256_50_u16.DataTypeOverride = 'Inherit';
  | T_n_rpm_256_50_u16.IsAlias = true;
  | 
  | T_n_rpm_2_25_u8 = Simulink.NumericType;
  | T_n_rpm_2_25_u8.Description = 'rpm (revolutions / minute  (rpm))';
  | if (tmpVer > 7.11)
  | 	T_n_rpm_2_25_u8.DataScope = 'Auto';
  | end
  | T_n_rpm_2_25_u8.HeaderFile = 'Rte_Type.h';
  | T_n_rpm_2_25_u8.DataTypeMode = 'Fixed-point: slope and bias scaling';
  | T_n_rpm_2_25_u8.SignednessBool = false;
  | T_n_rpm_2_25_u8.WordLength = 8;
  | T_n_rpm_2_25_u8.FixedExponent = 3;
  | T_n_rpm_2_25_u8.SlopeAdjustmentFactor = 1.5625;
  | T_n_rpm_2_25_u8.Bias = 0;
  | T_n_rpm_2_25_u8.DataTypeOverride = 'Inherit';
  | T_n_rpm_2_25_u8.IsAlias = true;
  | 
  | T_n_rpm_4_1_u16 = Simulink.NumericType;
  | T_n_rpm_4_1_u16.Description = 'rpm (revolutions / minute  (rpm))';
  | if (tmpVer > 7.11)
  | 	T_n_rpm_4_1_u16.DataScope = 'Auto';
  | end
  | T_n_rpm_4_1_u16.HeaderFile = 'Rte_Type.h';
  | T_n_rpm_4_1_u16.DataTypeMode = 'Fixed-point: slope and bias scaling';
  | T_n_rpm_4_1_u16.SignednessBool = false;
  | T_n_rpm_4_1_u16.WordLength = 16;
  | T_n_rpm_4_1_u16.FixedExponent = -2;
  | T_n_rpm_4_1_u16.SlopeAdjustmentFactor = 1;
  | T_n_rpm_4_1_u16.Bias = 0;
  | T_n_rpm_4_1_u16.DataTypeOverride = 'Inherit';
  | T_n_rpm_4_1_u16.IsAlias = true;
  | 
  | T_n_rpm_Float32 = Simulink.NumericType;
  | T_n_rpm_Float32.Description = 'rpm (revolutions / minute  (rpm))';
  | if (tmpVer > 7.11)
  | 	T_n_rpm_Float32.DataScope = 'Auto';
  | end
  | T_n_rpm_Float32.HeaderFile = 'Rte_Type.h';
  | T_n_rpm_Float32.DataTypeMode = 'Single';
  | T_n_rpm_Float32.SignednessBool = true;
  | T_n_rpm_Float32.WordLength = 32;
  | T_n_rpm_Float32.FixedExponent = 0;
  | T_n_rpm_Float32.SlopeAdjustmentFactor = 1;
  | T_n_rpm_Float32.Bias = 0;
  | T_n_rpm_Float32.DataTypeOverride = 'Inherit';
  | T_n_rpm_Float32.IsAlias = true;
  | 
  | T_p_MPa_64_1_s16 = Simulink.NumericType;
  | T_p_MPa_64_1_s16.Description = 'MPa (MegaPascals  (MPa))';
  | if (tmpVer > 7.11)
  | 	T_p_MPa_64_1_s16.DataScope = 'Auto';
  | end
  | T_p_MPa_64_1_s16.HeaderFile = 'Rte_Type.h';
  | T_p_MPa_64_1_s16.DataTypeMode = 'Fixed-point: slope and bias scaling';
  | T_p_MPa_64_1_s16.SignednessBool = true;
  | T_p_MPa_64_1_s16.WordLength = 16;
  | T_p_MPa_64_1_s16.FixedExponent = -6;
  | T_p_MPa_64_1_s16.SlopeAdjustmentFactor = 1;
  | T_p_MPa_64_1_s16.Bias = 0;
  | T_p_MPa_64_1_s16.DataTypeOverride = 'Inherit';
  | T_p_MPa_64_1_s16.IsAlias = true;
  | 
  | T_p_MPa_Float32 = Simulink.NumericType;
  | T_p_MPa_Float32.Description = 'MPa (MegaPascals  (MPa))';
  | if (tmpVer > 7.11)
  | 	T_p_MPa_Float32.DataScope = 'Auto';
  | end
  | T_p_MPa_Float32.HeaderFile = 'Rte_Type.h';
  | T_p_MPa_Float32.DataTypeMode = 'Single';
  | T_p_MPa_Float32.SignednessBool = true;
  | T_p_MPa_Float32.WordLength = 32;
  | T_p_MPa_Float32.FixedExponent = 0;
  | T_p_MPa_Float32.SlopeAdjustmentFactor = 1;
  | T_p_MPa_Float32.Bias = 0;
  | T_p_MPa_Float32.DataTypeOverride = 'Inherit';
  | T_p_MPa_Float32.IsAlias = true;
  | 
  | T_p_Pa_1_1_s16 = Simulink.NumericType;
  | T_p_Pa_1_1_s16.Description = 'Pa (Pascals  (Pa))';
  | if (tmpVer > 7.11)
  | 	T_p_Pa_1_1_s16.DataScope = 'Auto';
  | end
  | T_p_Pa_1_1_s16.HeaderFile = 'Rte_Type.h';
  | T_p_Pa_1_1_s16.DataTypeMode = 'Fixed-point: slope and bias scaling';
  | T_p_Pa_1_1_s16.SignednessBool = true;
  | T_p_Pa_1_1_s16.WordLength = 16;
  | T_p_Pa_1_1_s16.FixedExponent = 0;
  | T_p_Pa_1_1_s16.SlopeAdjustmentFactor = 1;
  | T_p_Pa_1_1_s16.Bias = 0;
  | T_p_Pa_1_1_s16.DataTypeOverride = 'Inherit';
  | T_p_Pa_1_1_s16.IsAlias = true;
  | 
  | T_p_Pa_Float32 = Simulink.NumericType;
  | T_p_Pa_Float32.Description = 'Pa (Pascals  (Pa))';
  | if (tmpVer > 7.11)
  | 	T_p_Pa_Float32.DataScope = 'Auto';
  | end
  | T_p_Pa_Float32.HeaderFile = 'Rte_Type.h';
  | T_p_Pa_Float32.DataTypeMode = 'Single';
  | T_p_Pa_Float32.SignednessBool = true;
  | T_p_Pa_Float32.WordLength = 32;
  | T_p_Pa_Float32.FixedExponent = 0;
  | T_p_Pa_Float32.SlopeAdjustmentFactor = 1;
  | T_p_Pa_Float32.Bias = 0;
  | T_p_Pa_Float32.DataTypeOverride = 'Inherit';
  | T_p_Pa_Float32.IsAlias = true;
  | 
  | T_p_kPa_1_10_u16 = Simulink.NumericType;
  | T_p_kPa_1_10_u16.Description = 'kPa (kiloPascals  (kPa))';
  | if (tmpVer > 7.11)
  | 	T_p_kPa_1_10_u16.DataScope = 'Auto';
  | end
  | T_p_kPa_1_10_u16.HeaderFile = 'Rte_Type.h';
  | T_p_kPa_1_10_u16.DataTypeMode = 'Fixed-point: slope and bias scaling';
  | T_p_kPa_1_10_u16.SignednessBool = false;
  | T_p_kPa_1_10_u16.WordLength = 16;
  | T_p_kPa_1_10_u16.FixedExponent = 3;
  | T_p_kPa_1_10_u16.SlopeAdjustmentFactor = 1.25;
  | T_p_kPa_1_10_u16.Bias = 0;
  | T_p_kPa_1_10_u16.DataTypeOverride = 'Inherit';
  | T_p_kPa_1_10_u16.IsAlias = true;
  | 
  | T_p_kPa_1_1_s16 = Simulink.NumericType;
  | T_p_kPa_1_1_s16.Description = 'kPa (kiloPascals  (kPa))';
  | if (tmpVer > 7.11)
  | 	T_p_kPa_1_1_s16.DataScope = 'Auto';
  | end
  | T_p_kPa_1_1_s16.HeaderFile = 'Rte_Type.h';
  | T_p_kPa_1_1_s16.DataTypeMode = 'Fixed-point: slope and bias scaling';
  | T_p_kPa_1_1_s16.SignednessBool = true;
  | T_p_kPa_1_1_s16.WordLength = 16;
  | T_p_kPa_1_1_s16.FixedExponent = 0;
  | T_p_kPa_1_1_s16.SlopeAdjustmentFactor = 1;
  | T_p_kPa_1_1_s16.Bias = 0;
  | T_p_kPa_1_1_s16.DataTypeOverride = 'Inherit';
  | T_p_kPa_1_1_s16.IsAlias = true;
  | 
  | T_p_kPa_1_1_u8 = Simulink.NumericType;
  | T_p_kPa_1_1_u8.Description = 'kPa (kiloPascals  (kPa))';
  | if (tmpVer > 7.11)
  | 	T_p_kPa_1_1_u8.DataScope = 'Auto';
  | end
  | T_p_kPa_1_1_u8.HeaderFile = 'Rte_Type.h';
  | T_p_kPa_1_1_u8.DataTypeMode = 'Fixed-point: slope and bias scaling';
  | T_p_kPa_1_1_u8.SignednessBool = false;
  | T_p_kPa_1_1_u8.WordLength = 8;
  | T_p_kPa_1_1_u8.FixedExponent = 0;
  | T_p_kPa_1_1_u8.SlopeAdjustmentFactor = 1;
